simulink model "deltino"  (R2021b)
(part 8 of 10)

C = ft_4({phi_dot,psi_dot,t10,t100,t1000,t1001,t101,t1010,t1011,t1012,t1013,t1014,t1015,t1016,t1017,t1018,t1019,t102,t1020,t1021,t1022,t1023,t1024,t1025,t1026,t1027,t1028,t1029,t103,t1030,t1031,t1032,t1033,t1038,t1039,t104,t1040,t1041,t1042,t1043,t1044,t1045,t1046,t1047,t1048,t1049,t105,t1054,t1055,t1056,t1057,t1058,t1059,t1060,t1061,t1062,t1063,t1064,t1065,t1066,t1067,t1068,t1069,t1070,t1071,t1072,t1073,t1074,t1075,t1076,t1077,t1079,t1080,t1082,t1083,t1085,t1086,t1088,t1089,t1090,t1091,t1092,t1093,t1094,t1095,t1096,t1097,t1098,t1099,t11,t110,t1100,t1101,t1102,t1103,t1104,t1105,t1106,t1107,t1108,t1109,t111,t1110,t1111,t1112,t1113,t1114,t1115,t1116,t1117,t1118,t1119,t112,t1120,t1121,t1122,t1123,t1124,t1125,t1126,t1127,t1128,t1129,t113,t1130,t1131,t1132,t1133,t1134,t1135,t1136,t1137,t1138,t1139,t114,t1140,t1141,t1142,t1143,t1144,t1145,t1146,t1147,t1148,t1149,t115,t1150,t1151,t1152,t1153,t1154,t1155,t1156,t1157,t1158,t1159,t116,t1160,t1161,t1162,t1163,t1164,t1165,t1166,t1167,t1168,t1169,t117,t1170,t1171,t1172,t1173,t1175,t1176,t1177,t1178,t1179,t118,t1180,t1181,t1182,t1183,t1184,t1185,t1186,t1187,t1188,t119,t1190,t1191,t1193,t1194,t1195,t1196,t1197,t1198,t1199,t12,t120,t1200,t1201,t1202,t1203,t1204,t1205,t1206,t1207,t1208,t1209,t121,t1210,t1211,t1212,t1213,t1214,t122,t1223,t1224,t1225,t123,t1232,t1233,t1234,t1235,t1236,t1237,t1238,t1239,t124,t1240,t1241,t1242,t1243,t1244,t1245,t1246,t1247,t1248,t1249,t125,t1250,t1251,t1252,t1253,t1254,t1255,t1256,t1257,t1258,t1259,t126,t1260,t1261,t1262,t1263,t1264,t1265,t1266,t1267,t1268,t1269,t127,t1270,t1271,t1272,t1273,t1274,t1275,t1276,t1277,t1278,t1279,t128,t1280,t1281,t1282,t1283,t1284,t1285,t1286,t1287,t1288,t1289,t129,t1290,t1291,t1292,t1293,t1294,t1295,t1296,t1297,t1298,t1299,t13,t130,t1300,t1301,t1302,t1303,t1304,t1305,t1306,t1307,t1308,t1309,t131,t1310,t1311,t1312,t1313,t1314,t1315,t1316,t1317,t1318,t1319,t132,t1320,t1321,t1322,t1323,t1324,t1325,t1326,t1327,t1328,t1329,t133,t1330,t1331,t1332,t1335,t1337,t1338,t134,t1340,t1341,t1342,t1343,t1344,t1345,t1346,t1347,t1348,t1349,t135,t1350,t1351,t1352,t1353,t1354,t1355,t1356,t1357,t1358,t1359,t136,t1360,t1361,t1362,t1363,t1364,t1365,t1366,t1367,t1368,t1369,t1370,t1371,t138,t1384,t1385,t1386,t1387,t1388,t1389,t139,t1390,t1391,t1392,t1393,t1394,t1395,t1396,t1397,t1398,t1399,t14,t140,t1400,t1401,t1402,t1403,t1404,t1405,t1406,t1407,t1408,t1409,t141,t1410,t1411,t1412,t1413,t1414,t1415,t1416,t1417,t1418,t1419,t142,t1420,t1421,t1422,t1423,t1424,t1425,t1426,t1427,t1428,t1429,t143,t1430,t1431,t1432,t1433,t1434,t1435,t1436,t1437,t1438,t1439,t144,t1440,t1441,t1442,t1443,t1444,t1445,t1446,t1447,t145,t1458,t1459,t146,t1460,t1461,t1462,t1463,t1464,t1465,t1466,t1467,t1468,t1469,t147,t1470,t1471,t1472,t1473,t1474,t1475,t1476,t1477,t1478,t1479,t148,t1480,t1481,t1482,t1483,t1484,t1485,t1486,t1487,t1488,t1489,t149,t1490,t1491,t1492,t1493,t1494,t1495,t1496,t1497,t1498,t1499,t15,t150,t1501,t1502,t1504,t1505,t1507,t1508,t151,t1510,t1511,t1512,t1513,t1514,t1515,t152,t1524,t1525,t1526,t1527,t1528,t1529,t153,t1530,t1531,t1532,t1533,t1534,t1535,t1536,t1537,t1538,t1539,t154,t1541,t1542,t1543,t1544,t1545,t1546,t1547,t1548,t1549,t155,t1550,t1551,t1552,t1553,t1554,t1555,t1556,t1557,t1558,t1559,t156,t1560,t1561,t1562,t1563,t1564,t1565,t1566,t1567,t1568,t1569,t157,t1570,t1571,t1572,t1573,t1574,t1575,t1576,t1577,t1578,t1579,t158,t1580,t1581,t1582,t1583,t1584,t1585,t1586,t1587,t1588,t1589,t159,t1590,t1591,t1592,t1593,t1594,t1595,t1596,t1597,t1598,t1599,t16,t160,t1600,t1601,t1602,t1603,t1604,t1605,t1606,t1608,t1609,t161,t1610,t1611,t1612,t1613,t1614,t1615,t1616,t1617,t1618,t1619,t162,t1620,t1621,t1622,t1623,t1624,t1625,t1626,t1627,t1628,t1629,t163,t1630,t1631,t1632,t1633,t1634,t1635,t1636,t164,t1645,t165,t1651,t1652,t1653,t1654,t1655,t1656,t1657,t1658,t1659,t166,t1660,t1661,t1662,t1663,t1664,t1665,t1666,t1667,t1668,t1669,t167,t1670,t1671,t1672,t1673,t1674,t1675,t1676,t1677,t1678,t1679,t168,t1680,t1681,t1682,t1683,t1684,t1685,t1686,t1687,t1688,t1689,t169,t1690,t1691,t1692,t1693,t1694,t1695,t1696,t1697,t1698,t1699,t17,t170,t1700,t1701,t1702,t1703,t1704,t1705,t1706,t1707,t1708,t1709,t171,t1710,t1711,t1712,t1713,t1714,t1719,t172,t1720,t1721,t1722,t1723,t1724,t1725,t1726,t1727,t1728,t1729,t173,t1730,t1731,t1732,t1733,t1734,t1735,t1736,t1737,t1738,t1739,t174,t1740,t1741,t1742,t1743,t1744,t1745,t1746,t1747,t1748,t1749,t175,t1750,t1751,t1752,t1753,t1754,t1755,t1756,t1757,t1758,t176,t1760,t1762,t1764,t1766,t1767,t1768,t1769,t177,t1770,t1771,t1772,t1773,t1774,t1775,t1776,t1777,t1778,t1779,t178,t1780,t1781,t1782,t1783,t1784,t1785,t1786,t1787,t1788,t1789,t179,t1790,t1791,t1792,t1793,t1794,t1795,t1796,t1797,t1798,t1799,t18,t180,t1800,t1801,t1802,t1803,t1804,t1805,t1806,t1808,t1809,t181,t1810,t1811,t1812,t1813,t1814,t1815,t1816,t1817,t1818,t1819,t182,t1820,t1821,t1822,t1823,t1824,t1825,t1826,t1827,t1828,t1829,t183,t1830,t1831,t1833,t1835,t1837,t1839,t184,t1841,t1842,t1843,t1844,t1845,t1846,t1847,t1848,t1849,t185,t1850,t1851,t1852,t1853,t1854,t1855,t1856,t1865,t1866,t1867,t1868,t1869,t187,t1870,t1871,t1872,t1873,t1874,t1875,t1876,t1877,t1878,t1879,t188,t1880,t1881,t1882,t1883,t1884,t1885,t1886,t1887,t1888,t1889,t189,t1890,t1891,t1892,t1894,t1895,t1897,t19,t190,t1900,t1901,t1903,t1905,t1907,t191,t1917,t1918,t1919,t192,t1920,t1921,t1922,t1923,t1924,t1929,t193,t1930,t1931,t1932,t1933,t1934,t1935,t1936,t1937,t1938,t1939,t194,t1940,t1941,t1942,t1943,t1944,t1945,t1946,t1947,t1948,t195,t1950,t1951,t1952,t1953,t1954,t1955,t1956,t1957,t1958,t1959,t196,t1960,t1961,t1962,t1963,t1964,t1965,t1966,t1967,t1968,t1969,t197,t1978,t198,t1980,t1982,t1984,t1986,t1987,t1988,t1989,t199,t1990,t1991,t1992,t1993,t1994,t1995,t1996,t1997,t1998,t1999,t2,t20,t200,t2000,t2001,t2002,t2003,t2004,t2005,t2006,t2007,t2008,t2009,t201,t2010,t2011,t2012,t2013,t2014,t2015,t2016,t2017,t2018,t2019,t202,t2020,t2021,t2022,t2023,t2024,t2025,t2026,t2027,t2028,t2029,t203,t2030,t2031,t2032,t2033,t2034,t2035,t2036,t2037,t2038,t2039,t204,t2040,t2041,t2042,t2043,t2044,t2045,t2046,t2047,t2048,t2049,t205,t2050,t2051,t2052,t2053,t2054,t2055,t2056,t2057,t2058,t2059,t206,t2060,t2061,t2062,t2063,t2064,t2065,t207,t2075,t2076,t2077,t2078,t2079,t208,t2080,t2081,t2082,t2083,t2084,t2085,t2086,t2087,t2088,t2089,t209,t2090,t2091,t2092,t2093,t2094,t21,t210,t2100,t2101,t2102,t2103,t2104,t2105,t2106,t2107,t2108,t2109,t211,t2110,t2111,t2112,t2113,t2114,t2115,t212,t2124,t2125,t2126,t2127,t2128,t2129,t213,t2130,t2131,t214,t2140,t2141,t2142,t2143,t2144,t2145,t2146,t2147,t215,t2158,t2159,t216,t2160,t2161,t2162,t2163,t2164,t2165,t217,t218,t219,t22,t220,t221,t222,t223,t224,t225,t226,t227,t228,t229,t23,t230,t231,t232,t233,t234,t235,t24,t248,t249,t25,t250,t251,t252,t253,t254,t255,t256,t257,t258,t259,t26,t260,t261,t262,t263,t264,t266,t267,t268,t269,t27,t270,t271,t272,t273,t274,t275,t276,t277,t278,t279,t28,t280,t281,t282,t283,t284,t285,t286,t287,t288,t289,t29,t290,t291,t292,t293,t294,t295,t296,t297,t298,t299,t3,t30,t300,t301,t302,t303,t304,t305,t306,t307,t308,t309,t31,t310,t311,t312,t313,t314,t315,t316,t317,t318,t319,t320,t321,t322,t323,t324,t325,t326,t327,t328,t329,t330,t331,t332,t333,t334,t335,t336,t337,t338,t339,t340,t341,t342,t343,t344,t345,t346,t347,t348,t349,t350,t351,t352,t353,t354,t355,t356,t357,t358,t359,t360,t361,t362,t363,t364,t365,t366,t367,t368,t369,t370,t371,t372,t373,t374,t375,t376,t377,t378,t379,t380,t394,t395,t396,t397,t398,t399,t4,t400,t401,t402,t403,t404,t405,t406,t407,t408,t409,t410,t411,t412,t413,t414,t415,t416,t417,t418,t419,t420,t421,t422,t423,t424,t425,t426,t427,t428,t429,t430,t431,t432,t433,t434,t435,t436,t437,t438,t439,t440,t441,t442,t443,t444,t445,t446,t447,t448,t449,t450,t451,t452,t453,t454,t455,t456,t457,t458,t459,t46,t460,t461,t462,t463,t464,t465,t466,t467,t468,t469,t47,t470,t471,t472,t473,t474,t475,t476,t477,t478,t479,t48,t480,t481,t482,t483,t484,t485,t486,t487,t488,t489,t49,t490,t491,t492,t493,t494,t495,t496,t497,t498,t499,t5,t50,t500,t501,t503,t504,t506,t507,t509,t51,t510,t512,t513,t514,t515,t516,t517,t518,t519,t52,t520,t521,t522,t523,t524,t525,t526,t527,t528,t529,t53,t530,t531,t532,t533,t534,t535,t536,t537,t538,t539,t54,t540,t541,t542,t543,t544,t545,t546,t547,t548,t549,t55,t550,t551,t552,t553,t554,t555,t556,t557,t558,t559,t56,t560,t561,t562,t563,t564,t565,t566,t567,t568,t569,t57,t570,t571,t572,t573,t574,t575,t576,t577,t578,t579,t58,t580,t581,t582,t583,t584,t585,t586,t587,t588,t589,t59,t590,t591,t592,t593,t594,t595,t596,t597,t598,t599,t6,t60,t600,t601,t602,t603,t604,t605,t606,t607,t608,t609,t61,t610,t611,t612,t613,t614,t615,t616,t617,t618,t619,t62,t620,t621,t622,t623,t624,t625,t626,t627,t628,t629,t63,t630,t631,t632,t633,t634,t635,t636,t637,t638,t639,t64,t640,t641,t642,t643,t644,t645,t646,t647,t648,t649,t65,t650,t651,t652,t653,t654,t655,t656,t657,t658,t659,t66,t660,t661,t662,t663,t664,t665,t666,t667,t668,t669,t67,t670,t671,t672,t673,t674,t675,t676,t677,t678,t679,t68,t680,t681,t682,t683,t684,t685,t686,t687,t688,t689,t69,t690,t691,t692,t693,t694,t695,t696,t697,t698,t699,t7,t70,t700,t701,t702,t703,t704,t705,t706,t707,t708,t709,t71,t710,t711,t712,t713,t714,t715,t716,t717,t718,t719,t72,t720,t721,t722,t725,t726,t727,t728,t729,t73,t730,t731,t732,t733,t734,t735,t736,t737,t738,t739,t74,t740,t741,t742,t743,t744,t745,t746,t747,t748,t749,t75,t750,t751,t752,t753,t754,t755,t756,t757,t758,t759,t76,t760,t761,t762,t763,t764,t765,t766,t767,t768,t769,t77,t770,t771,t772,t773,t774,t775,t776,t777,t778,t779,t78,t780,t781,t782,t783,t784,t785,t786,t787,t788,t789,t79,t790,t791,t792,t793,t794,t795,t796,t797,t798,t799,t8,t80,t800,t801,t802,t803,t804,t805,t806,t807,t808,t809,t81,t810,t811,t812,t813,t814,t815,t816,t817,t818,t819,t82,t820,t821,t822,t823,t824,t825,t826,t827,t828,t83,t830,t831,t833,t834,t836,t837,t839,t84,t840,t841,t842,t843,t844,t845,t846,t847,t848,t849,t85,t850,t851,t852,t853,t856,t859,t86,t862,t865,t866,t867,t868,t869,t87,t872,t875,t877,t878,t879,t88,t880,t881,t882,t883,t884,t885,t886,t887,t888,t889,t89,t890,t891,t892,t893,t894,t895,t896,t897,t898,t899,t9,t90,t900,t901,t902,t903,t904,t905,t906,t907,t908,t909,t91,t910,t911,t912,t913,t914,t915,t916,t917,t918,t919,t92,t920,t921,t922,t923,t924,t925,t926,t927,t928,t929,t93,t930,t931,t932,t933,t934,t935,t936,t937,t938,t939,t94,t940,t941,t942,t943,t944,t945,t946,t947,t948,t949,t95,t950,t951,t952,t953,t954,t955,t956,t957,t958,t96,t960,t961,t962,t963,t964,t965,t966,t967,t968,t969,t97,t970,t971,t972,t973,t974,t975,t976,t977,t978,t979,t98,t980,t981,t982,t983,t984,t985,t986,t987,t989,t99,t994,t995,t996,t997,t998,t999,th11_dot,th12_dot,th13_dot,th21_dot,th22_dot,th23_dot,th31_dot,th32_dot,th33_dot,th41_dot,th42_dot,th43_dot,zeta_dot});
end
function C = ft_4(ct)
phi_dot = ct{1};
psi_dot = ct{2};
t10 = ct{3};
t100 = ct{4};
t1000 = ct{5};
t1001 = ct{6};
t101 = ct{7};
t1010 = ct{8};
t1011 = ct{9};
t1012 = ct{10};
t1013 = ct{11};
t1014 = ct{12};
t1015 = ct{13};
t1016 = ct{14};
t1017 = ct{15};
t1018 = ct{16};
t1019 = ct{17};
t102 = ct{18};
t1020 = ct{19};
t1021 = ct{20};
t1022 = ct{21};
t1023 = ct{22};
t1024 = ct{23};
t1025 = ct{24};
t1026 = ct{25};
t1027 = ct{26};
t1028 = ct{27};
t1029 = ct{28};
t103 = ct{29};
t1030 = ct{30};
t1031 = ct{31};
t1032 = ct{32};
t1033 = ct{33};
t1038 = ct{34};
t1039 = ct{35};
t104 = ct{36};
t1040 = ct{37};
t1041 = ct{38};
t1042 = ct{39};
t1043 = ct{40};
t1044 = ct{41};
t1045 = ct{42};
t1046 = ct{43};
t1047 = ct{44};
t1048 = ct{45};
t1049 = ct{46};
t105 = ct{47};
t1054 = ct{48};
t1055 = ct{49};
t1056 = ct{50};
t1057 = ct{51};
t1058 = ct{52};
t1059 = ct{53};
t1060 = ct{54};
t1061 = ct{55};
t1062 = ct{56};
t1063 = ct{57};
t1064 = ct{58};
t1065 = ct{59};
t1066 = ct{60};
t1067 = ct{61};
t1068 = ct{62};
t1069 = ct{63};
t1070 = ct{64};
t1071 = ct{65};
t1072 = ct{66};
t1073 = ct{67};
t1074 = ct{68};
t1075 = ct{69};
t1076 = ct{70};
t1077 = ct{71};
t1079 = ct{72};
t1080 = ct{73};
t1082 = ct{74};
t1083 = ct{75};
t1085 = ct{76};
t1086 = ct{77};
t1088 = ct{78};
t1089 = ct{79};
t1090 = ct{80};
t1091 = ct{81};
t1092 = ct{82};
t1093 = ct{83};
t1094 = ct{84};
t1095 = ct{85};
t1096 = ct{86};
t1097 = ct{87};
t1098 = ct{88};
t1099 = ct{89};
t11 = ct{90};
t110 = ct{91};
t1100 = ct{92};
t1101 = ct{93};
t1102 = ct{94};
t1103 = ct{95};
t1104 = ct{96};
t1105 = ct{97};
t1106 = ct{98};
t1107 = ct{99};
t1108 = ct{100};
t1109 = ct{101};
t111 = ct{102};
t1110 = ct{103};
t1111 = ct{104};
t1112 = ct{105};
t1113 = ct{106};
t1114 = ct{107};
t1115 = ct{108};
t1116 = ct{109};
t1117 = ct{110};
t1118 = ct{111};
t1119 = ct{112};
t112 = ct{113};
t1120 = ct{114};
t1121 = ct{115};
t1122 = ct{116};
t1123 = ct{117};
t1124 = ct{118};
t1125 = ct{119};
t1126 = ct{120};
t1127 = ct{121};
t1128 = ct{122};
t1129 = ct{123};
t113 = ct{124};
t1130 = ct{125};
t1131 = ct{126};
t1132 = ct{127};
t1133 = ct{128};
t1134 = ct{129};
t1135 = ct{130};
t1136 = ct{131};
t1137 = ct{132};
t1138 = ct{133};
t1139 = ct{134};
t114 = ct{135};
t1140 = ct{136};
t1141 = ct{137};
t1142 = ct{138};
t1143 = ct{139};
t1144 = ct{140};
t1145 = ct{141};
t1146 = ct{142};
t1147 = ct{143};
t1148 = ct{144};
t1149 = ct{145};
t115 = ct{146};
t1150 = ct{147};
t1151 = ct{148};
t1152 = ct{149};
t1153 = ct{150};
t1154 = ct{151};
t1155 = ct{152};
t1156 = ct{153};
t1157 = ct{154};
t1158 = ct{155};
t1159 = ct{156};
t116 = ct{157};
t1160 = ct{158};
t1161 = ct{159};
t1162 = ct{160};
t1163 = ct{161};
t1164 = ct{162};
t1165 = ct{163};
t1166 = ct{164};
t1167 = ct{165};
t1168 = ct{166};
t1169 = ct{167};
t117 = ct{168};
t1170 = ct{169};
t1171 = ct{170};
t1172 = ct{171};
t1173 = ct{172};
t1175 = ct{173};
t1176 = ct{174};
t1177 = ct{175};
t1178 = ct{176};
t1179 = ct{177};
t118 = ct{178};
t1180 = ct{179};
t1181 = ct{180};
t1182 = ct{181};
t1183 = ct{182};
t1184 = ct{183};
t1185 = ct{184};
t1186 = ct{185};
t1187 = ct{186};
t1188 = ct{187};
t119 = ct{188};
t1190 = ct{189};
t1191 = ct{190};
t1193 = ct{191};
t1194 = ct{192};
t1195 = ct{193};
t1196 = ct{194};
t1197 = ct{195};
t1198 = ct{196};
t1199 = ct{197};
t12 = ct{198};
t120 = ct{199};
t1200 = ct{200};
t1201 = ct{201};
t1202 = ct{202};
t1203 = ct{203};
t1204 = ct{204};
t1205 = ct{205};
t1206 = ct{206};
t1207 = ct{207};
t1208 = ct{208};
t1209 = ct{209};
t121 = ct{210};
t1210 = ct{211};
t1211 = ct{212};
t1212 = ct{213};
t1213 = ct{214};
t1214 = ct{215};
t122 = ct{216};
t1223 = ct{217};
t1224 = ct{218};
t1225 = ct{219};
t123 = ct{220};
t1232 = ct{221};
t1233 = ct{222};
t1234 = ct{223};
t1235 = ct{224};
t1236 = ct{225};
t1237 = ct{226};
t1238 = ct{227};
t1239 = ct{228};
t124 = ct{229};
t1240 = ct{230};
t1241 = ct{231};
t1242 = ct{232};
t1243 = ct{233};
t1244 = ct{234};
t1245 = ct{235};
t1246 = ct{236};
t1247 = ct{237};
t1248 = ct{238};
t1249 = ct{239};
t125 = ct{240};
t1250 = ct{241};
t1251 = ct{242};
t1252 = ct{243};
t1253 = ct{244};
t1254 = ct{245};
t1255 = ct{246};
t1256 = ct{247};
t1257 = ct{248};
t1258 = ct{249};
t1259 = ct{250};
t126 = ct{251};
t1260 = ct{252};
t1261 = ct{253};
t1262 = ct{254};
t1263 = ct{255};
t1264 = ct{256};
t1265 = ct{257};
t1266 = ct{258};
t1267 = ct{259};
t1268 = ct{260};
t1269 = ct{261};
t127 = ct{262};
t1270 = ct{263};
t1271 = ct{264};
t1272 = ct{265};
t1273 = ct{266};
t1274 = ct{267};
t1275 = ct{268};
t1276 = ct{269};
t1277 = ct{270};
t1278 = ct{271};
t1279 = ct{272};
t128 = ct{273};
t1280 = ct{274};
t1281 = ct{275};
t1282 = ct{276};
t1283 = ct{277};
t1284 = ct{278};
t1285 = ct{279};
t1286 = ct{280};
t1287 = ct{281};
t1288 = ct{282};
t1289 = ct{283};
t129 = ct{284};
t1290 = ct{285};
t1291 = ct{286};
t1292 = ct{287};
t1293 = ct{288};
t1294 = ct{289};
t1295 = ct{290};
t1296 = ct{291};
t1297 = ct{292};
t1298 = ct{293};
t1299 = ct{294};
t13 = ct{295};
t130 = ct{296};
t1300 = ct{297};
t1301 = ct{298};
t1302 = ct{299};
t1303 = ct{300};
t1304 = ct{301};
t1305 = ct{302};
t1306 = ct{303};
t1307 = ct{304};
t1308 = ct{305};
t1309 = ct{306};
t131 = ct{307};
t1310 = ct{308};
t1311 = ct{309};
t1312 = ct{310};
t1313 = ct{311};
t1314 = ct{312};
t1315 = ct{313};
t1316 = ct{314};
t1317 = ct{315};
t1318 = ct{316};
t1319 = ct{317};
t132 = ct{318};
t1320 = ct{319};
t1321 = ct{320};
t1322 = ct{321};
t1323 = ct{322};
t1324 = ct{323};
t1325 = ct{324};
t1326 = ct{325};
t1327 = ct{326};
t1328 = ct{327};
t1329 = ct{328};
t133 = ct{329};
t1330 = ct{330};
t1331 = ct{331};
t1332 = ct{332};
t1335 = ct{333};
t1337 = ct{334};
t1338 = ct{335};
t134 = ct{336};
t1340 = ct{337};
t1341 = ct{338};
t1342 = ct{339};
t1343 = ct{340};
t1344 = ct{341};
t1345 = ct{342};
t1346 = ct{343};
t1347 = ct{344};
t1348 = ct{345};
t1349 = ct{346};
t135 = ct{347};
t1350 = ct{348};
t1351 = ct{349};
t1352 = ct{350};
t1353 = ct{351};
t1354 = ct{352};
t1355 = ct{353};
t1356 = ct{354};
t1357 = ct{355};
t1358 = ct{356};
t1359 = ct{357};
t136 = ct{358};
t1360 = ct{359};
t1361 = ct{360};
t1362 = ct{361};
t1363 = ct{362};
t1364 = ct{363};
t1365 = ct{364};
t1366 = ct{365};
t1367 = ct{366};
t1368 = ct{367};
t1369 = ct{368};
t1370 = ct{369};
t1371 = ct{370};
t138 = ct{371};
t1384 = ct{372};
t1385 = ct{373};
t1386 = ct{374};
t1387 = ct{375};
t1388 = ct{376};
t1389 = ct{377};
t139 = ct{378};
t1390 = ct{379};
t1391 = ct{380};
t1392 = ct{381};
t1393 = ct{382};
t1394 = ct{383};
t1395 = ct{384};
t1396 = ct{385};
t1397 = ct{386};
t1398 = ct{387};
t1399 = ct{388};
t14 = ct{389};
t140 = ct{390};
t1400 = ct{391};
t1401 = ct{392};
t1402 = ct{393};
t1403 = ct{394};
t1404 = ct{395};
t1405 = ct{396};
t1406 = ct{397};
t1407 = ct{398};
t1408 = ct{399};
t1409 = ct{400};
t141 = ct{401};
t1410 = ct{402};
t1411 = ct{403};
t1412 = ct{404};
t1413 = ct{405};
t1414 = ct{406};
t1415 = ct{407};
t1416 = ct{408};
t1417 = ct{409};
t1418 = ct{410};
t1419 = ct{411};
t142 = ct{412};
t1420 = ct{413};
t1421 = ct{414};
t1422 = ct{415};
t1423 = ct{416};
t1424 = ct{417};
t1425 = ct{418};
t1426 = ct{419};
t1427 = ct{420};
t1428 = ct{421};
t1429 = ct{422};
t143 = ct{423};
t1430 = ct{424};
t1431 = ct{425};
t1432 = ct{426};
t1433 = ct{427};
t1434 = ct{428};
t1435 = ct{429};
t1436 = ct{430};
t1437 = ct{431};
t1438 = ct{432};
t1439 = ct{433};
t144 = ct{434};
t1440 = ct{435};
t1441 = ct{436};
t1442 = ct{437};
t1443 = ct{438};
t1444 = ct{439};
t1445 = ct{440};
t1446 = ct{441};
t1447 = ct{442};
t145 = ct{443};
t1458 = ct{444};
t1459 = ct{445};
t146 = ct{446};
t1460 = ct{447};
t1461 = ct{448};
t1462 = ct{449};
t1463 = ct{450};
t1464 = ct{451};
t1465 = ct{452};
t1466 = ct{453};
t1467 = ct{454};
t1468 = ct{455};
t1469 = ct{456};
t147 = ct{457};
t1470 = ct{458};
t1471 = ct{459};
t1472 = ct{460};
t1473 = ct{461};
t1474 = ct{462};
t1475 = ct{463};
t1476 = ct{464};
t1477 = ct{465};
t1478 = ct{466};
t1479 = ct{467};
t148 = ct{468};
t1480 = ct{469};
t1481 = ct{470};
t1482 = ct{471};
t1483 = ct{472};
t1484 = ct{473};
t1485 = ct{474};
t1486 = ct{475};
t1487 = ct{476};
t1488 = ct{477};
t1489 = ct{478};
t149 = ct{479};
t1490 = ct{480};
t1491 = ct{481};
t1492 = ct{482};
t1493 = ct{483};
t1494 = ct{484};
t1495 = ct{485};
t1496 = ct{486};
t1497 = ct{487};
t1498 = ct{488};
t1499 = ct{489};
t15 = ct{490};
t150 = ct{491};
t1501 = ct{492};
t1502 = ct{493};
t1504 = ct{494};
t1505 = ct{495};
t1507 = ct{496};
t1508 = ct{497};
t151 = ct{498};
t1510 = ct{499};
t1511 = ct{500};
t1512 = ct{501};
t1513 = ct{502};
t1514 = ct{503};
t1515 = ct{504};
t152 = ct{505};
t1524 = ct{506};
t1525 = ct{507};
t1526 = ct{508};
t1527 = ct{509};
t1528 = ct{510};
t1529 = ct{511};
t153 = ct{512};
t1530 = ct{513};
t1531 = ct{514};
t1532 = ct{515};
t1533 = ct{516};
t1534 = ct{517};
t1535 = ct{518};
t1536 = ct{519};
t1537 = ct{520};
t1538 = ct{521};
t1539 = ct{522};
t154 = ct{523};
t1541 = ct{524};
t1542 = ct{525};
t1543 = ct{526};
t1544 = ct{527};
t1545 = ct{528};
t1546 = ct{529};
t1547 = ct{530};
t1548 = ct{531};
t1549 = ct{532};
t155 = ct{533};
t1550 = ct{534};
t1551 = ct{535};
t1552 = ct{536};
t1553 = ct{537};
t1554 = ct{538};
t1555 = ct{539};
t1556 = ct{540};
t1557 = ct{541};
t1558 = ct{542};
t1559 = ct{543};
t156 = ct{544};
t1560 = ct{545};
t1561 = ct{546};
t1562 = ct{547};
t1563 = ct{548};
t1564 = ct{549};
t1565 = ct{550};
t1566 = ct{551};
t1567 = ct{552};
t1568 = ct{553};
t1569 = ct{554};
t157 = ct{555};
t1570 = ct{556};
t1571 = ct{557};
t1572 = ct{558};
t1573 = ct{559};
t1574 = ct{560};
t1575 = ct{561};
t1576 = ct{562};
t1577 = ct{563};
t1578 = ct{564};
t1579 = ct{565};
t158 = ct{566};
t1580 = ct{567};
t1581 = ct{568};
t1582 = ct{569};
t1583 = ct{570};
t1584 = ct{571};
t1585 = ct{572};
t1586 = ct{573};
t1587 = ct{574};
t1588 = ct{575};
t1589 = ct{576};
t159 = ct{577};
t1590 = ct{578};
t1591 = ct{579};
t1592 = ct{580};
t1593 = ct{581};
t1594 = ct{582};
t1595 = ct{583};
t1596 = ct{584};
t1597 = ct{585};
t1598 = ct{586};
t1599 = ct{587};
t16 = ct{588};
t160 = ct{589};
t1600 = ct{590};
t1601 = ct{591};
t1602 = ct{592};
t1603 = ct{593};
t1604 = ct{594};
t1605 = ct{595};
t1606 = ct{596};
t1608 = ct{597};
t1609 = ct{598};
t161 = ct{599};
t1610 = ct{600};
t1611 = ct{601};
t1612 = ct{602};
t1613 = ct{603};
t1614 = ct{604};
t1615 = ct{605};
t1616 = ct{606};
t1617 = ct{607};
t1618 = ct{608};
t1619 = ct{609};
t162 = ct{610};
t1620 = ct{611};
t1621 = ct{612};
t1622 = ct{613};
t1623 = ct{614};
t1624 = ct{615};
t1625 = ct{616};
t1626 = ct{617};
t1627 = ct{618};
t1628 = ct{619};
t1629 = ct{620};
t163 = ct{621};
t1630 = ct{622};
t1631 = ct{623};
t1632 = ct{624};
t1633 = ct{625};
t1634 = ct{626};
t1635 = ct{627};
t1636 = ct{628};
t164 = ct{629};
t1645 = ct{630};
t165 = ct{631};
t1651 = ct{632};
t1652 = ct{633};
t1653 = ct{634};
t1654 = ct{635};
t1655 = ct{636};
t1656 = ct{637};
t1657 = ct{638};
t1658 = ct{639};
t1659 = ct{640};
t166 = ct{641};
t1660 = ct{642};
t1661 = ct{643};
t1662 = ct{644};
t1663 = ct{645};
t1664 = ct{646};
t1665 = ct{647};
t1666 = ct{648};
t1667 = ct{649};
t1668 = ct{650};
t1669 = ct{651};
t167 = ct{652};
t1670 = ct{653};
t1671 = ct{654};
t1672 = ct{655};
t1673 = ct{656};
t1674 = ct{657};
t1675 = ct{658};
t1676 = ct{659};
t1677 = ct{660};
t1678 = ct{661};
t1679 = ct{662};
t168 = ct{663};
t1680 = ct{664};
t1681 = ct{665};
t1682 = ct{666};
t1683 = ct{667};
t1684 = ct{668};
t1685 = ct{669};
t1686 = ct{670};
t1687 = ct{671};
t1688 = ct{672};
t1689 = ct{673};
t169 = ct{674};
t1690 = ct{675};
t1691 = ct{676};
t1692 = ct{677};
t1693 = ct{678};
t1694 = ct{679};
t1695 = ct{680};
t1696 = ct{681};
t1697 = ct{682};
t1698 = ct{683};
t1699 = ct{684};
t17 = ct{685};
t170 = ct{686};
t1700 = ct{687};
t1701 = ct{688};
t1702 = ct{689};
t1703 = ct{690};
t1704 = ct{691};
t1705 = ct{692};
t1706 = ct{693};
t1707 = ct{694};
t1708 = ct{695};
t1709 = ct{696};
t171 = ct{697};
t1710 = ct{698};
t1711 = ct{699};
t1712 = ct{700};
t1713 = ct{701};
t1714 = ct{702};
t1719 = ct{703};
t172 = ct{704};
t1720 = ct{705};
t1721 = ct{706};
t1722 = ct{707};
t1723 = ct{708};
t1724 = ct{709};
t1725 = ct{710};
t1726 = ct{711};
t1727 = ct{712};
t1728 = ct{713};
t1729 = ct{714};
t173 = ct{715};
t1730 = ct{716};
t1731 = ct{717};
t1732 = ct{718};
t1733 = ct{719};
t1734 = ct{720};
t1735 = ct{721};
t1736 = ct{722};
t1737 = ct{723};
t1738 = ct{724};
t1739 = ct{725};
t174 = ct{726};
t1740 = ct{727};
t1741 = ct{728};
t1742 = ct{729};
t1743 = ct{730};
t1744 = ct{731};
t1745 = ct{732};
t1746 = ct{733};
t1747 = ct{734};
t1748 = ct{735};
t1749 = ct{736};
t175 = ct{737};
t1750 = ct{738};
t1751 = ct{739};
t1752 = ct{740};
t1753 = ct{741};
t1754 = ct{742};
t1755 = ct{743};
t1756 = ct{744};
t1757 = ct{745};
t1758 = ct{746};
t176 = ct{747};
t1760 = ct{748};
t1762 = ct{749};
t1764 = ct{750};
t1766 = ct{751};
t1767 = ct{752};
t1768 = ct{753};
t1769 = ct{754};
t177 = ct{755};
t1770 = ct{756};
t1771 = ct{757};
t1772 = ct{758};
t1773 = ct{759};
t1774 = ct{760};
t1775 = ct{761};
t1776 = ct{762};
t1777 = ct{763};
t1778 = ct{764};
t1779 = ct{765};
t178 = ct{766};
t1780 = ct{767};
t1781 = ct{768};
t1782 = ct{769};
t1783 = ct{770};
t1784 = ct{771};
t1785 = ct{772};
t1786 = ct{773};
t1787 = ct{774};
t1788 = ct{775};
t1789 = ct{776};
t179 = ct{777};
t1790 = ct{778};
t1791 = ct{779};
t1792 = ct{780};
t1793 = ct{781};
t1794 = ct{782};
t1795 = ct{783};
t1796 = ct{784};
t1797 = ct{785};
t1798 = ct{786};
t1799 = ct{787};
t18 = ct{788};
t180 = ct{789};
t1800 = ct{790};
t1801 = ct{791};
t1802 = ct{792};
t1803 = ct{793};
t1804 = ct{794};
t1805 = ct{795};
t1806 = ct{796};
t1808 = ct{797};
t1809 = ct{798};
t181 = ct{799};
t1810 = ct{800};
t1811 = ct{801};
t1812 = ct{802};
t1813 = ct{803};
t1814 = ct{804};
t1815 = ct{805};
t1816 = ct{806};
t1817 = ct{807};
t1818 = ct{808};
t1819 = ct{809};
t182 = ct{810};
t1820 = ct{811};
t1821 = ct{812};
t1822 = ct{813};
t1823 = ct{814};
t1824 = ct{815};
t1825 = ct{816};
t1826 = ct{817};
t1827 = ct{818};
t1828 = ct{819};
t1829 = ct{820};
t183 = ct{821};
t1830 = ct{822};
t1831 = ct{823};
t1833 = ct{824};
t1835 = ct{825};
t1837 = ct{826};
t1839 = ct{827};
t184 = ct{828};
t1841 = ct{829};
t1842 = ct{830};
t1843 = ct{831};
t1844 = ct{832};
t1845 = ct{833};
t1846 = ct{834};
t1847 = ct{835};
t1848 = ct{836};
t1849 = ct{837};
t185 = ct{838};
t1850 = ct{839};
t1851 = ct{840};
t1852 = ct{841};
t1853 = ct{842};
t1854 = ct{843};
t1855 = ct{844};
t1856 = ct{845};
t1865 = ct{846};
t1866 = ct{847};
t1867 = ct{848};
t1868 = ct{849};
t1869 = ct{850};
t187 = ct{851};
t1870 = ct{852};
t1871 = ct{853};
t1872 = ct{854};
t1873 = ct{855};
t1874 = ct{856};
t1875 = ct{857};
t1876 = ct{858};
t1877 = ct{859};
t1878 = ct{860};
t1879 = ct{861};
t188 = ct{862};
t1880 = ct{863};
t1881 = ct{864};
t1882 = ct{865};
t1883 = ct{866};
t1884 = ct{867};
t1885 = ct{868};
t1886 = ct{869};
t1887 = ct{870};
t1888 = ct{871};
t1889 = ct{872};
t189 = ct{873};
t1890 = ct{874};
t1891 = ct{875};
t1892 = ct{876};
t1894 = ct{877};
t1895 = ct{878};
t1897 = ct{879};
t19 = ct{880};
t190 = ct{881};
t1900 = ct{882};
t1901 = ct{883};
t1903 = ct{884};
t1905 = ct{885};
t1907 = ct{886};
t191 = ct{887};
t1917 = ct{888};
t1918 = ct{889};
t1919 = ct{890};
t192 = ct{891};
t1920 = ct{892};
t1921 = ct{893};
t1922 = ct{894};
t1923 = ct{895};
t1924 = ct{896};
t1929 = ct{897};
t193 = ct{898};
t1930 = ct{899};
t1931 = ct{900};
t1932 = ct{901};
t1933 = ct{902};
t1934 = ct{903};
t1935 = ct{904};
t1936 = ct{905};
t1937 = ct{906};
t1938 = ct{907};
t1939 = ct{908};
t194 = ct{909};
t1940 = ct{910};
t1941 = ct{911};
t1942 = ct{912};
t1943 = ct{913};
t1944 = ct{914};
t1945 = ct{915};
t1946 = ct{916};
t1947 = ct{917};
t1948 = ct{918};
t195 = ct{919};
t1950 = ct{920};
t1951 = ct{921};
t1952 = ct{922};
t1953 = ct{923};
t1954 = ct{924};
t1955 = ct{925};
t1956 = ct{926};
t1957 = ct{927};
t1958 = ct{928};
t1959 = ct{929};
t196 = ct{930};
t1960 = ct{931};
t1961 = ct{932};
t1962 = ct{933};
t1963 = ct{934};
t1964 = ct{935};
t1965 = ct{936};
t1966 = ct{937};
t1967 = ct{938};
t1968 = ct{939};
t1969 = ct{940};
t197 = ct{941};
t1978 = ct{942};
t198 = ct{943};
t1980 = ct{944};
t1982 = ct{945};
t1984 = ct{946};
t1986 = ct{947};
t1987 = ct{948};
t1988 = ct{949};
t1989 = ct{950};
t199 = ct{951};
t1990 = ct{952};
t1991 = ct{953};
t1992 = ct{954};
t1993 = ct{955};
t1994 = ct{956};
t1995 = ct{957};
t1996 = ct{958};
t1997 = ct{959};
t1998 = ct{960};
t1999 = ct{961};
t2 = ct{962};
t20 = ct{963};
t200 = ct{964};
t2000 = ct{965};
t2001 = ct{966};
t2002 = ct{967};
t2003 = ct{968};
t2004 = ct{969};
t2005 = ct{970};
t2006 = ct{971};
t2007 = ct{972};
t2008 = ct{973};
t2009 = ct{974};
t201 = ct{975};
t2010 = ct{976};
t2011 = ct{977};
t2012 = ct{978};
t2013 = ct{979};
t2014 = ct{980};
t2015 = ct{981};
t2016 = ct{982};
t2017 = ct{983};
t2018 = ct{984};
t2019 = ct{985};
t202 = ct{986};
t2020 = ct{987};
t2021 = ct{988};
t2022 = ct{989};
t2023 = ct{990};
t2024 = ct{991};
t2025 = ct{992};
t2026 = ct{993};
t2027 = ct{994};
t2028 = ct{995};
t2029 = ct{996};
t203 = ct{997};
t2030 = ct{998};
t2031 = ct{999};
t2032 = ct{1000};
t2033 = ct{1001};
t2034 = ct{1002};
t2035 = ct{1003};
t2036 = ct{1004};
t2037 = ct{1005};
t2038 = ct{1006};
t2039 = ct{1007};
t204 = ct{1008};
t2040 = ct{1009};
t2041 = ct{1010};
t2042 = ct{1011};
t2043 = ct{1012};
t2044 = ct{1013};
t2045 = ct{1014};
t2046 = ct{1015};
t2047 = ct{1016};
t2048 = ct{1017};
t2049 = ct{1018};
t205 = ct{1019};
t2050 = ct{1020};
t2051 = ct{1021};
t2052 = ct{1022};
t2053 = ct{1023};
t2054 = ct{1024};
t2055 = ct{1025};
t2056 = ct{1026};
t2057 = ct{1027};
t2058 = ct{1028};
t2059 = ct{1029};
t206 = ct{1030};
t2060 = ct{1031};
t2061 = ct{1032};
t2062 = ct{1033};
t2063 = ct{1034};
t2064 = ct{1035};
t2065 = ct{1036};
t207 = ct{1037};
t2075 = ct{1038};
t2076 = ct{1039};
t2077 = ct{1040};
t2078 = ct{1041};
t2079 = ct{1042};
t208 = ct{1043};
t2080 = ct{1044};
t2081 = ct{1045};
t2082 = ct{1046};
t2083 = ct{1047};
t2084 = ct{1048};
t2085 = ct{1049};
t2086 = ct{1050};
t2087 = ct{1051};
t2088 = ct{1052};
t2089 = ct{1053};
t209 = ct{1054};
t2090 = ct{1055};
t2091 = ct{1056};
t2092 = ct{1057};
t2093 = ct{1058};
t2094 = ct{1059};
t21 = ct{1060};
t210 = ct{1061};
t2100 = ct{1062};
t2101 = ct{1063};
t2102 = ct{1064};
t2103 = ct{1065};
t2104 = ct{1066};
t2105 = ct{1067};
t2106 = ct{1068};
t2107 = ct{1069};
t2108 = ct{1070};
t2109 = ct{1071};
t211 = ct{1072};
t2110 = ct{1073};
t2111 = ct{1074};
t2112 = ct{1075};
t2113 = ct{1076};
t2114 = ct{1077};
t2115 = ct{1078};
t212 = ct{1079};
t2124 = ct{1080};
t2125 = ct{1081};
t2126 = ct{1082};
t2127 = ct{1083};
t2128 = ct{1084};
t2129 = ct{1085};
t213 = ct{1086};
t2130 = ct{1087};
t2131 = ct{1088};
t214 = ct{1089};
t2140 = ct{1090};
t2141 = ct{1091};
t2142 = ct{1092};
t2143 = ct{1093};
t2144 = ct{1094};
t2145 = ct{1095};
t2146 = ct{1096};
t2147 = ct{1097};
t215 = ct{1098};
t2158 = ct{1099};
t2159 = ct{1100};
t216 = ct{1101};
t2160 = ct{1102};
t2161 = ct{1103};
t2162 = ct{1104};
t2163 = ct{1105};
t2164 = ct{1106};
t2165 = ct{1107};
t217 = ct{1108};
t218 = ct{1109};
t219 = ct{1110};
t22 = ct{1111};
t220 = ct{1112};
t221 = ct{1113};
t222 = ct{1114};
t223 = ct{1115};
t224 = ct{1116};
t225 = ct{1117};
t226 = ct{1118};
t227 = ct{1119};
t228 = ct{1120};
t229 = ct{1121};
t23 = ct{1122};
t230 = ct{1123};
t231 = ct{1124};
t232 = ct{1125};
t233 = ct{1126};
t234 = ct{1127};
t235 = ct{1128};
t24 = ct{1129};
t248 = ct{1130};
t249 = ct{1131};
t25 = ct{1132};
t250 = ct{1133};
t251 = ct{1134};
t252 = ct{1135};
t253 = ct{1136};
t254 = ct{1137};
t255 = ct{1138};
t256 = ct{1139};
t257 = ct{1140};
t258 = ct{1141};
t259 = ct{1142};
t26 = ct{1143};
t260 = ct{1144};
t261 = ct{1145};
t262 = ct{1146};
t263 = ct{1147};
t264 = ct{1148};
t266 = ct{1149};
t267 = ct{1150};
t268 = ct{1151};
t269 = ct{1152};
t27 = ct{1153};
t270 = ct{1154};
t271 = ct{1155};
t272 = ct{1156};
t273 = ct{1157};
t274 = ct{1158};
t275 = ct{1159};
t276 = ct{1160};
t277 = ct{1161};
t278 = ct{1162};
t279 = ct{1163};
t28 = ct{1164};
t280 = ct{1165};
t281 = ct{1166};
t282 = ct{1167};
t283 = ct{1168};
t284 = ct{1169};
t285 = ct{1170};
t286 = ct{1171};
t287 = ct{1172};
t288 = ct{1173};
t289 = ct{1174};
t29 = ct{1175};
t290 = ct{1176};
t291 = ct{1177};
t292 = ct{1178};
t293 = ct{1179};
t294 = ct{1180};
t295 = ct{1181};
t296 = ct{1182};
t297 = ct{1183};
t298 = ct{1184};
t299 = ct{1185};
t3 = ct{1186};
t30 = ct{1187};
t300 = ct{1188};
t301 = ct{1189};
t302 = ct{1190};
t303 = ct{1191};
t304 = ct{1192};
t305 = ct{1193};
t306 = ct{1194};
t307 = ct{1195};
t308 = ct{1196};
t309 = ct{1197};
t31 = ct{1198};
t310 = ct{1199};
t311 = ct{1200};
t312 = ct{1201};
t313 = ct{1202};
t314 = ct{1203};
t315 = ct{1204};
t316 = ct{1205};
t317 = ct{1206};
t318 = ct{1207};
t319 = ct{1208};
t320 = ct{1209};
t321 = ct{1210};
t322 = ct{1211};
t323 = ct{1212};
t324 = ct{1213};
t325 = ct{1214};
t326 = ct{1215};
t327 = ct{1216};
t328 = ct{1217};
t329 = ct{1218};
t330 = ct{1219};
t331 = ct{1220};
t332 = ct{1221};
t333 = ct{1222};
t334 = ct{1223};
t335 = ct{1224};
t336 = ct{1225};
t337 = ct{1226};
t338 = ct{1227};
t339 = ct{1228};
t340 = ct{1229};
t341 = ct{1230};
t342 = ct{1231};
t343 = ct{1232};
t344 = ct{1233};
t345 = ct{1234};
t346 = ct{1235};
t347 = ct{1236};
t348 = ct{1237};
t349 = ct{1238};
t350 = ct{1239};
t351 = ct{1240};
t352 = ct{1241};
t353 = ct{1242};
t354 = ct{1243};
t355 = ct{1244};
t356 = ct{1245};
t357 = ct{1246};
t358 = ct{1247};
t359 = ct{1248};
t360 = ct{1249};
t361 = ct{1250};
t362 = ct{1251};
t363 = ct{1252};
t364 = ct{1253};
t365 = ct{1254};
t366 = ct{1255};
t367 = ct{1256};
t368 = ct{1257};
t369 = ct{1258};
t370 = ct{1259};
t371 = ct{1260};
t372 = ct{1261};
t373 = ct{1262};
t374 = ct{1263};
t375 = ct{1264};
t376 = ct{1265};
t377 = ct{1266};
t378 = ct{1267};
t379 = ct{1268};
t380 = ct{1269};
t394 = ct{1270};
t395 = ct{1271};
t396 = ct{1272};
t397 = ct{1273};
t398 = ct{1274};
t399 = ct{1275};
t4 = ct{1276};
t400 = ct{1277};
t401 = ct{1278};
t402 = ct{1279};
t403 = ct{1280};
t404 = ct{1281};
t405 = ct{1282};
t406 = ct{1283};
t407 = ct{1284};
t408 = ct{1285};
t409 = ct{1286};
t410 = ct{1287};
t411 = ct{1288};
t412 = ct{1289};
t413 = ct{1290};
t414 = ct{1291};
t415 = ct{1292};
t416 = ct{1293};
t417 = ct{1294};
t418 = ct{1295};
t419 = ct{1296};
t420 = ct{1297};
t421 = ct{1298};
t422 = ct{1299};
t423 = ct{1300};
t424 = ct{1301};
t425 = ct{1302};
t426 = ct{1303};
t427 = ct{1304};
t428 = ct{1305};
t429 = ct{1306};
t430 = ct{1307};
t431 = ct{1308};
t432 = ct{1309};
t433 = ct{1310};
t434 = ct{1311};
t435 = ct{1312};
t436 = ct{1313};
t437 = ct{1314};
t438 = ct{1315};
t439 = ct{1316};
t440 = ct{1317};
t441 = ct{1318};
t442 = ct{1319};
t443 = ct{1320};
t444 = ct{1321};
t445 = ct{1322};
t446 = ct{1323};
t447 = ct{1324};
t448 = ct{1325};
t449 = ct{1326};
t450 = ct{1327};
t451 = ct{1328};
t452 = ct{1329};
t453 = ct{1330};
t454 = ct{1331};
t455 = ct{1332};
t456 = ct{1333};
t457 = ct{1334};
t458 = ct{1335};
t459 = ct{1336};
t46 = ct{1337};
t460 = ct{1338};
t461 = ct{1339};
t462 = ct{1340};
t463 = ct{1341};
t464 = ct{1342};
t465 = ct{1343};
t466 = ct{1344};
t467 = ct{1345};
t468 = ct{1346};
t469 = ct{1347};
t47 = ct{1348};
t470 = ct{1349};
t471 = ct{1350};
t472 = ct{1351};
t473 = ct{1352};
t474 = ct{1353};
t475 = ct{1354};
t476 = ct{1355};
t477 = ct{1356};
t478 = ct{1357};
t479 = ct{1358};
t48 = ct{1359};
t480 = ct{1360};
t481 = ct{1361};
t482 = ct{1362};
t483 = ct{1363};
t484 = ct{1364};
t485 = ct{1365};
t486 = ct{1366};
t487 = ct{1367};
t488 = ct{1368};
t489 = ct{1369};
t49 = ct{1370};
t490 = ct{1371};
t491 = ct{1372};
t492 = ct{1373};
t493 = ct{1374};
t494 = ct{1375};
t495 = ct{1376};
t496 = ct{1377};
t497 = ct{1378};
t498 = ct{1379};
t499 = ct{1380};
t5 = ct{1381};
t50 = ct{1382};
t500 = ct{1383};
t501 = ct{1384};
t503 = ct{1385};
t504 = ct{1386};
t506 = ct{1387};
t507 = ct{1388};
t509 = ct{1389};
t51 = ct{1390};
t510 = ct{1391};
t512 = ct{1392};
t513 = ct{1393};
t514 = ct{1394};
t515 = ct{1395};
t516 = ct{1396};
t517 = ct{1397};
t518 = ct{1398};
t519 = ct{1399};
t52 = ct{1400};
t520 = ct{1401};
t521 = ct{1402};
t522 = ct{1403};
t523 = ct{1404};
t524 = ct{1405};
t525 = ct{1406};
t526 = ct{1407};
t527 = ct{1408};
t528 = ct{1409};
t529 = ct{1410};
t53 = ct{1411};
t530 = ct{1412};
t531 = ct{1413};
t532 = ct{1414};
t533 = ct{1415};
t534 = ct{1416};
t535 = ct{1417};
t536 = ct{1418};
t537 = ct{1419};
t538 = ct{1420};
t539 = ct{1421};
t54 = ct{1422};
t540 = ct{1423};
t541 = ct{1424};
t542 = ct{1425};
t543 = ct{1426};
t544 = ct{1427};
t545 = ct{1428};
t546 = ct{1429};
t547 = ct{1430};
t548 = ct{1431};
t549 = ct{1432};
t55 = ct{1433};
t550 = ct{1434};
t551 = ct{1435};
t552 = ct{1436};
t553 = ct{1437};
t554 = ct{1438};
t555 = ct{1439};
t556 = ct{1440};
t557 = ct{1441};
t558 = ct{1442};
t559 = ct{1443};
t56 = ct{1444};
t560 = ct{1445};
t561 = ct{1446};
t562 = ct{1447};
t563 = ct{1448};
t564 = ct{1449};
t565 = ct{1450};
t566 = ct{1451};
t567 = ct{1452};
t568 = ct{1453};
t569 = ct{1454};
t57 = ct{1455};
t570 = ct{1456};
t571 = ct{1457};
t572 = ct{1458};
t573 = ct{1459};
t574 = ct{1460};
t575 = ct{1461};
t576 = ct{1462};
t577 = ct{1463};
t578 = ct{1464};
t579 = ct{1465};
t58 = ct{1466};
t580 = ct{1467};
t581 = ct{1468};
t582 = ct{1469};
t583 = ct{1470};
t584 = ct{1471};
t585 = ct{1472};
t586 = ct{1473};
t587 = ct{1474};
t588 = ct{1475};
t589 = ct{1476};
t59 = ct{1477};
t590 = ct{1478};
t591 = ct{1479};
t592 = ct{1480};
t593 = ct{1481};
t594 = ct{1482};
t595 = ct{1483};
t596 = ct{1484};
t597 = ct{1485};
t598 = ct{1486};
t599 = ct{1487};
t6 = ct{1488};
t60 = ct{1489};
t600 = ct{1490};
t601 = ct{1491};
t602 = ct{1492};
t603 = ct{1493};
t604 = ct{1494};
t605 = ct{1495};
t606 = ct{1496};
t607 = ct{1497};
t608 = ct{1498};
t609 = ct{1499};
t61 = ct{1500};
t610 = ct{1501};
t611 = ct{1502};
t612 = ct{1503};
t613 = ct{1504};
t614 = ct{1505};
t615 = ct{1506};
t616 = ct{1507};
t617 = ct{1508};
t618 = ct{1509};
t619 = ct{1510};
t62 = ct{1511};
t620 = ct{1512};
t621 = ct{1513};
t622 = ct{1514};
t623 = ct{1515};
t624 = ct{1516};
t625 = ct{1517};
t626 = ct{1518};
t627 = ct{1519};
t628 = ct{1520};
t629 = ct{1521};
t63 = ct{1522};
t630 = ct{1523};
t631 = ct{1524};
t632 = ct{1525};
t633 = ct{1526};
t634 = ct{1527};
t635 = ct{1528};
t636 = ct{1529};
t637 = ct{1530};
t638 = ct{1531};
t639 = ct{1532};
t64 = ct{1533};
t640 = ct{1534};
t641 = ct{1535};
t642 = ct{1536};
t643 = ct{1537};
t644 = ct{1538};
t645 = ct{1539};
t646 = ct{1540};
t647 = ct{1541};
t648 = ct{1542};
t649 = ct{1543};
t65 = ct{1544};
t650 = ct{1545};
t651 = ct{1546};
t652 = ct{1547};
t653 = ct{1548};
t654 = ct{1549};
t655 = ct{1550};
t656 = ct{1551};
t657 = ct{1552};
t658 = ct{1553};
t659 = ct{1554};
t66 = ct{1555};
t660 = ct{1556};
t661 = ct{1557};
t662 = ct{1558};
t663 = ct{1559};
t664 = ct{1560};
t665 = ct{1561};
t666 = ct{1562};
t667 = ct{1563};
t668 = ct{1564};
t669 = ct{1565};
t67 = ct{1566};
t670 = ct{1567};
t671 = ct{1568};
t672 = ct{1569};
t673 = ct{1570};
t674 = ct{1571};
t675 = ct{1572};
t676 = ct{1573};
t677 = ct{1574};
t678 = ct{1575};
t679 = ct{1576};
t68 = ct{1577};
t680 = ct{1578};
t681 = ct{1579};
t682 = ct{1580};
t683 = ct{1581};
t684 = ct{1582};
t685 = ct{1583};
t686 = ct{1584};
t687 = ct{1585};
t688 = ct{1586};
t689 = ct{1587};
t69 = ct{1588};
t690 = ct{1589};
t691 = ct{1590};
t692 = ct{1591};
t693 = ct{1592};
t694 = ct{1593};
t695 = ct{1594};
t696 = ct{1595};
t697 = ct{1596};
t698 = ct{1597};
t699 = ct{1598};
t7 = ct{1599};
t70 = ct{1600};
t700 = ct{1601};
t701 = ct{1602};
t702 = ct{1603};
t703 = ct{1604};
t704 = ct{1605};
t705 = ct{1606};
t706 = ct{1607};
t707 = ct{1608};
t708 = ct{1609};
t709 = ct{1610};
t71 = ct{1611};
t710 = ct{1612};
t711 = ct{1613};
t712 = ct{1614};
t713 = ct{1615};
t714 = ct{1616};
t715 = ct{1617};
t716 = ct{1618};
t717 = ct{1619};
t718 = ct{1620};
t719 = ct{1621};
t72 = ct{1622};
t720 = ct{1623};
t721 = ct{1624};
t722 = ct{1625};
t725 = ct{1626};
t726 = ct{1627};
t727 = ct{1628};
t728 = ct{1629};
t729 = ct{1630};
t73 = ct{1631};
t730 = ct{1632};
t731 = ct{1633};
t732 = ct{1634};
t733 = ct{1635};
t734 = ct{1636};
t735 = ct{1637};
t736 = ct{1638};
t737 = ct{1639};
t738 = ct{1640};
t739 = ct{1641};
t74 = ct{1642};
t740 = ct{1643};
t741 = ct{1644};
t742 = ct{1645};
t743 = ct{1646};
t744 = ct{1647};
t745 = ct{1648};
t746 = ct{1649};
t747 = ct{1650};
t748 = ct{1651};
t749 = ct{1652};
t75 = ct{1653};
t750 = ct{1654};
t751 = ct{1655};
t752 = ct{1656};
t753 = ct{1657};
t754 = ct{1658};
t755 = ct{1659};
t756 = ct{1660};
t757 = ct{1661};
t758 = ct{1662};
t759 = ct{1663};
t76 = ct{1664};
t760 = ct{1665};
t761 = ct{1666};
t762 = ct{1667};
t763 = ct{1668};
t764 = ct{1669};
t765 = ct{1670};
t766 = ct{1671};
t767 = ct{1672};
t768 = ct{1673};
t769 = ct{1674};
t77 = ct{1675};
t770 = ct{1676};
t771 = ct{1677};
t772 = ct{1678};
t773 = ct{1679};
t774 = ct{1680};
t775 = ct{1681};
t776 = ct{1682};
t777 = ct{1683};
t778 = ct{1684};
t779 = ct{1685};
t78 = ct{1686};
t780 = ct{1687};
t781 = ct{1688};
t782 = ct{1689};
t783 = ct{1690};
t784 = ct{1691};
t785 = ct{1692};
t786 = ct{1693};
t787 = ct{1694};
t788 = ct{1695};
t789 = ct{1696};
t79 = ct{1697};
t790 = ct{1698};
t791 = ct{1699};
t792 = ct{1700};
t793 = ct{1701};
t794 = ct{1702};
t795 = ct{1703};
t796 = ct{1704};
t797 = ct{1705};
t798 = ct{1706};
t799 = ct{1707};
t8 = ct{1708};
t80 = ct{1709};
t800 = ct{1710};
t801 = ct{1711};
t802 = ct{1712};
t803 = ct{1713};
t804 = ct{1714};
t805 = ct{1715};
t806 = ct{1716};
t807 = ct{1717};
t808 = ct{1718};
t809 = ct{1719};
t81 = ct{1720};
t810 = ct{1721};
t811 = ct{1722};
t812 = ct{1723};
t813 = ct{1724};
t814 = ct{1725};
t815 = ct{1726};
t816 = ct{1727};
t817 = ct{1728};
t818 = ct{1729};
t819 = ct{1730};
t82 = ct{1731};
t820 = ct{1732};
t821 = ct{1733};
t822 = ct{1734};
t823 = ct{1735};
t824 = ct{1736};
t825 = ct{1737};
t826 = ct{1738};
t827 = ct{1739};
t828 = ct{1740};
t83 = ct{1741};
t830 = ct{1742};
t831 = ct{1743};
t833 = ct{1744};
t834 = ct{1745};
t836 = ct{1746};
t837 = ct{1747};
t839 = ct{1748};
t84 = ct{1749};
t840 = ct{1750};
t841 = ct{1751};
t842 = ct{1752};
t843 = ct{1753};
t844 = ct{1754};
t845 = ct{1755};
t846 = ct{1756};
t847 = ct{1757};
t848 = ct{1758};
t849 = ct{1759};
t85 = ct{1760};
t850 = ct{1761};
t851 = ct{1762};
t852 = ct{1763};
t853 = ct{1764};
t856 = ct{1765};
t859 = ct{1766};
t86 = ct{1767};
t862 = ct{1768};
t865 = ct{1769};
t866 = ct{1770};
t867 = ct{1771};
t868 = ct{1772};
t869 = ct{1773};
t87 = ct{1774};
t872 = ct{1775};
t875 = ct{1776};
t877 = ct{1777};
t878 = ct{1778};
t879 = ct{1779};
t88 = ct{1780};
t880 = ct{1781};
t881 = ct{1782};
t882 = ct{1783};
t883 = ct{1784};
t884 = ct{1785};
t885 = ct{1786};
t886 = ct{1787};
t887 = ct{1788};
t888 = ct{1789};
t889 = ct{1790};
t89 = ct{1791};
t890 = ct{1792};
t891 = ct{1793};
t892 = ct{1794};
t893 = ct{1795};
t894 = ct{1796};
t895 = ct{1797};
t896 = ct{1798};
t897 = ct{1799};
t898 = ct{1800};
t899 = ct{1801};
t9 = ct{1802};
t90 = ct{1803};
t900 = ct{1804};
t901 = ct{1805};
t902 = ct{1806};
t903 = ct{1807};
t904 = ct{1808};
t905 = ct{1809};
t906 = ct{1810};
t907 = ct{1811};
t908 = ct{1812};
t909 = ct{1813};
t91 = ct{1814};
t910 = ct{1815};
t911 = ct{1816};
t912 = ct{1817};
t913 = ct{1818};
t914 = ct{1819};
t915 = ct{1820};
t916 = ct{1821};
t917 = ct{1822};
t918 = ct{1823};
t919 = ct{1824};
t92 = ct{1825};
t920 = ct{1826};
t921 = ct{1827};
t922 = ct{1828};
t923 = ct{1829};
t924 = ct{1830};
t925 = ct{1831};
t926 = ct{1832};
t927 = ct{1833};
t928 = ct{1834};
t929 = ct{1835};
t93 = ct{1836};
t930 = ct{1837};
t931 = ct{1838};
t932 = ct{1839};
t933 = ct{1840};
t934 = ct{1841};
t935 = ct{1842};
t936 = ct{1843};
t937 = ct{1844};
t938 = ct{1845};
t939 = ct{1846};
t94 = ct{1847};
t940 = ct{1848};
t941 = ct{1849};
t942 = ct{1850};
t943 = ct{1851};
t944 = ct{1852};
t945 = ct{1853};
t946 = ct{1854};
t947 = ct{1855};
t948 = ct{1856};
t949 = ct{1857};
t95 = ct{1858};
t950 = ct{1859};
t951 = ct{1860};
t952 = ct{1861};
t953 = ct{1862};
t954 = ct{1863};
t955 = ct{1864};
t956 = ct{1865};
t957 = ct{1866};
t958 = ct{1867};
t96 = ct{1868};
t960 = ct{1869};
t961 = ct{1870};
t962 = ct{1871};
t963 = ct{1872};
t964 = ct{1873};
t965 = ct{1874};
t966 = ct{1875};
t967 = ct{1876};
t968 = ct{1877};
t969 = ct{1878};
t97 = ct{1879};
t970 = ct{1880};
t971 = ct{1881};
t972 = ct{1882};
t973 = ct{1883};
t974 = ct{1884};
t975 = ct{1885};
t976 = ct{1886};
t977 = ct{1887};
t978 = ct{1888};
t979 = ct{1889};
t98 = ct{1890};
t980 = ct{1891};
t981 = ct{1892};
t982 = ct{1893};
t983 = ct{1894};
t984 = ct{1895};
t985 = ct{1896};
t986 = ct{1897};
t987 = ct{1898};
t989 = ct{1899};
t99 = ct{1900};
t994 = ct{1901};
t995 = ct{1902};
t996 = ct{1903};
t997 = ct{1904};
t998 = ct{1905};
t999 = ct{1906};
th11_dot = ct{1907};
th12_dot = ct{1908};
th13_dot = ct{1909};
th21_dot = ct{1910};
th22_dot = ct{1911};
th23_dot = ct{1912};
th31_dot = ct{1913};
th32_dot = ct{1914};
th33_dot = ct{1915};
th41_dot = ct{1916};
th42_dot = ct{1917};
th43_dot = ct{1918};
zeta_dot = ct{1919};
t870 = t65.*t264;
t871 = t67.*t264;
t873 = t68.*t264;
t874 = t70.*t264;
t876 = t71.*t264;
t959 = -t657;
t988 = -t666;
t990 = t93+t155;
t991 = t94+t156;
t992 = t95+t157;
t993 = t96+t158;
t1002 = -t754;
t1003 = -t755;
t1004 = -t757;
t1005 = -t758;
t1006 = -t760;
t1007 = -t761;
t1008 = -t763;
t1009 = -t764;
t1034 = t46.*t470;
t1035 = t46.*t471;
t1036 = t46.*t472;
t1037 = t46.*t473;
t1050 = t46.*t474;
t1051 = t46.*t475;
t1052 = t46.*t476;
t1053 = t46.*t477;
t1078 = t3.*t72.*t165;
t1081 = t3.*t72.*t166;
t1084 = t3.*t72.*t167;
t1087 = t3.*t72.*t168;
t1174 = -t989;
t1189 = t3.*t18.*t528;
t1192 = t3.*t18.*t529;
t1372 = t46.*t546;
t1373 = t46.*t547;
t1374 = t46.*t548;
t1375 = t46.*t549;
t1376 = t46.*t550;
t1377 = t46.*t551;
t1378 = t46.*t552;
t1379 = t46.*t553;
t1380 = t46.*t554;
t1381 = t46.*t555;
t1382 = t46.*t556;
t1383 = t46.*t557;
t1448 = t18.*t92.*t190;
t1449 = t18.*t92.*t192;
t1450 = t18.*t92.*t196;
t1451 = t18.*t92.*t198;
t1452 = -t1287;
t1453 = -t1288;
t1454 = -t1289;
t1455 = -t1296;
t1456 = -t1297;
t1457 = -t1298;
t1500 = t47.*t793;
t1503 = t47.*t796;
t1506 = t47.*t799;
t1509 = t47.*t802;
t1516 = -t1352;
t1517 = -t1353;
t1518 = -t1354;
t1519 = -t1355;
t1520 = -t1356;
t1521 = -t1357;
t1522 = -t1358;
t1523 = -t1359;
t1540 = -t1392;
t1607 = -t1459;
t1637 = t92.*t794;
t1638 = t92.*t795;
t1639 = t92.*t797;
t1640 = t92.*t798;
t1641 = t92.*t800;
t1642 = t92.*t801;
t1643 = t92.*t803;
t1644 = t92.*t804;
t1646 = -t1570;
t1647 = -t1572;
t1648 = -t1574;
t1649 = -t1576;
t1650 = t46.*t933;
t1715 = t3.*t16.*t92.*t190;
t1716 = t3.*t16.*t92.*t192;
t1717 = t3.*t16.*t92.*t196;
t1718 = t3.*t16.*t92.*t198;
t1807 = -t1620;
t1840 = t97+t585;
t1857 = t31.*t1570;
t1858 = t31.*t1571;
t1859 = t31.*t1572;
t1860 = t31.*t1573;
t1861 = t31.*t1574;
t1862 = t31.*t1575;
t1863 = t31.*t1576;
t1864 = t31.*t1577;
t1909 = t92.*t1236;
t1910 = t92.*t1237;
t1911 = t92.*t1239;
t1912 = t92.*t1240;
t1913 = t92.*t1242;
t1914 = t92.*t1243;
t1915 = t92.*t1245;
t1916 = t92.*t1246;
t1925 = -t1824;
t1926 = -t1826;
t1927 = -t1828;
t1928 = -t1830;
t1970 = t92.*t1039;
t1971 = t92.*t1040;
t1972 = t92.*t1042;
t1973 = t92.*t1043;
t1974 = t92.*t1045;
t1975 = t92.*t1046;
t1976 = t92.*t1048;
t1977 = t92.*t1049;
t2066 = -t1941;
t2067 = -t1943;
t2068 = -t1945;
t2069 = -t1947;
t2071 = -t1955;
t2072 = -t1956;
t2073 = -t1958;
t2074 = -t1961;
t2095 = -t2010;
t2096 = -t2012;
t2097 = -t2014;
t2098 = -t2016;
t2116 = t46.*t1651;
t2117 = t46.*t1652;
t2118 = t46.*t1653;
t2119 = t46.*t1654;
t2120 = t46.*t1655;
t2121 = t46.*t1656;
t2122 = t46.*t1657;
t2123 = t46.*t1658;
t2132 = t47.*t1663;
t2133 = t47.*t1664;
t2134 = t47.*t1667;
t2135 = t47.*t1668;
t2136 = t47.*t1671;
t2137 = t47.*t1672;
t2138 = t47.*t1673;
t2139 = t47.*t1674;
t2148 = t103+t657;
t2149 = t105+t666;
t2150 = t92.*t1579;
t2151 = t92.*t1580;
t2152 = t92.*t1582;
t2153 = t92.*t1583;
t2154 = t92.*t1585;
t2155 = t92.*t1586;
t2156 = t92.*t1588;
t2157 = t92.*t1589;
t2166 = t74.*t87.*t92.*t286;
t2167 = t74.*t87.*t92.*t287;
t2168 = t74.*t87.*t92.*t288;
t2169 = t74.*t87.*t92.*t289;
t2170 = t74.*t87.*t92.*t290;
t2171 = t74.*t87.*t92.*t291;
t2172 = t74.*t87.*t92.*t292;
t2173 = t74.*t87.*t92.*t293;
t723 = t89+t111;
t724 = t90+t110;
t829 = t3.*t325;
t832 = t3.*t326;
t835 = t3.*t327;
t838 = t3.*t328;
t1949 = (t92.*t359)./2.0;
t2175 = t103+t959;
t2176 = t105+t988;
t2070 = -t1949;
t2099 = (t92.*t724)./2.0;
t2177 = t104+t1949;
t2174 = -t2099;
t2178 = t104+t2070;
t2179 = t102+t2099;
t2180 = t102+t2174;
et1 = phi_dot.*t91.*(1.2e+1./2.5e+1)+phi_dot.*t101.*(1.2e+1./2.5e+1)-psi_dot.*t88.*(1.2e+1./2.5e+1)-psi_dot.*t100.*(1.2e+1./2.5e+1)+phi_dot.*t19.*t91.*(3.0./5.0e+1)+phi_dot.*t20.*t91.*(3.0./5.0e+1)+phi_dot.*t21.*t91.*(3.0./5.0e+1)+phi_dot.*t22.*t91.*(3.0./5.0e+1)+phi_dot.*t23.*t91.*(3.0./5.0e+1)+phi_dot.*t24.*t91.*(3.0./5.0e+1)+phi_dot.*t25.*t91.*(3.0./5.0e+1)+phi_dot.*t26.*t91.*(3.0./5.0e+1)+phi_dot.*t27.*t91.*(3.0./5.0e+1)+phi_dot.*t28.*t91.*(3.0./5.0e+1)+phi_dot.*t19.*t101.*(3.0./5.0e+1)+phi_dot.*t29.*t91.*(3.0./5.0e+1)+phi_dot.*t20.*t101.*(3.0./5.0e+1)+phi_dot.*t30.*t91.*(3.0./5.0e+1)+phi_dot.*t21.*t101.*(3.0./5.0e+1)+phi_dot.*t22.*t101.*(3.0./5.0e+1)+phi_dot.*t23.*t101.*(3.0./5.0e+1)+phi_dot.*t24.*t101.*(3.0./5.0e+1)+phi_dot.*t25.*t101.*(3.0./5.0e+1)+phi_dot.*t26.*t101.*(3.0./5.0e+1);
et2 = phi_dot.*t27.*t101.*(3.0./5.0e+1)+phi_dot.*t28.*t101.*(3.0./5.0e+1)+phi_dot.*t29.*t101.*(3.0./5.0e+1)+phi_dot.*t30.*t101.*(3.0./5.0e+1)-psi_dot.*t19.*t88.*(3.0./5.0e+1)-psi_dot.*t20.*t88.*(3.0./5.0e+1)-psi_dot.*t21.*t88.*(3.0./5.0e+1)-psi_dot.*t22.*t88.*(3.0./5.0e+1)-psi_dot.*t23.*t88.*(3.0./5.0e+1)-psi_dot.*t24.*t88.*(3.0./5.0e+1)-psi_dot.*t25.*t88.*(3.0./5.0e+1)-psi_dot.*t26.*t88.*(3.0./5.0e+1)-psi_dot.*t27.*t88.*(3.0./5.0e+1)-psi_dot.*t28.*t88.*(3.0./5.0e+1)-psi_dot.*t29.*t88.*(3.0./5.0e+1)-psi_dot.*t30.*t88.*(3.0./5.0e+1)-psi_dot.*t19.*t100.*(3.0./5.0e+1)-psi_dot.*t20.*t100.*(3.0./5.0e+1)-psi_dot.*t21.*t100.*(3.0./5.0e+1)-psi_dot.*t22.*t100.*(3.0./5.0e+1)-psi_dot.*t23.*t100.*(3.0./5.0e+1)-psi_dot.*t24.*t100.*(3.0./5.0e+1);
et3 = psi_dot.*t25.*t100.*(-3.0./5.0e+1)-psi_dot.*t26.*t100.*(3.0./5.0e+1)-psi_dot.*t27.*t100.*(3.0./5.0e+1)-psi_dot.*t28.*t100.*(3.0./5.0e+1)-psi_dot.*t29.*t100.*(3.0./5.0e+1)-psi_dot.*t30.*t100.*(3.0./5.0e+1)-t4.*t89.*th11_dot.*(3.0./5.0e+1)-t5.*t89.*th12_dot.*(3.0./5.0e+1)-t6.*t89.*th13_dot.*(3.0./5.0e+1)+t4.*t99.*th11_dot.*(3.0./5.0e+1)+t5.*t99.*th12_dot.*(3.0./5.0e+1)-t7.*t89.*th21_dot.*(3.0./5.0e+1)+t6.*t99.*th13_dot.*(3.0./5.0e+1)-t8.*t89.*th22_dot.*(3.0./5.0e+1)-t9.*t89.*th23_dot.*(3.0./5.0e+1)+t7.*t99.*th21_dot.*(3.0./5.0e+1)+t8.*t99.*th22_dot.*(3.0./5.0e+1)-t10.*t89.*th31_dot.*(3.0./5.0e+1)+t9.*t99.*th23_dot.*(3.0./5.0e+1)-t11.*t89.*th32_dot.*(3.0./5.0e+1)-t12.*t89.*th33_dot.*(3.0./5.0e+1)+t10.*t99.*th31_dot.*(3.0./5.0e+1)+t11.*t99.*th32_dot.*(3.0./5.0e+1);
et4 = t13.*t89.*th41_dot.*(-3.0./5.0e+1)+t12.*t99.*th33_dot.*(3.0./5.0e+1)-t14.*t89.*th42_dot.*(3.0./5.0e+1)-t15.*t89.*th43_dot.*(3.0./5.0e+1)+t13.*t99.*th41_dot.*(3.0./5.0e+1)+t14.*t99.*th42_dot.*(3.0./5.0e+1)+t15.*t99.*th43_dot.*(3.0./5.0e+1)+t16.*t90.*zeta_dot.*(1.2e+1./2.5e+1)-phi_dot.*t2.*t4.*t16.*(3.0./5.0e+1)+phi_dot.*t2.*t5.*t16.*(3.0./1.0e+2)+phi_dot.*t2.*t6.*t16.*(3.0./1.0e+2)-phi_dot.*t2.*t7.*t16.*(3.0./5.0e+1)+phi_dot.*t2.*t8.*t16.*(3.0./1.0e+2)+phi_dot.*t2.*t9.*t16.*(3.0./1.0e+2)-phi_dot.*t2.*t10.*t16.*(3.0./5.0e+1)+phi_dot.*t2.*t11.*t16.*(3.0./1.0e+2)+phi_dot.*t2.*t12.*t16.*(3.0./1.0e+2)-phi_dot.*t2.*t13.*t16.*(3.0./5.0e+1)+phi_dot.*t2.*t14.*t16.*(3.0./1.0e+2)+phi_dot.*t2.*t15.*t16.*(3.0./1.0e+2)+phi_dot.*t5.*t90.*t92.*(3.0./1.0e+2);
et5 = phi_dot.*t6.*t90.*t92.*(-3.0./1.0e+2)+phi_dot.*t8.*t90.*t92.*(3.0./1.0e+2)-phi_dot.*t9.*t90.*t92.*(3.0./1.0e+2)+phi_dot.*t11.*t90.*t92.*(3.0./1.0e+2)-phi_dot.*t12.*t90.*t92.*(3.0./1.0e+2)-phi_dot.*t5.*t92.*t98.*(3.0./1.0e+2)+phi_dot.*t6.*t92.*t98.*(3.0./1.0e+2)+phi_dot.*t14.*t90.*t92.*(3.0./1.0e+2)-phi_dot.*t15.*t90.*t92.*(3.0./1.0e+2)-phi_dot.*t8.*t92.*t98.*(3.0./1.0e+2)+phi_dot.*t9.*t92.*t98.*(3.0./1.0e+2)-phi_dot.*t11.*t92.*t98.*(3.0./1.0e+2)+phi_dot.*t12.*t92.*t98.*(3.0./1.0e+2)-phi_dot.*t14.*t92.*t98.*(3.0./1.0e+2)+phi_dot.*t15.*t92.*t98.*(3.0./1.0e+2)+psi_dot.*t5.*t89.*t92.*(3.0./1.0e+2)-psi_dot.*t6.*t89.*t92.*(3.0./1.0e+2)+psi_dot.*t8.*t89.*t92.*(3.0./1.0e+2)-psi_dot.*t9.*t89.*t92.*(3.0./1.0e+2);
et6 = psi_dot.*t11.*t89.*t92.*(3.0./1.0e+2)-psi_dot.*t12.*t89.*t92.*(3.0./1.0e+2)+psi_dot.*t14.*t89.*t92.*(3.0./1.0e+2)-psi_dot.*t5.*t92.*t99.*(3.0./1.0e+2)-psi_dot.*t15.*t89.*t92.*(3.0./1.0e+2)+psi_dot.*t6.*t92.*t99.*(3.0./1.0e+2)-psi_dot.*t8.*t92.*t99.*(3.0./1.0e+2)+psi_dot.*t9.*t92.*t99.*(3.0./1.0e+2)-psi_dot.*t11.*t92.*t99.*(3.0./1.0e+2)+psi_dot.*t12.*t92.*t99.*(3.0./1.0e+2)-psi_dot.*t14.*t92.*t99.*(3.0./1.0e+2)+psi_dot.*t15.*t92.*t99.*(3.0./1.0e+2)+t16.*t17.*t19.*th11_dot.*(3.0./5.0e+1)-t16.*t17.*t20.*th12_dot.*(3.0./1.0e+2)-t16.*t17.*t21.*th13_dot.*(3.0./1.0e+2)+t16.*t17.*t22.*th21_dot.*(3.0./5.0e+1)-t16.*t17.*t23.*th22_dot.*(3.0./1.0e+2)-t16.*t17.*t24.*th23_dot.*(3.0./1.0e+2)+t16.*t17.*t25.*th31_dot.*(3.0./5.0e+1);
et7 = t16.*t17.*t26.*th32_dot.*(-3.0./1.0e+2)-t16.*t17.*t27.*th33_dot.*(3.0./1.0e+2)+t16.*t17.*t28.*th41_dot.*(3.0./5.0e+1)-t16.*t17.*t29.*th42_dot.*(3.0./1.0e+2)-t16.*t17.*t30.*th43_dot.*(3.0./1.0e+2)+t20.*t88.*t92.*th12_dot.*(3.0./1.0e+2)-t21.*t88.*t92.*th13_dot.*(3.0./1.0e+2)+t20.*t92.*t100.*th12_dot.*(3.0./1.0e+2)+t23.*t88.*t92.*th22_dot.*(3.0./1.0e+2)-t21.*t92.*t100.*th13_dot.*(3.0./1.0e+2)-t24.*t88.*t92.*th23_dot.*(3.0./1.0e+2)+t23.*t92.*t100.*th22_dot.*(3.0./1.0e+2)+t26.*t88.*t92.*th32_dot.*(3.0./1.0e+2)-t24.*t92.*t100.*th23_dot.*(3.0./1.0e+2)-t27.*t88.*t92.*th33_dot.*(3.0./1.0e+2)+t26.*t92.*t100.*th32_dot.*(3.0./1.0e+2)+t29.*t88.*t92.*th42_dot.*(3.0./1.0e+2)-t27.*t92.*t100.*th33_dot.*(3.0./1.0e+2)-t30.*t88.*t92.*th43_dot.*(3.0./1.0e+2);
et8 = t29.*t92.*t100.*th42_dot.*(3.0./1.0e+2)-t30.*t92.*t100.*th43_dot.*(3.0./1.0e+2)+t4.*t17.*t31.*zeta_dot.*(3.0./5.0e+1)-t5.*t17.*t31.*zeta_dot.*(3.0./1.0e+2)-t6.*t17.*t31.*zeta_dot.*(3.0./1.0e+2)+t7.*t17.*t31.*zeta_dot.*(3.0./5.0e+1)-t8.*t17.*t31.*zeta_dot.*(3.0./1.0e+2)-t9.*t17.*t31.*zeta_dot.*(3.0./1.0e+2)+t10.*t17.*t31.*zeta_dot.*(3.0./5.0e+1)-t11.*t17.*t31.*zeta_dot.*(3.0./1.0e+2)-t12.*t17.*t31.*zeta_dot.*(3.0./1.0e+2)+t13.*t17.*t31.*zeta_dot.*(3.0./5.0e+1)-t14.*t17.*t31.*zeta_dot.*(3.0./1.0e+2)-t15.*t17.*t31.*zeta_dot.*(3.0./1.0e+2)+t16.*t19.*t90.*zeta_dot.*(3.0./5.0e+1)+t16.*t20.*t90.*zeta_dot.*(3.0./5.0e+1)+t16.*t21.*t90.*zeta_dot.*(3.0./5.0e+1)+t16.*t22.*t90.*zeta_dot.*(3.0./5.0e+1)+t16.*t23.*t90.*zeta_dot.*(3.0./5.0e+1)+t16.*t24.*t90.*zeta_dot.*(3.0./5.0e+1);
et9 = t16.*t25.*t90.*zeta_dot.*(3.0./5.0e+1)+t16.*t26.*t90.*zeta_dot.*(3.0./5.0e+1)+t16.*t27.*t90.*zeta_dot.*(3.0./5.0e+1)+t16.*t28.*t90.*zeta_dot.*(3.0./5.0e+1)+t16.*t29.*t90.*zeta_dot.*(3.0./5.0e+1)+t16.*t30.*t90.*zeta_dot.*(3.0./5.0e+1)-t5.*t16.*t91.*t92.*zeta_dot.*(3.0./1.0e+2)+t6.*t16.*t91.*t92.*zeta_dot.*(3.0./1.0e+2)-t8.*t16.*t91.*t92.*zeta_dot.*(3.0./1.0e+2)+t9.*t16.*t91.*t92.*zeta_dot.*(3.0./1.0e+2)-t11.*t16.*t91.*t92.*zeta_dot.*(3.0./1.0e+2)+t12.*t16.*t91.*t92.*zeta_dot.*(3.0./1.0e+2)-t14.*t16.*t91.*t92.*zeta_dot.*(3.0./1.0e+2)+t15.*t16.*t91.*t92.*zeta_dot.*(3.0./1.0e+2);
et10 = t101.*zeta_dot.*(1.2e+1./2.5e+1)+phi_dot.*t16.*t90.*(1.2e+1./2.5e+1)+psi_dot.*t16.*t89.*(1.2e+1./2.5e+1)+t19.*t101.*zeta_dot.*(3.0./5.0e+1)+t20.*t101.*zeta_dot.*(3.0./5.0e+1)+t21.*t101.*zeta_dot.*(3.0./5.0e+1)+t22.*t101.*zeta_dot.*(3.0./5.0e+1)+t23.*t101.*zeta_dot.*(3.0./5.0e+1)+t24.*t101.*zeta_dot.*(3.0./5.0e+1)+t25.*t101.*zeta_dot.*(3.0./5.0e+1)+t26.*t101.*zeta_dot.*(3.0./5.0e+1)+t27.*t101.*zeta_dot.*(3.0./5.0e+1)+t28.*t101.*zeta_dot.*(3.0./5.0e+1)+t29.*t101.*zeta_dot.*(3.0./5.0e+1)+t30.*t101.*zeta_dot.*(3.0./5.0e+1)+phi_dot.*t4.*t17.*t31.*(3.0./5.0e+1)-phi_dot.*t5.*t17.*t31.*(3.0./1.0e+2)-phi_dot.*t6.*t17.*t31.*(3.0./1.0e+2)+phi_dot.*t7.*t17.*t31.*(3.0./5.0e+1)-phi_dot.*t8.*t17.*t31.*(3.0./1.0e+2)-phi_dot.*t9.*t17.*t31.*(3.0./1.0e+2)+phi_dot.*t10.*t17.*t31.*(3.0./5.0e+1);
et11 = phi_dot.*t11.*t17.*t31.*(-3.0./1.0e+2)-phi_dot.*t12.*t17.*t31.*(3.0./1.0e+2)+phi_dot.*t13.*t17.*t31.*(3.0./5.0e+1)-phi_dot.*t14.*t17.*t31.*(3.0./1.0e+2)-phi_dot.*t15.*t17.*t31.*(3.0./1.0e+2)+phi_dot.*t16.*t19.*t90.*(3.0./5.0e+1)+phi_dot.*t16.*t20.*t90.*(3.0./5.0e+1)+phi_dot.*t16.*t21.*t90.*(3.0./5.0e+1)+phi_dot.*t16.*t22.*t90.*(3.0./5.0e+1)+phi_dot.*t16.*t23.*t90.*(3.0./5.0e+1)+phi_dot.*t16.*t24.*t90.*(3.0./5.0e+1)+phi_dot.*t16.*t25.*t90.*(3.0./5.0e+1)+phi_dot.*t16.*t26.*t90.*(3.0./5.0e+1)+phi_dot.*t16.*t27.*t90.*(3.0./5.0e+1)+phi_dot.*t16.*t28.*t90.*(3.0./5.0e+1)+phi_dot.*t16.*t29.*t90.*(3.0./5.0e+1)+phi_dot.*t16.*t30.*t90.*(3.0./5.0e+1)+psi_dot.*t16.*t19.*t89.*(3.0./5.0e+1)+psi_dot.*t16.*t20.*t89.*(3.0./5.0e+1)+psi_dot.*t16.*t21.*t89.*(3.0./5.0e+1)+psi_dot.*t16.*t22.*t89.*(3.0./5.0e+1);
et12 = psi_dot.*t16.*t23.*t89.*(3.0./5.0e+1)+psi_dot.*t16.*t24.*t89.*(3.0./5.0e+1)+psi_dot.*t16.*t25.*t89.*(3.0./5.0e+1)+psi_dot.*t16.*t26.*t89.*(3.0./5.0e+1)+psi_dot.*t16.*t27.*t89.*(3.0./5.0e+1)+psi_dot.*t16.*t28.*t89.*(3.0./5.0e+1)+psi_dot.*t16.*t29.*t89.*(3.0./5.0e+1)+psi_dot.*t16.*t30.*t89.*(3.0./5.0e+1)+t2.*t19.*t31.*th11_dot.*(3.0./5.0e+1)-t2.*t20.*t31.*th12_dot.*(3.0./1.0e+2)-t2.*t21.*t31.*th13_dot.*(3.0./1.0e+2)+t2.*t22.*t31.*th21_dot.*(3.0./5.0e+1)-t2.*t23.*t31.*th22_dot.*(3.0./1.0e+2)-t2.*t24.*t31.*th23_dot.*(3.0./1.0e+2)+t2.*t25.*t31.*th31_dot.*(3.0./5.0e+1)-t2.*t26.*t31.*th32_dot.*(3.0./1.0e+2)-t2.*t27.*t31.*th33_dot.*(3.0./1.0e+2)+t2.*t28.*t31.*th41_dot.*(3.0./5.0e+1)-t2.*t29.*t31.*th42_dot.*(3.0./1.0e+2)-t2.*t30.*t31.*th43_dot.*(3.0./1.0e+2);
et13 = t4.*t16.*t88.*th11_dot.*(-3.0./5.0e+1)-t5.*t16.*t88.*th12_dot.*(3.0./5.0e+1)-t6.*t16.*t88.*th13_dot.*(3.0./5.0e+1)-t7.*t16.*t88.*th21_dot.*(3.0./5.0e+1)-t8.*t16.*t88.*th22_dot.*(3.0./5.0e+1)-t9.*t16.*t88.*th23_dot.*(3.0./5.0e+1)-t10.*t16.*t88.*th31_dot.*(3.0./5.0e+1)-t11.*t16.*t88.*th32_dot.*(3.0./5.0e+1)-t12.*t16.*t88.*th33_dot.*(3.0./5.0e+1)-t13.*t16.*t88.*th41_dot.*(3.0./5.0e+1)-t14.*t16.*t88.*th42_dot.*(3.0./5.0e+1)-t15.*t16.*t88.*th43_dot.*(3.0./5.0e+1)-t2.*t4.*t16.*zeta_dot.*(3.0./5.0e+1)+t2.*t5.*t16.*zeta_dot.*(3.0./1.0e+2)+t2.*t6.*t16.*zeta_dot.*(3.0./1.0e+2)-t2.*t7.*t16.*zeta_dot.*(3.0./5.0e+1)+t2.*t8.*t16.*zeta_dot.*(3.0./1.0e+2)+t2.*t9.*t16.*zeta_dot.*(3.0./1.0e+2)-t2.*t10.*t16.*zeta_dot.*(3.0./5.0e+1)+t2.*t11.*t16.*zeta_dot.*(3.0./1.0e+2);
et14 = t2.*t12.*t16.*zeta_dot.*(3.0./1.0e+2)-t2.*t13.*t16.*zeta_dot.*(3.0./5.0e+1)+t2.*t14.*t16.*zeta_dot.*(3.0./1.0e+2)+t2.*t15.*t16.*zeta_dot.*(3.0./1.0e+2)-t5.*t92.*t98.*zeta_dot.*(3.0./1.0e+2)+t6.*t92.*t98.*zeta_dot.*(3.0./1.0e+2)-t8.*t92.*t98.*zeta_dot.*(3.0./1.0e+2)+t9.*t92.*t98.*zeta_dot.*(3.0./1.0e+2)-t11.*t92.*t98.*zeta_dot.*(3.0./1.0e+2)+t12.*t92.*t98.*zeta_dot.*(3.0./1.0e+2)-t14.*t92.*t98.*zeta_dot.*(3.0./1.0e+2)+t15.*t92.*t98.*zeta_dot.*(3.0./1.0e+2)-phi_dot.*t5.*t16.*t91.*t92.*(3.0./1.0e+2)+phi_dot.*t6.*t16.*t91.*t92.*(3.0./1.0e+2)-phi_dot.*t8.*t16.*t91.*t92.*(3.0./1.0e+2)+phi_dot.*t9.*t16.*t91.*t92.*(3.0./1.0e+2)-phi_dot.*t11.*t16.*t91.*t92.*(3.0./1.0e+2)+phi_dot.*t12.*t16.*t91.*t92.*(3.0./1.0e+2);
et15 = phi_dot.*t14.*t16.*t91.*t92.*(-3.0./1.0e+2)+phi_dot.*t15.*t16.*t91.*t92.*(3.0./1.0e+2)+psi_dot.*t5.*t16.*t88.*t92.*(3.0./1.0e+2)-psi_dot.*t6.*t16.*t88.*t92.*(3.0./1.0e+2)+psi_dot.*t8.*t16.*t88.*t92.*(3.0./1.0e+2)-psi_dot.*t9.*t16.*t88.*t92.*(3.0./1.0e+2)+psi_dot.*t11.*t16.*t88.*t92.*(3.0./1.0e+2)-psi_dot.*t12.*t16.*t88.*t92.*(3.0./1.0e+2)+psi_dot.*t14.*t16.*t88.*t92.*(3.0./1.0e+2)-psi_dot.*t15.*t16.*t88.*t92.*(3.0./1.0e+2)-t16.*t20.*t89.*t92.*th12_dot.*(3.0./1.0e+2)+t16.*t21.*t89.*t92.*th13_dot.*(3.0./1.0e+2)-t16.*t23.*t89.*t92.*th22_dot.*(3.0./1.0e+2)+t16.*t24.*t89.*t92.*th23_dot.*(3.0./1.0e+2)-t16.*t26.*t89.*t92.*th32_dot.*(3.0./1.0e+2)+t16.*t27.*t89.*t92.*th33_dot.*(3.0./1.0e+2)-t16.*t29.*t89.*t92.*th42_dot.*(3.0./1.0e+2);
et16 = t16.*t30.*t89.*t92.*th43_dot.*(3.0./1.0e+2);
et17 = phi_dot.*t88.*(-1.2e+1./2.5e+1)-phi_dot.*t100.*(1.2e+1./2.5e+1)+psi_dot.*t91.*(1.2e+1./2.5e+1)+psi_dot.*t101.*(1.2e+1./2.5e+1)-phi_dot.*t19.*t88.*(3.0./5.0e+1)-phi_dot.*t20.*t88.*(3.0./5.0e+1)-phi_dot.*t21.*t88.*(3.0./5.0e+1)-phi_dot.*t22.*t88.*(3.0./5.0e+1)-phi_dot.*t23.*t88.*(3.0./5.0e+1)-phi_dot.*t24.*t88.*(3.0./5.0e+1)-phi_dot.*t25.*t88.*(3.0./5.0e+1)-phi_dot.*t26.*t88.*(3.0./5.0e+1)-phi_dot.*t27.*t88.*(3.0./5.0e+1)-phi_dot.*t28.*t88.*(3.0./5.0e+1)-phi_dot.*t29.*t88.*(3.0./5.0e+1)-phi_dot.*t30.*t88.*(3.0./5.0e+1)-phi_dot.*t19.*t100.*(3.0./5.0e+1)-phi_dot.*t20.*t100.*(3.0./5.0e+1)-phi_dot.*t21.*t100.*(3.0./5.0e+1)-phi_dot.*t22.*t100.*(3.0./5.0e+1)-phi_dot.*t23.*t100.*(3.0./5.0e+1)-phi_dot.*t24.*t100.*(3.0./5.0e+1);
et18 = phi_dot.*t25.*t100.*(-3.0./5.0e+1)-phi_dot.*t26.*t100.*(3.0./5.0e+1)-phi_dot.*t27.*t100.*(3.0./5.0e+1)-phi_dot.*t28.*t100.*(3.0./5.0e+1)-phi_dot.*t29.*t100.*(3.0./5.0e+1)-phi_dot.*t30.*t100.*(3.0./5.0e+1)+psi_dot.*t19.*t91.*(3.0./5.0e+1)+psi_dot.*t20.*t91.*(3.0./5.0e+1)+psi_dot.*t21.*t91.*(3.0./5.0e+1)+psi_dot.*t22.*t91.*(3.0./5.0e+1)+psi_dot.*t23.*t91.*(3.0./5.0e+1)+psi_dot.*t24.*t91.*(3.0./5.0e+1)+psi_dot.*t25.*t91.*(3.0./5.0e+1)+psi_dot.*t26.*t91.*(3.0./5.0e+1)+psi_dot.*t27.*t91.*(3.0./5.0e+1)+psi_dot.*t28.*t91.*(3.0./5.0e+1)+psi_dot.*t19.*t101.*(3.0./5.0e+1)+psi_dot.*t29.*t91.*(3.0./5.0e+1)+psi_dot.*t20.*t101.*(3.0./5.0e+1)+psi_dot.*t30.*t91.*(3.0./5.0e+1)+psi_dot.*t21.*t101.*(3.0./5.0e+1)+psi_dot.*t22.*t101.*(3.0./5.0e+1)+psi_dot.*t23.*t101.*(3.0./5.0e+1)+psi_dot.*t24.*t101.*(3.0./5.0e+1);
et19 = psi_dot.*t25.*t101.*(3.0./5.0e+1)+psi_dot.*t26.*t101.*(3.0./5.0e+1)+psi_dot.*t27.*t101.*(3.0./5.0e+1)+psi_dot.*t28.*t101.*(3.0./5.0e+1)+psi_dot.*t29.*t101.*(3.0./5.0e+1)+psi_dot.*t30.*t101.*(3.0./5.0e+1)-t4.*t90.*th11_dot.*(3.0./5.0e+1)-t5.*t90.*th12_dot.*(3.0./5.0e+1)-t6.*t90.*th13_dot.*(3.0./5.0e+1)+t4.*t98.*th11_dot.*(3.0./5.0e+1)+t5.*t98.*th12_dot.*(3.0./5.0e+1)+t6.*t98.*th13_dot.*(3.0./5.0e+1)-t7.*t90.*th21_dot.*(3.0./5.0e+1)-t8.*t90.*th22_dot.*(3.0./5.0e+1)-t9.*t90.*th23_dot.*(3.0./5.0e+1)+t7.*t98.*th21_dot.*(3.0./5.0e+1)+t8.*t98.*th22_dot.*(3.0./5.0e+1)+t9.*t98.*th23_dot.*(3.0./5.0e+1)-t10.*t90.*th31_dot.*(3.0./5.0e+1)-t11.*t90.*th32_dot.*(3.0./5.0e+1)-t12.*t90.*th33_dot.*(3.0./5.0e+1)+t10.*t98.*th31_dot.*(3.0./5.0e+1)+t11.*t98.*th32_dot.*(3.0./5.0e+1);
et20 = t12.*t98.*th33_dot.*(3.0./5.0e+1)-t13.*t90.*th41_dot.*(3.0./5.0e+1)-t14.*t90.*th42_dot.*(3.0./5.0e+1)-t15.*t90.*th43_dot.*(3.0./5.0e+1)+t13.*t98.*th41_dot.*(3.0./5.0e+1)+t14.*t98.*th42_dot.*(3.0./5.0e+1)+t15.*t98.*th43_dot.*(3.0./5.0e+1)+t16.*t89.*zeta_dot.*(1.2e+1./2.5e+1)+phi_dot.*t5.*t89.*t92.*(3.0./1.0e+2)-phi_dot.*t6.*t89.*t92.*(3.0./1.0e+2)+phi_dot.*t8.*t89.*t92.*(3.0./1.0e+2)-phi_dot.*t9.*t89.*t92.*(3.0./1.0e+2)+phi_dot.*t11.*t89.*t92.*(3.0./1.0e+2)-phi_dot.*t12.*t89.*t92.*(3.0./1.0e+2)+phi_dot.*t14.*t89.*t92.*(3.0./1.0e+2)-phi_dot.*t5.*t92.*t99.*(3.0./1.0e+2)-phi_dot.*t15.*t89.*t92.*(3.0./1.0e+2)+phi_dot.*t6.*t92.*t99.*(3.0./1.0e+2)-phi_dot.*t8.*t92.*t99.*(3.0./1.0e+2)+phi_dot.*t9.*t92.*t99.*(3.0./1.0e+2);
et21 = phi_dot.*t11.*t92.*t99.*(-3.0./1.0e+2)+phi_dot.*t12.*t92.*t99.*(3.0./1.0e+2)-phi_dot.*t14.*t92.*t99.*(3.0./1.0e+2)+phi_dot.*t15.*t92.*t99.*(3.0./1.0e+2)+psi_dot.*t5.*t90.*t92.*(3.0./1.0e+2)-psi_dot.*t6.*t90.*t92.*(3.0./1.0e+2)+psi_dot.*t8.*t90.*t92.*(3.0./1.0e+2)-psi_dot.*t9.*t90.*t92.*(3.0./1.0e+2)+psi_dot.*t11.*t90.*t92.*(3.0./1.0e+2)-psi_dot.*t12.*t90.*t92.*(3.0./1.0e+2)-psi_dot.*t5.*t92.*t98.*(3.0./1.0e+2)+psi_dot.*t6.*t92.*t98.*(3.0./1.0e+2)+psi_dot.*t14.*t90.*t92.*(3.0./1.0e+2)-psi_dot.*t15.*t90.*t92.*(3.0./1.0e+2)-psi_dot.*t8.*t92.*t98.*(3.0./1.0e+2)+psi_dot.*t9.*t92.*t98.*(3.0./1.0e+2)-psi_dot.*t11.*t92.*t98.*(3.0./1.0e+2)+psi_dot.*t12.*t92.*t98.*(3.0./1.0e+2)-psi_dot.*t14.*t92.*t98.*(3.0./1.0e+2);
et22 = psi_dot.*t15.*t92.*t98.*(3.0./1.0e+2)-t20.*t91.*t92.*th12_dot.*(3.0./1.0e+2)+t21.*t91.*t92.*th13_dot.*(3.0./1.0e+2)-t20.*t92.*t101.*th12_dot.*(3.0./1.0e+2)+t21.*t92.*t101.*th13_dot.*(3.0./1.0e+2)-t23.*t91.*t92.*th22_dot.*(3.0./1.0e+2)+t24.*t91.*t92.*th23_dot.*(3.0./1.0e+2)-t23.*t92.*t101.*th22_dot.*(3.0./1.0e+2)+t24.*t92.*t101.*th23_dot.*(3.0./1.0e+2)-t26.*t91.*t92.*th32_dot.*(3.0./1.0e+2)+t27.*t91.*t92.*th33_dot.*(3.0./1.0e+2)-t26.*t92.*t101.*th32_dot.*(3.0./1.0e+2)+t27.*t92.*t101.*th33_dot.*(3.0./1.0e+2)-t29.*t91.*t92.*th42_dot.*(3.0./1.0e+2)+t30.*t91.*t92.*th43_dot.*(3.0./1.0e+2)-t29.*t92.*t101.*th42_dot.*(3.0./1.0e+2)+t30.*t92.*t101.*th43_dot.*(3.0./1.0e+2)+t16.*t19.*t89.*zeta_dot.*(3.0./5.0e+1)+t16.*t20.*t89.*zeta_dot.*(3.0./5.0e+1);
et23 = t16.*t21.*t89.*zeta_dot.*(3.0./5.0e+1)+t16.*t22.*t89.*zeta_dot.*(3.0./5.0e+1)+t16.*t23.*t89.*zeta_dot.*(3.0./5.0e+1)+t16.*t24.*t89.*zeta_dot.*(3.0./5.0e+1)+t16.*t25.*t89.*zeta_dot.*(3.0./5.0e+1)+t16.*t26.*t89.*zeta_dot.*(3.0./5.0e+1)+t16.*t27.*t89.*zeta_dot.*(3.0./5.0e+1)+t16.*t28.*t89.*zeta_dot.*(3.0./5.0e+1)+t16.*t29.*t89.*zeta_dot.*(3.0./5.0e+1)+t16.*t30.*t89.*zeta_dot.*(3.0./5.0e+1)+t5.*t16.*t88.*t92.*zeta_dot.*(3.0./1.0e+2)-t6.*t16.*t88.*t92.*zeta_dot.*(3.0./1.0e+2)+t8.*t16.*t88.*t92.*zeta_dot.*(3.0./1.0e+2)-t9.*t16.*t88.*t92.*zeta_dot.*(3.0./1.0e+2)+t11.*t16.*t88.*t92.*zeta_dot.*(3.0./1.0e+2)-t12.*t16.*t88.*t92.*zeta_dot.*(3.0./1.0e+2)+t14.*t16.*t88.*t92.*zeta_dot.*(3.0./1.0e+2)-t15.*t16.*t88.*t92.*zeta_dot.*(3.0./1.0e+2);
et24 = phi_dot.*t89.*(-1.2e+1./2.5e+1)+phi_dot.*t99.*(1.2e+1./2.5e+1)-psi_dot.*t90.*(1.2e+1./2.5e+1)+psi_dot.*t98.*(1.2e+1./2.5e+1)-phi_dot.*t19.*t89.*(3.0./5.0e+1)-phi_dot.*t20.*t89.*(3.0./5.0e+1)-phi_dot.*t21.*t89.*(3.0./5.0e+1)-phi_dot.*t22.*t89.*(3.0./5.0e+1)-phi_dot.*t23.*t89.*(3.0./5.0e+1)-phi_dot.*t24.*t89.*(3.0./5.0e+1)-phi_dot.*t25.*t89.*(3.0./5.0e+1)-phi_dot.*t26.*t89.*(3.0./5.0e+1)-phi_dot.*t27.*t89.*(3.0./5.0e+1)-phi_dot.*t28.*t89.*(3.0./5.0e+1)+phi_dot.*t19.*t99.*(3.0./5.0e+1)-phi_dot.*t29.*t89.*(3.0./5.0e+1)+phi_dot.*t20.*t99.*(3.0./5.0e+1)-phi_dot.*t30.*t89.*(3.0./5.0e+1)+phi_dot.*t21.*t99.*(3.0./5.0e+1)+phi_dot.*t22.*t99.*(3.0./5.0e+1)+phi_dot.*t23.*t99.*(3.0./5.0e+1)+phi_dot.*t24.*t99.*(3.0./5.0e+1)+phi_dot.*t25.*t99.*(3.0./5.0e+1);
et25 = phi_dot.*t26.*t99.*(3.0./5.0e+1)+phi_dot.*t27.*t99.*(3.0./5.0e+1)+phi_dot.*t28.*t99.*(3.0./5.0e+1)+phi_dot.*t29.*t99.*(3.0./5.0e+1)+phi_dot.*t30.*t99.*(3.0./5.0e+1)-psi_dot.*t19.*t90.*(3.0./5.0e+1)-psi_dot.*t20.*t90.*(3.0./5.0e+1)-psi_dot.*t21.*t90.*(3.0./5.0e+1)-psi_dot.*t22.*t90.*(3.0./5.0e+1)-psi_dot.*t23.*t90.*(3.0./5.0e+1)-psi_dot.*t24.*t90.*(3.0./5.0e+1)-psi_dot.*t25.*t90.*(3.0./5.0e+1)-psi_dot.*t26.*t90.*(3.0./5.0e+1)+psi_dot.*t19.*t98.*(3.0./5.0e+1)-psi_dot.*t27.*t90.*(3.0./5.0e+1)+psi_dot.*t20.*t98.*(3.0./5.0e+1)-psi_dot.*t28.*t90.*(3.0./5.0e+1)+psi_dot.*t21.*t98.*(3.0./5.0e+1)-psi_dot.*t29.*t90.*(3.0./5.0e+1)+psi_dot.*t22.*t98.*(3.0./5.0e+1)-psi_dot.*t30.*t90.*(3.0./5.0e+1)+psi_dot.*t23.*t98.*(3.0./5.0e+1)+psi_dot.*t24.*t98.*(3.0./5.0e+1);
et26 = psi_dot.*t25.*t98.*(3.0./5.0e+1)+psi_dot.*t26.*t98.*(3.0./5.0e+1)+psi_dot.*t27.*t98.*(3.0./5.0e+1)+psi_dot.*t28.*t98.*(3.0./5.0e+1)+psi_dot.*t29.*t98.*(3.0./5.0e+1)+psi_dot.*t30.*t98.*(3.0./5.0e+1)-t4.*t91.*th11_dot.*(3.0./5.0e+1)-t5.*t91.*th12_dot.*(3.0./5.0e+1)-t6.*t91.*th13_dot.*(3.0./5.0e+1)-t4.*t101.*th11_dot.*(3.0./5.0e+1)-t5.*t101.*th12_dot.*(3.0./5.0e+1)-t7.*t91.*th21_dot.*(3.0./5.0e+1)-t6.*t101.*th13_dot.*(3.0./5.0e+1)-t8.*t91.*th22_dot.*(3.0./5.0e+1)-t9.*t91.*th23_dot.*(3.0./5.0e+1)-t7.*t101.*th21_dot.*(3.0./5.0e+1)-t8.*t101.*th22_dot.*(3.0./5.0e+1)-t10.*t91.*th31_dot.*(3.0./5.0e+1)-t9.*t101.*th23_dot.*(3.0./5.0e+1)-t11.*t91.*th32_dot.*(3.0./5.0e+1)-t12.*t91.*th33_dot.*(3.0./5.0e+1)-t10.*t101.*th31_dot.*(3.0./5.0e+1);
et27 = t11.*t101.*th32_dot.*(-3.0./5.0e+1)-t13.*t91.*th41_dot.*(3.0./5.0e+1)-t12.*t101.*th33_dot.*(3.0./5.0e+1)-t14.*t91.*th42_dot.*(3.0./5.0e+1)-t15.*t91.*th43_dot.*(3.0./5.0e+1)-t13.*t101.*th41_dot.*(3.0./5.0e+1)-t14.*t101.*th42_dot.*(3.0./5.0e+1)-t15.*t101.*th43_dot.*(3.0./5.0e+1)-t16.*t88.*zeta_dot.*(1.2e+1./2.5e+1)-phi_dot.*t4.*t16.*t17.*(3.0./5.0e+1)+phi_dot.*t5.*t16.*t17.*(3.0./1.0e+2)+phi_dot.*t6.*t16.*t17.*(3.0./1.0e+2)-phi_dot.*t7.*t16.*t17.*(3.0./5.0e+1)+phi_dot.*t8.*t16.*t17.*(3.0./1.0e+2)+phi_dot.*t9.*t16.*t17.*(3.0./1.0e+2)-phi_dot.*t10.*t16.*t17.*(3.0./5.0e+1)+phi_dot.*t11.*t16.*t17.*(3.0./1.0e+2)+phi_dot.*t12.*t16.*t17.*(3.0./1.0e+2)-phi_dot.*t13.*t16.*t17.*(3.0./5.0e+1)+phi_dot.*t14.*t16.*t17.*(3.0./1.0e+2);
et28 = phi_dot.*t15.*t16.*t17.*(3.0./1.0e+2)-phi_dot.*t5.*t88.*t92.*(3.0./1.0e+2)+phi_dot.*t6.*t88.*t92.*(3.0./1.0e+2)-phi_dot.*t8.*t88.*t92.*(3.0./1.0e+2)+phi_dot.*t9.*t88.*t92.*(3.0./1.0e+2)-phi_dot.*t11.*t88.*t92.*(3.0./1.0e+2)+phi_dot.*t12.*t88.*t92.*(3.0./1.0e+2)-phi_dot.*t14.*t88.*t92.*(3.0./1.0e+2)+phi_dot.*t15.*t88.*t92.*(3.0./1.0e+2)-phi_dot.*t5.*t92.*t100.*(3.0./1.0e+2)+phi_dot.*t6.*t92.*t100.*(3.0./1.0e+2)-phi_dot.*t8.*t92.*t100.*(3.0./1.0e+2)+phi_dot.*t9.*t92.*t100.*(3.0./1.0e+2)-phi_dot.*t11.*t92.*t100.*(3.0./1.0e+2)+phi_dot.*t12.*t92.*t100.*(3.0./1.0e+2)-phi_dot.*t14.*t92.*t100.*(3.0./1.0e+2)+phi_dot.*t15.*t92.*t100.*(3.0./1.0e+2)+psi_dot.*t5.*t91.*t92.*(3.0./1.0e+2)-psi_dot.*t6.*t91.*t92.*(3.0./1.0e+2);
et29 = psi_dot.*t8.*t91.*t92.*(3.0./1.0e+2)-psi_dot.*t9.*t91.*t92.*(3.0./1.0e+2)+psi_dot.*t11.*t91.*t92.*(3.0./1.0e+2)-psi_dot.*t12.*t91.*t92.*(3.0./1.0e+2)+psi_dot.*t14.*t91.*t92.*(3.0./1.0e+2)+psi_dot.*t5.*t92.*t101.*(3.0./1.0e+2)-psi_dot.*t15.*t91.*t92.*(3.0./1.0e+2)-psi_dot.*t6.*t92.*t101.*(3.0./1.0e+2)+psi_dot.*t8.*t92.*t101.*(3.0./1.0e+2)-psi_dot.*t9.*t92.*t101.*(3.0./1.0e+2)+psi_dot.*t11.*t92.*t101.*(3.0./1.0e+2)-psi_dot.*t12.*t92.*t101.*(3.0./1.0e+2)+psi_dot.*t14.*t92.*t101.*(3.0./1.0e+2)-psi_dot.*t15.*t92.*t101.*(3.0./1.0e+2)-t2.*t16.*t19.*th11_dot.*(3.0./5.0e+1)+t2.*t16.*t20.*th12_dot.*(3.0./1.0e+2)+t2.*t16.*t21.*th13_dot.*(3.0./1.0e+2)-t2.*t16.*t22.*th21_dot.*(3.0./5.0e+1)+t2.*t16.*t23.*th22_dot.*(3.0./1.0e+2);
et30 = t2.*t16.*t24.*th23_dot.*(3.0./1.0e+2)-t2.*t16.*t25.*th31_dot.*(3.0./5.0e+1)+t2.*t16.*t26.*th32_dot.*(3.0./1.0e+2)+t2.*t16.*t27.*th33_dot.*(3.0./1.0e+2)-t2.*t16.*t28.*th41_dot.*(3.0./5.0e+1)+t2.*t16.*t29.*th42_dot.*(3.0./1.0e+2)+t2.*t16.*t30.*th43_dot.*(3.0./1.0e+2)+t20.*t90.*t92.*th12_dot.*(3.0./1.0e+2)-t21.*t90.*t92.*th13_dot.*(3.0./1.0e+2)-t20.*t92.*t98.*th12_dot.*(3.0./1.0e+2)+t21.*t92.*t98.*th13_dot.*(3.0./1.0e+2)+t23.*t90.*t92.*th22_dot.*(3.0./1.0e+2)-t24.*t90.*t92.*th23_dot.*(3.0./1.0e+2)-t23.*t92.*t98.*th22_dot.*(3.0./1.0e+2)+t24.*t92.*t98.*th23_dot.*(3.0./1.0e+2)+t26.*t90.*t92.*th32_dot.*(3.0./1.0e+2)-t27.*t90.*t92.*th33_dot.*(3.0./1.0e+2)-t26.*t92.*t98.*th32_dot.*(3.0./1.0e+2)+t27.*t92.*t98.*th33_dot.*(3.0./1.0e+2);
et31 = t29.*t90.*t92.*th42_dot.*(3.0./1.0e+2)-t30.*t90.*t92.*th43_dot.*(3.0./1.0e+2)-t29.*t92.*t98.*th42_dot.*(3.0./1.0e+2)+t30.*t92.*t98.*th43_dot.*(3.0./1.0e+2)-t2.*t4.*t31.*zeta_dot.*(3.0./5.0e+1)+t2.*t5.*t31.*zeta_dot.*(3.0./1.0e+2)+t2.*t6.*t31.*zeta_dot.*(3.0./1.0e+2)-t2.*t7.*t31.*zeta_dot.*(3.0./5.0e+1)+t2.*t8.*t31.*zeta_dot.*(3.0./1.0e+2)+t2.*t9.*t31.*zeta_dot.*(3.0./1.0e+2)-t2.*t10.*t31.*zeta_dot.*(3.0./5.0e+1)+t2.*t11.*t31.*zeta_dot.*(3.0./1.0e+2)+t2.*t12.*t31.*zeta_dot.*(3.0./1.0e+2)-t2.*t13.*t31.*zeta_dot.*(3.0./5.0e+1)+t2.*t14.*t31.*zeta_dot.*(3.0./1.0e+2)+t2.*t15.*t31.*zeta_dot.*(3.0./1.0e+2)-t16.*t19.*t88.*zeta_dot.*(3.0./5.0e+1)-t16.*t20.*t88.*zeta_dot.*(3.0./5.0e+1)-t16.*t21.*t88.*zeta_dot.*(3.0./5.0e+1);
et32 = t16.*t22.*t88.*zeta_dot.*(-3.0./5.0e+1)-t16.*t23.*t88.*zeta_dot.*(3.0./5.0e+1)-t16.*t24.*t88.*zeta_dot.*(3.0./5.0e+1)-t16.*t25.*t88.*zeta_dot.*(3.0./5.0e+1)-t16.*t26.*t88.*zeta_dot.*(3.0./5.0e+1)-t16.*t27.*t88.*zeta_dot.*(3.0./5.0e+1)-t16.*t28.*t88.*zeta_dot.*(3.0./5.0e+1)-t16.*t29.*t88.*zeta_dot.*(3.0./5.0e+1)-t16.*t30.*t88.*zeta_dot.*(3.0./5.0e+1)+t5.*t16.*t89.*t92.*zeta_dot.*(3.0./1.0e+2)-t6.*t16.*t89.*t92.*zeta_dot.*(3.0./1.0e+2)+t8.*t16.*t89.*t92.*zeta_dot.*(3.0./1.0e+2)-t9.*t16.*t89.*t92.*zeta_dot.*(3.0./1.0e+2)+t11.*t16.*t89.*t92.*zeta_dot.*(3.0./1.0e+2)-t12.*t16.*t89.*t92.*zeta_dot.*(3.0./1.0e+2)+t14.*t16.*t89.*t92.*zeta_dot.*(3.0./1.0e+2)-t15.*t16.*t89.*t92.*zeta_dot.*(3.0./1.0e+2);
et33 = t99.*zeta_dot.*(1.2e+1./2.5e+1)-phi_dot.*t16.*t88.*(1.2e+1./2.5e+1)+psi_dot.*t16.*t91.*(1.2e+1./2.5e+1)+t19.*t99.*zeta_dot.*(3.0./5.0e+1)+t20.*t99.*zeta_dot.*(3.0./5.0e+1)+t21.*t99.*zeta_dot.*(3.0./5.0e+1)+t22.*t99.*zeta_dot.*(3.0./5.0e+1)+t23.*t99.*zeta_dot.*(3.0./5.0e+1)+t24.*t99.*zeta_dot.*(3.0./5.0e+1)+t25.*t99.*zeta_dot.*(3.0./5.0e+1)+t26.*t99.*zeta_dot.*(3.0./5.0e+1)+t27.*t99.*zeta_dot.*(3.0./5.0e+1)+t28.*t99.*zeta_dot.*(3.0./5.0e+1)+t29.*t99.*zeta_dot.*(3.0./5.0e+1)+t30.*t99.*zeta_dot.*(3.0./5.0e+1)-phi_dot.*t2.*t4.*t31.*(3.0./5.0e+1)+phi_dot.*t2.*t5.*t31.*(3.0./1.0e+2)+phi_dot.*t2.*t6.*t31.*(3.0./1.0e+2)-phi_dot.*t2.*t7.*t31.*(3.0./5.0e+1)+phi_dot.*t2.*t8.*t31.*(3.0./1.0e+2)+phi_dot.*t2.*t9.*t31.*(3.0./1.0e+2)-phi_dot.*t2.*t10.*t31.*(3.0./5.0e+1);
et34 = phi_dot.*t2.*t11.*t31.*(3.0./1.0e+2)+phi_dot.*t2.*t12.*t31.*(3.0./1.0e+2)-phi_dot.*t2.*t13.*t31.*(3.0./5.0e+1)+phi_dot.*t2.*t14.*t31.*(3.0./1.0e+2)+phi_dot.*t2.*t15.*t31.*(3.0./1.0e+2)-phi_dot.*t16.*t19.*t88.*(3.0./5.0e+1)-phi_dot.*t16.*t20.*t88.*(3.0./5.0e+1)-phi_dot.*t16.*t21.*t88.*(3.0./5.0e+1)-phi_dot.*t16.*t22.*t88.*(3.0./5.0e+1)-phi_dot.*t16.*t23.*t88.*(3.0./5.0e+1)-phi_dot.*t16.*t24.*t88.*(3.0./5.0e+1)-phi_dot.*t16.*t25.*t88.*(3.0./5.0e+1)-phi_dot.*t16.*t26.*t88.*(3.0./5.0e+1)-phi_dot.*t16.*t27.*t88.*(3.0./5.0e+1)-phi_dot.*t16.*t28.*t88.*(3.0./5.0e+1)-phi_dot.*t16.*t29.*t88.*(3.0./5.0e+1)-phi_dot.*t16.*t30.*t88.*(3.0./5.0e+1)+psi_dot.*t16.*t19.*t91.*(3.0./5.0e+1)+psi_dot.*t16.*t20.*t91.*(3.0./5.0e+1)+psi_dot.*t16.*t21.*t91.*(3.0./5.0e+1);
et35 = psi_dot.*t16.*t22.*t91.*(3.0./5.0e+1)+psi_dot.*t16.*t23.*t91.*(3.0./5.0e+1)+psi_dot.*t16.*t24.*t91.*(3.0./5.0e+1)+psi_dot.*t16.*t25.*t91.*(3.0./5.0e+1)+psi_dot.*t16.*t26.*t91.*(3.0./5.0e+1)+psi_dot.*t16.*t27.*t91.*(3.0./5.0e+1)+psi_dot.*t16.*t28.*t91.*(3.0./5.0e+1)+psi_dot.*t16.*t29.*t91.*(3.0./5.0e+1)+psi_dot.*t16.*t30.*t91.*(3.0./5.0e+1)+t17.*t19.*t31.*th11_dot.*(3.0./5.0e+1)-t17.*t20.*t31.*th12_dot.*(3.0./1.0e+2)-t17.*t21.*t31.*th13_dot.*(3.0./1.0e+2)+t17.*t22.*t31.*th21_dot.*(3.0./5.0e+1)-t17.*t23.*t31.*th22_dot.*(3.0./1.0e+2)-t17.*t24.*t31.*th23_dot.*(3.0./1.0e+2)+t17.*t25.*t31.*th31_dot.*(3.0./5.0e+1)-t17.*t26.*t31.*th32_dot.*(3.0./1.0e+2)-t17.*t27.*t31.*th33_dot.*(3.0./1.0e+2)+t17.*t28.*t31.*th41_dot.*(3.0./5.0e+1)-t17.*t29.*t31.*th42_dot.*(3.0./1.0e+2);
et36 = t4.*t16.*t90.*th11_dot.*(-3.0./5.0e+1)-t17.*t30.*t31.*th43_dot.*(3.0./1.0e+2)-t5.*t16.*t90.*th12_dot.*(3.0./5.0e+1)-t6.*t16.*t90.*th13_dot.*(3.0./5.0e+1)-t7.*t16.*t90.*th21_dot.*(3.0./5.0e+1)-t8.*t16.*t90.*th22_dot.*(3.0./5.0e+1)-t9.*t16.*t90.*th23_dot.*(3.0./5.0e+1)-t10.*t16.*t90.*th31_dot.*(3.0./5.0e+1)-t11.*t16.*t90.*th32_dot.*(3.0./5.0e+1)-t12.*t16.*t90.*th33_dot.*(3.0./5.0e+1)-t13.*t16.*t90.*th41_dot.*(3.0./5.0e+1)-t14.*t16.*t90.*th42_dot.*(3.0./5.0e+1)-t15.*t16.*t90.*th43_dot.*(3.0./5.0e+1)-t4.*t16.*t17.*zeta_dot.*(3.0./5.0e+1)+t5.*t16.*t17.*zeta_dot.*(3.0./1.0e+2)+t6.*t16.*t17.*zeta_dot.*(3.0./1.0e+2)-t7.*t16.*t17.*zeta_dot.*(3.0./5.0e+1)+t8.*t16.*t17.*zeta_dot.*(3.0./1.0e+2)+t9.*t16.*t17.*zeta_dot.*(3.0./1.0e+2);
et37 = t10.*t16.*t17.*zeta_dot.*(-3.0./5.0e+1)+t11.*t16.*t17.*zeta_dot.*(3.0./1.0e+2)+t12.*t16.*t17.*zeta_dot.*(3.0./1.0e+2)-t13.*t16.*t17.*zeta_dot.*(3.0./5.0e+1)+t14.*t16.*t17.*zeta_dot.*(3.0./1.0e+2)+t15.*t16.*t17.*zeta_dot.*(3.0./1.0e+2)-t5.*t92.*t100.*zeta_dot.*(3.0./1.0e+2)+t6.*t92.*t100.*zeta_dot.*(3.0./1.0e+2)-t8.*t92.*t100.*zeta_dot.*(3.0./1.0e+2)+t9.*t92.*t100.*zeta_dot.*(3.0./1.0e+2)-t11.*t92.*t100.*zeta_dot.*(3.0./1.0e+2)+t12.*t92.*t100.*zeta_dot.*(3.0./1.0e+2)-t14.*t92.*t100.*zeta_dot.*(3.0./1.0e+2)+t15.*t92.*t100.*zeta_dot.*(3.0./1.0e+2)+phi_dot.*t5.*t16.*t89.*t92.*(3.0./1.0e+2)-phi_dot.*t6.*t16.*t89.*t92.*(3.0./1.0e+2)+phi_dot.*t8.*t16.*t89.*t92.*(3.0./1.0e+2)-phi_dot.*t9.*t16.*t89.*t92.*(3.0./1.0e+2);
et38 = phi_dot.*t11.*t16.*t89.*t92.*(3.0./1.0e+2)-phi_dot.*t12.*t16.*t89.*t92.*(3.0./1.0e+2)+phi_dot.*t14.*t16.*t89.*t92.*(3.0./1.0e+2)-phi_dot.*t15.*t16.*t89.*t92.*(3.0./1.0e+2)+psi_dot.*t5.*t16.*t90.*t92.*(3.0./1.0e+2)-psi_dot.*t6.*t16.*t90.*t92.*(3.0./1.0e+2)+psi_dot.*t8.*t16.*t90.*t92.*(3.0./1.0e+2)-psi_dot.*t9.*t16.*t90.*t92.*(3.0./1.0e+2)+psi_dot.*t11.*t16.*t90.*t92.*(3.0./1.0e+2)-psi_dot.*t12.*t16.*t90.*t92.*(3.0./1.0e+2)+psi_dot.*t14.*t16.*t90.*t92.*(3.0./1.0e+2)-psi_dot.*t15.*t16.*t90.*t92.*(3.0./1.0e+2)-t16.*t20.*t91.*t92.*th12_dot.*(3.0./1.0e+2)+t16.*t21.*t91.*t92.*th13_dot.*(3.0./1.0e+2)-t16.*t23.*t91.*t92.*th22_dot.*(3.0./1.0e+2)+t16.*t24.*t91.*t92.*th23_dot.*(3.0./1.0e+2)-t16.*t26.*t91.*t92.*th32_dot.*(3.0./1.0e+2);
et39 = t16.*t27.*t91.*t92.*th33_dot.*(3.0./1.0e+2)-t16.*t29.*t91.*t92.*th42_dot.*(3.0./1.0e+2)+t16.*t30.*t91.*t92.*th43_dot.*(3.0./1.0e+2);
et40 = phi_dot.*t90.*(-1.2e+1./2.5e+1)+phi_dot.*t98.*(1.2e+1./2.5e+1)-psi_dot.*t89.*(1.2e+1./2.5e+1)+psi_dot.*t99.*(1.2e+1./2.5e+1)-phi_dot.*t19.*t90.*(3.0./5.0e+1)-phi_dot.*t20.*t90.*(3.0./5.0e+1)-phi_dot.*t21.*t90.*(3.0./5.0e+1)-phi_dot.*t22.*t90.*(3.0./5.0e+1)-phi_dot.*t23.*t90.*(3.0./5.0e+1)-phi_dot.*t24.*t90.*(3.0./5.0e+1)-phi_dot.*t25.*t90.*(3.0./5.0e+1)-phi_dot.*t26.*t90.*(3.0./5.0e+1)+phi_dot.*t19.*t98.*(3.0./5.0e+1)-phi_dot.*t27.*t90.*(3.0./5.0e+1)+phi_dot.*t20.*t98.*(3.0./5.0e+1)-phi_dot.*t28.*t90.*(3.0./5.0e+1)+phi_dot.*t21.*t98.*(3.0./5.0e+1)-phi_dot.*t29.*t90.*(3.0./5.0e+1)+phi_dot.*t22.*t98.*(3.0./5.0e+1)-phi_dot.*t30.*t90.*(3.0./5.0e+1)+phi_dot.*t23.*t98.*(3.0./5.0e+1)+phi_dot.*t24.*t98.*(3.0./5.0e+1)+phi_dot.*t25.*t98.*(3.0./5.0e+1);
et41 = phi_dot.*t26.*t98.*(3.0./5.0e+1)+phi_dot.*t27.*t98.*(3.0./5.0e+1)+phi_dot.*t28.*t98.*(3.0./5.0e+1)+phi_dot.*t29.*t98.*(3.0./5.0e+1)+phi_dot.*t30.*t98.*(3.0./5.0e+1)-psi_dot.*t19.*t89.*(3.0./5.0e+1)-psi_dot.*t20.*t89.*(3.0./5.0e+1)-psi_dot.*t21.*t89.*(3.0./5.0e+1)-psi_dot.*t22.*t89.*(3.0./5.0e+1)-psi_dot.*t23.*t89.*(3.0./5.0e+1)-psi_dot.*t24.*t89.*(3.0./5.0e+1)-psi_dot.*t25.*t89.*(3.0./5.0e+1)-psi_dot.*t26.*t89.*(3.0./5.0e+1)-psi_dot.*t27.*t89.*(3.0./5.0e+1)-psi_dot.*t28.*t89.*(3.0./5.0e+1)+psi_dot.*t19.*t99.*(3.0./5.0e+1)-psi_dot.*t29.*t89.*(3.0./5.0e+1)+psi_dot.*t20.*t99.*(3.0./5.0e+1)-psi_dot.*t30.*t89.*(3.0./5.0e+1)+psi_dot.*t21.*t99.*(3.0./5.0e+1)+psi_dot.*t22.*t99.*(3.0./5.0e+1)+psi_dot.*t23.*t99.*(3.0./5.0e+1)+psi_dot.*t24.*t99.*(3.0./5.0e+1);
et42 = psi_dot.*t25.*t99.*(3.0./5.0e+1)+psi_dot.*t26.*t99.*(3.0./5.0e+1)+psi_dot.*t27.*t99.*(3.0./5.0e+1)+psi_dot.*t28.*t99.*(3.0./5.0e+1)+psi_dot.*t29.*t99.*(3.0./5.0e+1)+psi_dot.*t30.*t99.*(3.0./5.0e+1)+t4.*t88.*th11_dot.*(3.0./5.0e+1)+t5.*t88.*th12_dot.*(3.0./5.0e+1)+t6.*t88.*th13_dot.*(3.0./5.0e+1)+t4.*t100.*th11_dot.*(3.0./5.0e+1)+t7.*t88.*th21_dot.*(3.0./5.0e+1)+t5.*t100.*th12_dot.*(3.0./5.0e+1)+t8.*t88.*th22_dot.*(3.0./5.0e+1)+t6.*t100.*th13_dot.*(3.0./5.0e+1)+t9.*t88.*th23_dot.*(3.0./5.0e+1)+t7.*t100.*th21_dot.*(3.0./5.0e+1)+t10.*t88.*th31_dot.*(3.0./5.0e+1)+t8.*t100.*th22_dot.*(3.0./5.0e+1)+t11.*t88.*th32_dot.*(3.0./5.0e+1)+t9.*t100.*th23_dot.*(3.0./5.0e+1)+t12.*t88.*th33_dot.*(3.0./5.0e+1)+t10.*t100.*th31_dot.*(3.0./5.0e+1)+t13.*t88.*th41_dot.*(3.0./5.0e+1)+t11.*t100.*th32_dot.*(3.0./5.0e+1)+t14.*t88.*th42_dot.*(3.0./5.0e+1);
et43 = t12.*t100.*th33_dot.*(3.0./5.0e+1)+t15.*t88.*th43_dot.*(3.0./5.0e+1)+t13.*t100.*th41_dot.*(3.0./5.0e+1)+t14.*t100.*th42_dot.*(3.0./5.0e+1)+t15.*t100.*th43_dot.*(3.0./5.0e+1)+t16.*t91.*zeta_dot.*(1.2e+1./2.5e+1)+phi_dot.*t5.*t91.*t92.*(3.0./1.0e+2)-phi_dot.*t6.*t91.*t92.*(3.0./1.0e+2)+phi_dot.*t8.*t91.*t92.*(3.0./1.0e+2)-phi_dot.*t9.*t91.*t92.*(3.0./1.0e+2)+phi_dot.*t11.*t91.*t92.*(3.0./1.0e+2)-phi_dot.*t12.*t91.*t92.*(3.0./1.0e+2)+phi_dot.*t14.*t91.*t92.*(3.0./1.0e+2)+phi_dot.*t5.*t92.*t101.*(3.0./1.0e+2)-phi_dot.*t15.*t91.*t92.*(3.0./1.0e+2)-phi_dot.*t6.*t92.*t101.*(3.0./1.0e+2)+phi_dot.*t8.*t92.*t101.*(3.0./1.0e+2)-phi_dot.*t9.*t92.*t101.*(3.0./1.0e+2)+phi_dot.*t11.*t92.*t101.*(3.0./1.0e+2)-phi_dot.*t12.*t92.*t101.*(3.0./1.0e+2);
et44 = phi_dot.*t14.*t92.*t101.*(3.0./1.0e+2)-phi_dot.*t15.*t92.*t101.*(3.0./1.0e+2)-psi_dot.*t5.*t88.*t92.*(3.0./1.0e+2)+psi_dot.*t6.*t88.*t92.*(3.0./1.0e+2)-psi_dot.*t8.*t88.*t92.*(3.0./1.0e+2)+psi_dot.*t9.*t88.*t92.*(3.0./1.0e+2)-psi_dot.*t11.*t88.*t92.*(3.0./1.0e+2)+psi_dot.*t12.*t88.*t92.*(3.0./1.0e+2)-psi_dot.*t14.*t88.*t92.*(3.0./1.0e+2)+psi_dot.*t15.*t88.*t92.*(3.0./1.0e+2)-psi_dot.*t5.*t92.*t100.*(3.0./1.0e+2)+psi_dot.*t6.*t92.*t100.*(3.0./1.0e+2)-psi_dot.*t8.*t92.*t100.*(3.0./1.0e+2)+psi_dot.*t9.*t92.*t100.*(3.0./1.0e+2)-psi_dot.*t11.*t92.*t100.*(3.0./1.0e+2)+psi_dot.*t12.*t92.*t100.*(3.0./1.0e+2)-psi_dot.*t14.*t92.*t100.*(3.0./1.0e+2)+psi_dot.*t15.*t92.*t100.*(3.0./1.0e+2)+t20.*t89.*t92.*th12_dot.*(3.0./1.0e+2);
et45 = t21.*t89.*t92.*th13_dot.*(-3.0./1.0e+2)-t20.*t92.*t99.*th12_dot.*(3.0./1.0e+2)+t21.*t92.*t99.*th13_dot.*(3.0./1.0e+2)+t23.*t89.*t92.*th22_dot.*(3.0./1.0e+2)-t24.*t89.*t92.*th23_dot.*(3.0./1.0e+2)-t23.*t92.*t99.*th22_dot.*(3.0./1.0e+2)+t24.*t92.*t99.*th23_dot.*(3.0./1.0e+2)+t26.*t89.*t92.*th32_dot.*(3.0./1.0e+2)-t27.*t89.*t92.*th33_dot.*(3.0./1.0e+2)-t26.*t92.*t99.*th32_dot.*(3.0./1.0e+2)+t27.*t92.*t99.*th33_dot.*(3.0./1.0e+2)+t29.*t89.*t92.*th42_dot.*(3.0./1.0e+2)-t30.*t89.*t92.*th43_dot.*(3.0./1.0e+2)-t29.*t92.*t99.*th42_dot.*(3.0./1.0e+2)+t30.*t92.*t99.*th43_dot.*(3.0./1.0e+2)+t16.*t19.*t91.*zeta_dot.*(3.0./5.0e+1)+t16.*t20.*t91.*zeta_dot.*(3.0./5.0e+1)+t16.*t21.*t91.*zeta_dot.*(3.0./5.0e+1)+t16.*t22.*t91.*zeta_dot.*(3.0./5.0e+1);
et46 = t16.*t23.*t91.*zeta_dot.*(3.0./5.0e+1)+t16.*t24.*t91.*zeta_dot.*(3.0./5.0e+1)+t16.*t25.*t91.*zeta_dot.*(3.0./5.0e+1)+t16.*t26.*t91.*zeta_dot.*(3.0./5.0e+1)+t16.*t27.*t91.*zeta_dot.*(3.0./5.0e+1)+t16.*t28.*t91.*zeta_dot.*(3.0./5.0e+1)+t16.*t29.*t91.*zeta_dot.*(3.0./5.0e+1)+t16.*t30.*t91.*zeta_dot.*(3.0./5.0e+1)+t5.*t16.*t90.*t92.*zeta_dot.*(3.0./1.0e+2)-t6.*t16.*t90.*t92.*zeta_dot.*(3.0./1.0e+2)+t8.*t16.*t90.*t92.*zeta_dot.*(3.0./1.0e+2)-t9.*t16.*t90.*t92.*zeta_dot.*(3.0./1.0e+2)+t11.*t16.*t90.*t92.*zeta_dot.*(3.0./1.0e+2)-t12.*t16.*t90.*t92.*zeta_dot.*(3.0./1.0e+2)+t14.*t16.*t90.*t92.*zeta_dot.*(3.0./1.0e+2)-t15.*t16.*t90.*t92.*zeta_dot.*(3.0./1.0e+2);
et47 = psi_dot.*t18.*t31.*(-1.2e+1./2.5e+1)+t16.*t19.*th11_dot.*(3.0./5.0e+1)-t16.*t20.*th12_dot.*(3.0./1.0e+2)-t16.*t21.*th13_dot.*(3.0./1.0e+2)+t16.*t22.*th21_dot.*(3.0./5.0e+1)-t16.*t23.*th22_dot.*(3.0./1.0e+2)-t16.*t24.*th23_dot.*(3.0./1.0e+2)+t16.*t25.*th31_dot.*(3.0./5.0e+1)-t16.*t26.*th32_dot.*(3.0./1.0e+2)-t16.*t27.*th33_dot.*(3.0./1.0e+2)+t16.*t28.*th41_dot.*(3.0./5.0e+1)-t16.*t29.*th42_dot.*(3.0./1.0e+2)-t16.*t30.*th43_dot.*(3.0./1.0e+2)+t3.*t16.*zeta_dot.*(1.2e+1./2.5e+1)+t4.*t31.*zeta_dot.*(3.0./5.0e+1)-t5.*t31.*zeta_dot.*(3.0./1.0e+2)-t6.*t31.*zeta_dot.*(3.0./1.0e+2)+t7.*t31.*zeta_dot.*(3.0./5.0e+1)-t8.*t31.*zeta_dot.*(3.0./1.0e+2)-t9.*t31.*zeta_dot.*(3.0./1.0e+2)+t10.*t31.*zeta_dot.*(3.0./5.0e+1);
et48 = t11.*t31.*zeta_dot.*(-3.0./1.0e+2)-t12.*t31.*zeta_dot.*(3.0./1.0e+2)+t13.*t31.*zeta_dot.*(3.0./5.0e+1)-t14.*t31.*zeta_dot.*(3.0./1.0e+2)-t15.*t31.*zeta_dot.*(3.0./1.0e+2)-psi_dot.*t18.*t19.*t31.*(3.0./5.0e+1)-psi_dot.*t18.*t20.*t31.*(3.0./5.0e+1)-psi_dot.*t18.*t21.*t31.*(3.0./5.0e+1)-psi_dot.*t18.*t22.*t31.*(3.0./5.0e+1)-psi_dot.*t18.*t23.*t31.*(3.0./5.0e+1)-psi_dot.*t18.*t24.*t31.*(3.0./5.0e+1)-psi_dot.*t18.*t25.*t31.*(3.0./5.0e+1)-psi_dot.*t18.*t26.*t31.*(3.0./5.0e+1)-psi_dot.*t18.*t27.*t31.*(3.0./5.0e+1)-psi_dot.*t18.*t28.*t31.*(3.0./5.0e+1)-psi_dot.*t18.*t29.*t31.*(3.0./5.0e+1)-psi_dot.*t18.*t30.*t31.*(3.0./5.0e+1)+t3.*t4.*t31.*th11_dot.*(3.0./5.0e+1)+t3.*t5.*t31.*th12_dot.*(3.0./5.0e+1)+t3.*t6.*t31.*th13_dot.*(3.0./5.0e+1);
et49 = t3.*t7.*t31.*th21_dot.*(3.0./5.0e+1)+t3.*t8.*t31.*th22_dot.*(3.0./5.0e+1)+t3.*t9.*t31.*th23_dot.*(3.0./5.0e+1)+t3.*t10.*t31.*th31_dot.*(3.0./5.0e+1)+t3.*t11.*t31.*th32_dot.*(3.0./5.0e+1)+t3.*t12.*t31.*th33_dot.*(3.0./5.0e+1)+t3.*t13.*t31.*th41_dot.*(3.0./5.0e+1)+t3.*t14.*t31.*th42_dot.*(3.0./5.0e+1)+t3.*t15.*t31.*th43_dot.*(3.0./5.0e+1)+t3.*t16.*t19.*zeta_dot.*(3.0./5.0e+1)+t3.*t16.*t20.*zeta_dot.*(3.0./5.0e+1)+t3.*t16.*t21.*zeta_dot.*(3.0./5.0e+1)+t3.*t16.*t22.*zeta_dot.*(3.0./5.0e+1)+t3.*t16.*t23.*zeta_dot.*(3.0./5.0e+1)+t3.*t16.*t24.*zeta_dot.*(3.0./5.0e+1)+t3.*t16.*t25.*zeta_dot.*(3.0./5.0e+1)+t3.*t16.*t26.*zeta_dot.*(3.0./5.0e+1)+t3.*t16.*t27.*zeta_dot.*(3.0./5.0e+1)+t3.*t16.*t28.*zeta_dot.*(3.0./5.0e+1)+t3.*t16.*t29.*zeta_dot.*(3.0./5.0e+1)+t3.*t16.*t30.*zeta_dot.*(3.0./5.0e+1);
et50 = psi_dot.*t3.*t5.*t31.*t92.*(-3.0./1.0e+2)+psi_dot.*t3.*t6.*t31.*t92.*(3.0./1.0e+2)-psi_dot.*t3.*t8.*t31.*t92.*(3.0./1.0e+2)+psi_dot.*t3.*t9.*t31.*t92.*(3.0./1.0e+2)-psi_dot.*t3.*t11.*t31.*t92.*(3.0./1.0e+2)+psi_dot.*t3.*t12.*t31.*t92.*(3.0./1.0e+2)-psi_dot.*t3.*t14.*t31.*t92.*(3.0./1.0e+2)+psi_dot.*t3.*t15.*t31.*t92.*(3.0./1.0e+2)+t18.*t20.*t31.*t92.*th12_dot.*(3.0./1.0e+2)-t18.*t21.*t31.*t92.*th13_dot.*(3.0./1.0e+2)+t18.*t23.*t31.*t92.*th22_dot.*(3.0./1.0e+2)-t18.*t24.*t31.*t92.*th23_dot.*(3.0./1.0e+2)+t18.*t26.*t31.*t92.*th32_dot.*(3.0./1.0e+2)-t18.*t27.*t31.*t92.*th33_dot.*(3.0./1.0e+2)+t18.*t29.*t31.*t92.*th42_dot.*(3.0./1.0e+2)-t18.*t30.*t31.*t92.*th43_dot.*(3.0./1.0e+2)-t5.*t16.*t18.*t92.*zeta_dot.*(3.0./1.0e+2);
et51 = t6.*t16.*t18.*t92.*zeta_dot.*(3.0./1.0e+2)-t8.*t16.*t18.*t92.*zeta_dot.*(3.0./1.0e+2)+t9.*t16.*t18.*t92.*zeta_dot.*(3.0./1.0e+2)-t11.*t16.*t18.*t92.*zeta_dot.*(3.0./1.0e+2)+t12.*t16.*t18.*t92.*zeta_dot.*(3.0./1.0e+2)-t14.*t16.*t18.*t92.*zeta_dot.*(3.0./1.0e+2)+t15.*t16.*t18.*t92.*zeta_dot.*(3.0./1.0e+2);
et52 = psi_dot.*t3.*t16.*(1.2e+1./2.5e+1)-t18.*t31.*zeta_dot.*(1.2e+1./2.5e+1)+psi_dot.*t3.*t16.*t19.*(3.0./5.0e+1)+psi_dot.*t3.*t16.*t20.*(3.0./5.0e+1)+psi_dot.*t3.*t16.*t21.*(3.0./5.0e+1)+psi_dot.*t3.*t16.*t22.*(3.0./5.0e+1)+psi_dot.*t3.*t16.*t23.*(3.0./5.0e+1)+psi_dot.*t3.*t16.*t24.*(3.0./5.0e+1)+psi_dot.*t3.*t16.*t25.*(3.0./5.0e+1)+psi_dot.*t3.*t16.*t26.*(3.0./5.0e+1)+psi_dot.*t3.*t16.*t27.*(3.0./5.0e+1)+psi_dot.*t3.*t16.*t28.*(3.0./5.0e+1)+psi_dot.*t3.*t16.*t29.*(3.0./5.0e+1)+psi_dot.*t3.*t16.*t30.*(3.0./5.0e+1)+t4.*t16.*t18.*th11_dot.*(3.0./5.0e+1)+t5.*t16.*t18.*th12_dot.*(3.0./5.0e+1)+t6.*t16.*t18.*th13_dot.*(3.0./5.0e+1)+t7.*t16.*t18.*th21_dot.*(3.0./5.0e+1)+t8.*t16.*t18.*th22_dot.*(3.0./5.0e+1)+t9.*t16.*t18.*th23_dot.*(3.0./5.0e+1)+t10.*t16.*t18.*th31_dot.*(3.0./5.0e+1)+t11.*t16.*t18.*th32_dot.*(3.0./5.0e+1);
et53 = t12.*t16.*t18.*th33_dot.*(3.0./5.0e+1)+t13.*t16.*t18.*th41_dot.*(3.0./5.0e+1)+t14.*t16.*t18.*th42_dot.*(3.0./5.0e+1)+t15.*t16.*t18.*th43_dot.*(3.0./5.0e+1)-t18.*t19.*t31.*zeta_dot.*(3.0./5.0e+1)-t18.*t20.*t31.*zeta_dot.*(3.0./5.0e+1)-t18.*t21.*t31.*zeta_dot.*(3.0./5.0e+1)-t18.*t22.*t31.*zeta_dot.*(3.0./5.0e+1)-t18.*t23.*t31.*zeta_dot.*(3.0./5.0e+1)-t18.*t24.*t31.*zeta_dot.*(3.0./5.0e+1)-t18.*t25.*t31.*zeta_dot.*(3.0./5.0e+1)-t18.*t26.*t31.*zeta_dot.*(3.0./5.0e+1)-t18.*t27.*t31.*zeta_dot.*(3.0./5.0e+1)-t18.*t28.*t31.*zeta_dot.*(3.0./5.0e+1)-t18.*t29.*t31.*zeta_dot.*(3.0./5.0e+1)-t18.*t30.*t31.*zeta_dot.*(3.0./5.0e+1)-psi_dot.*t5.*t16.*t18.*t92.*(3.0./1.0e+2)+psi_dot.*t6.*t16.*t18.*t92.*(3.0./1.0e+2)-psi_dot.*t8.*t16.*t18.*t92.*(3.0./1.0e+2);
et54 = psi_dot.*t9.*t16.*t18.*t92.*(3.0./1.0e+2)-psi_dot.*t11.*t16.*t18.*t92.*(3.0./1.0e+2)+psi_dot.*t12.*t16.*t18.*t92.*(3.0./1.0e+2)-psi_dot.*t14.*t16.*t18.*t92.*(3.0./1.0e+2)+psi_dot.*t15.*t16.*t18.*t92.*(3.0./1.0e+2)-t3.*t16.*t20.*t92.*th12_dot.*(3.0./1.0e+2)+t3.*t16.*t21.*t92.*th13_dot.*(3.0./1.0e+2)-t3.*t16.*t23.*t92.*th22_dot.*(3.0./1.0e+2)+t3.*t16.*t24.*t92.*th23_dot.*(3.0./1.0e+2)-t3.*t16.*t26.*t92.*th32_dot.*(3.0./1.0e+2)+t3.*t16.*t27.*t92.*th33_dot.*(3.0./1.0e+2)-t3.*t16.*t29.*t92.*th42_dot.*(3.0./1.0e+2)+t3.*t16.*t30.*t92.*th43_dot.*(3.0./1.0e+2)-t3.*t5.*t31.*t92.*zeta_dot.*(3.0./1.0e+2)+t3.*t6.*t31.*t92.*zeta_dot.*(3.0./1.0e+2)-t3.*t8.*t31.*t92.*zeta_dot.*(3.0./1.0e+2)+t3.*t9.*t31.*t92.*zeta_dot.*(3.0./1.0e+2);
et55 = t3.*t11.*t31.*t92.*zeta_dot.*(-3.0./1.0e+2)+t3.*t12.*t31.*t92.*zeta_dot.*(3.0./1.0e+2)-t3.*t14.*t31.*t92.*zeta_dot.*(3.0./1.0e+2)+t3.*t15.*t31.*t92.*zeta_dot.*(3.0./1.0e+2);
et56 = psi_dot.*t74.*(-1.5428125e-1)+t4.*th11_dot.*4.5e-3+t5.*th12_dot.*4.5e-3+t6.*th13_dot.*4.5e-3+t7.*th21_dot.*4.5e-3+t8.*th22_dot.*4.5e-3-t19.*th11_dot.*(3.0./2.0e+2)+t9.*th23_dot.*4.5e-3-t20.*th12_dot.*9.375e-4-t21.*th13_dot.*9.375e-4+t10.*th31_dot.*4.5e-3+t11.*th32_dot.*4.5e-3-t22.*th21_dot.*(3.0./2.0e+2)+t12.*th33_dot.*4.5e-3-t23.*th22_dot.*9.375e-4-t24.*th23_dot.*9.375e-4+t13.*th41_dot.*4.5e-3+t14.*th42_dot.*4.5e-3+t25.*th31_dot.*(3.0./5.0e+2)+t15.*th43_dot.*4.5e-3;
et57 = t26.*th32_dot.*(-1.14375e-2)-t27.*th33_dot.*1.14375e-2+t28.*th41_dot.*(3.0./5.0e+2)-t29.*th42_dot.*1.14375e-2-t30.*th43_dot.*1.14375e-2+(t75.*th11_dot)./7.5e+2+(t76.*th12_dot)./3.0e+3+(t77.*th13_dot)./3.0e+3+(t78.*th21_dot)./7.5e+2+(t79.*th22_dot)./3.0e+3+(t80.*th23_dot)./3.0e+3+(t81.*th31_dot)./7.5e+2+(t82.*th32_dot)./3.0e+3+(t83.*th33_dot)./3.0e+3+(t84.*th41_dot)./7.5e+2+(t85.*th42_dot)./3.0e+3+(t86.*th43_dot)./3.0e+3-t87.*zeta_dot.*1.5428125e-1+psi_dot.*t19.*t46.*1.05e-2;
et58 = psi_dot.*t20.*t46.*1.05e-2+psi_dot.*t21.*t46.*1.05e-2-psi_dot.*t22.*t46.*1.05e-2-psi_dot.*t23.*t46.*1.05e-2-psi_dot.*t24.*t46.*1.05e-2-psi_dot.*t25.*t46.*1.05e-2-psi_dot.*t26.*t46.*1.05e-2-psi_dot.*t27.*t46.*1.05e-2+psi_dot.*t28.*t46.*1.05e-2+psi_dot.*t29.*t46.*1.05e-2+psi_dot.*t30.*t46.*1.05e-2-psi_dot.*t5.*t74.*3.375e-3-psi_dot.*t6.*t74.*3.375e-3-psi_dot.*t8.*t74.*3.375e-3-psi_dot.*t9.*t74.*3.375e-3-psi_dot.*t11.*t74.*3.375e-3-psi_dot.*t12.*t74.*3.375e-3;
et59 = psi_dot.*t14.*t74.*(-3.375e-3)-psi_dot.*t15.*t74.*3.375e-3+psi_dot.*t19.*t74.*(3.0./1.0e+3)+psi_dot.*t20.*t74.*(3.0./1.0e+3)+psi_dot.*t21.*t74.*(3.0./1.0e+3)+psi_dot.*t22.*t74.*(3.0./1.0e+3)+psi_dot.*t23.*t74.*(3.0./1.0e+3)+psi_dot.*t24.*t74.*(3.0./1.0e+3)+psi_dot.*t25.*t74.*(3.0./1.0e+3)+psi_dot.*t26.*t74.*(3.0./1.0e+3)+psi_dot.*t27.*t74.*(3.0./1.0e+3)+psi_dot.*t28.*t74.*(3.0./1.0e+3)+psi_dot.*t29.*t74.*(3.0./1.0e+3)+psi_dot.*t30.*t74.*(3.0./1.0e+3)-(psi_dot.*t48.*t74)./7.5e+2-psi_dot.*t49.*t74.*2.333333333333333e-3-psi_dot.*t50.*t74.*2.333333333333333e-3-(psi_dot.*t51.*t74)./7.5e+2-psi_dot.*t52.*t74.*2.333333333333333e-3;
et60 = psi_dot.*t53.*t74.*(-2.333333333333333e-3)-(psi_dot.*t54.*t74)./7.5e+2-psi_dot.*t55.*t74.*2.333333333333333e-3-psi_dot.*t56.*t74.*2.333333333333333e-3-(psi_dot.*t57.*t74)./7.5e+2-psi_dot.*t58.*t74.*2.333333333333333e-3-psi_dot.*t59.*t74.*2.333333333333333e-3-psi_dot.*t72.*t74.*1.5428125e-1+t3.*t72.*t153+t3.*t72.*t154+t46.*t92.*t294+t46.*t92.*t296+t46.*t92.*t298+t46.*t92.*t300-t4.*t46.*th11_dot.*1.5e-3-t5.*t46.*th12_dot.*1.5e-3-t6.*t46.*th13_dot.*1.5e-3-t7.*t46.*th21_dot.*1.5e-3-t8.*t46.*th22_dot.*1.5e-3-t9.*t46.*th23_dot.*1.5e-3-t20.*t46.*th12_dot.*1.6875e-3;
et61 = t21.*t46.*th13_dot.*(-1.6875e-3)-t4.*t72.*th11_dot.*1.5e-3-t10.*t46.*th31_dot.*1.5e-3+t4.*t74.*th11_dot.*5.25e-3-t5.*t72.*th12_dot.*1.5e-3-t11.*t46.*th32_dot.*1.5e-3+t5.*t74.*th12_dot.*5.25e-3-t6.*t72.*th13_dot.*1.5e-3-t12.*t46.*th33_dot.*1.5e-3-t23.*t46.*th22_dot.*1.6875e-3+t6.*t74.*th13_dot.*5.25e-3-t24.*t46.*th23_dot.*1.6875e-3-t7.*t72.*th21_dot.*1.5e-3-t13.*t46.*th41_dot.*1.5e-3-t7.*t74.*th21_dot.*5.25e-3-t8.*t72.*th22_dot.*1.5e-3-t14.*t46.*th42_dot.*1.5e-3;
et62 = t19.*t72.*th11_dot.*(-3.0./2.0e+2)-t8.*t74.*th22_dot.*5.25e-3-t9.*t72.*th23_dot.*1.5e-3-t15.*t46.*th43_dot.*1.5e-3+t20.*t72.*th12_dot.*5.8125e-3-t26.*t46.*th32_dot.*1.6875e-3-t9.*t74.*th23_dot.*5.25e-3+t21.*t72.*th13_dot.*5.8125e-3-t27.*t46.*th33_dot.*1.6875e-3-t10.*t72.*th31_dot.*1.5e-3-t10.*t74.*th31_dot.*5.25e-3-t11.*t72.*th32_dot.*1.5e-3-t22.*t72.*th21_dot.*(3.0./2.0e+2)-t11.*t74.*th32_dot.*5.25e-3-t12.*t72.*th33_dot.*1.5e-3+t23.*t72.*th22_dot.*5.8125e-3;
et63 = t29.*t46.*th42_dot.*(-1.6875e-3)-t12.*t74.*th33_dot.*5.25e-3+t24.*t72.*th23_dot.*5.8125e-3-t30.*t46.*th43_dot.*1.6875e-3-t20.*t92.*th12_dot.*7.875e-3-t13.*t72.*th41_dot.*1.5e-3+t21.*t92.*th13_dot.*7.875e-3+t13.*t74.*th41_dot.*5.25e-3-t14.*t72.*th42_dot.*1.5e-3+t25.*t72.*th31_dot.*(3.0./5.0e+2)+t14.*t74.*th42_dot.*5.25e-3-t15.*t72.*th43_dot.*1.5e-3-t26.*t72.*th32_dot.*(3.0./6.4e+2)+t15.*t74.*th43_dot.*5.25e-3-t27.*t72.*th33_dot.*(3.0./6.4e+2)-(t46.*t75.*th11_dot)./7.5e+2-t46.*t76.*th12_dot.*2.333333333333333e-3;
et64 = t46.*t77.*th13_dot.*(-2.333333333333333e-3)+t23.*t92.*th22_dot.*7.875e-3-t24.*t92.*th23_dot.*7.875e-3+t28.*t72.*th41_dot.*(3.0./5.0e+2)-t29.*t72.*th42_dot.*(3.0./6.4e+2)-t30.*t72.*th43_dot.*(3.0./6.4e+2)-(t46.*t78.*th21_dot)./7.5e+2-t46.*t79.*th22_dot.*2.333333333333333e-3-t46.*t80.*th23_dot.*2.333333333333333e-3+t26.*t92.*th32_dot.*7.875e-3-t27.*t92.*th33_dot.*7.875e-3-(t46.*t81.*th31_dot)./7.5e+2-(t72.*t75.*th11_dot)./2.5e+2-t46.*t82.*th32_dot.*2.333333333333333e-3-(t72.*t76.*th12_dot)./1.0e+3-t46.*t83.*th33_dot.*2.333333333333333e-3-(t72.*t77.*th13_dot)./1.0e+3-t29.*t92.*th42_dot.*7.875e-3;
et65 = t30.*t92.*th43_dot.*7.875e-3-(t46.*t84.*th41_dot)./7.5e+2-(t72.*t78.*th21_dot)./2.5e+2-t46.*t85.*th42_dot.*2.333333333333333e-3-(t72.*t79.*th22_dot)./1.0e+3-t46.*t86.*th43_dot.*2.333333333333333e-3-(t72.*t80.*th23_dot)./1.0e+3-(t72.*t81.*th31_dot)./2.5e+2-(t72.*t82.*th32_dot)./1.0e+3-(t72.*t83.*th33_dot)./1.0e+3-(t72.*t84.*th41_dot)./2.5e+2-(t72.*t85.*th42_dot)./1.0e+3-(t72.*t86.*th43_dot)./1.0e+3-t4.*t87.*zeta_dot.*(3.0./1.0e+2)+t5.*t87.*zeta_dot.*1.1625e-2+t6.*t87.*zeta_dot.*1.1625e-2-t7.*t87.*zeta_dot.*(3.0./1.0e+2)+t8.*t87.*zeta_dot.*1.1625e-2;
et66 = t9.*t87.*zeta_dot.*1.1625e-2+t10.*t87.*zeta_dot.*(3.0./2.5e+2)-t11.*t87.*zeta_dot.*(3.0./3.2e+2)-t12.*t87.*zeta_dot.*(3.0./3.2e+2)+t13.*t87.*zeta_dot.*(3.0./2.5e+2)-t14.*t87.*zeta_dot.*(3.0./3.2e+2)-t15.*t87.*zeta_dot.*(3.0./3.2e+2)+t19.*t87.*zeta_dot.*(3.0./1.0e+3)+t20.*t87.*zeta_dot.*(3.0./1.0e+3)+t21.*t87.*zeta_dot.*(3.0./1.0e+3)+t22.*t87.*zeta_dot.*(3.0./1.0e+3)+t23.*t87.*zeta_dot.*(3.0./1.0e+3)+t24.*t87.*zeta_dot.*(3.0./1.0e+3)+t25.*t87.*zeta_dot.*(3.0./1.0e+3)+t26.*t87.*zeta_dot.*(3.0./1.0e+3)+t27.*t87.*zeta_dot.*(3.0./1.0e+3)+t28.*t87.*zeta_dot.*(3.0./1.0e+3)+t29.*t87.*zeta_dot.*(3.0./1.0e+3)+t30.*t87.*zeta_dot.*(3.0./1.0e+3);
et67 = t46.*t87.*zeta_dot.*(-1.5428125e-1)-(t48.*t87.*zeta_dot)./2.5e+2-(t49.*t87.*zeta_dot)./1.0e+3-(t50.*t87.*zeta_dot)./1.0e+3-(t51.*t87.*zeta_dot)./2.5e+2-(t52.*t87.*zeta_dot)./1.0e+3-(t53.*t87.*zeta_dot)./1.0e+3-(t54.*t87.*zeta_dot)./2.5e+2-(t55.*t87.*zeta_dot)./1.0e+3-(t56.*t87.*zeta_dot)./1.0e+3-(t57.*t87.*zeta_dot)./2.5e+2-(t58.*t87.*zeta_dot)./1.0e+3-(t59.*t87.*zeta_dot)./1.0e+3+psi_dot.*t3.*t4.*t87.*1.05e-2-psi_dot.*t3.*t5.*t87.*5.25e-3-psi_dot.*t3.*t6.*t87.*5.25e-3-psi_dot.*t3.*t7.*t87.*1.05e-2;
et68 = psi_dot.*t3.*t8.*t87.*5.25e-3+psi_dot.*t3.*t9.*t87.*5.25e-3-psi_dot.*t3.*t10.*t87.*1.05e-2+psi_dot.*t3.*t11.*t87.*5.25e-3+psi_dot.*t3.*t12.*t87.*5.25e-3+psi_dot.*t3.*t13.*t87.*1.05e-2-psi_dot.*t3.*t14.*t87.*5.25e-3-psi_dot.*t3.*t15.*t87.*5.25e-3+psi_dot.*t4.*t18.*t87.*(3.0./1.0e+3)-psi_dot.*t5.*t18.*t87.*1.5e-3-psi_dot.*t6.*t18.*t87.*1.5e-3+psi_dot.*t7.*t18.*t87.*(3.0./1.0e+3)-psi_dot.*t8.*t18.*t87.*1.5e-3-psi_dot.*t9.*t18.*t87.*1.5e-3+psi_dot.*t10.*t18.*t87.*(3.0./1.0e+3)-psi_dot.*t11.*t18.*t87.*1.5e-3;
et69 = psi_dot.*t12.*t18.*t87.*(-1.5e-3)+psi_dot.*t13.*t18.*t87.*(3.0./1.0e+3)-psi_dot.*t14.*t18.*t87.*1.5e-3-psi_dot.*t15.*t18.*t87.*1.5e-3+psi_dot.*t18.*t19.*t87.*(3.0./2.0e+2)+psi_dot.*t18.*t20.*t87.*8.25e-3+psi_dot.*t18.*t21.*t87.*8.25e-3+psi_dot.*t18.*t22.*t87.*(3.0./2.0e+2)+psi_dot.*t18.*t23.*t87.*8.25e-3+psi_dot.*t18.*t24.*t87.*8.25e-3-psi_dot.*t18.*t25.*t87.*(3.0./5.0e+2)-psi_dot.*t18.*t26.*t87.*1.275e-2-psi_dot.*t18.*t27.*t87.*1.275e-2-psi_dot.*t18.*t28.*t87.*(3.0./5.0e+2)-psi_dot.*t18.*t29.*t87.*1.275e-2-psi_dot.*t18.*t30.*t87.*1.275e-2;
et70 = psi_dot.*t19.*t46.*t72.*1.05e-2+psi_dot.*t20.*t46.*t72.*1.05e-2+psi_dot.*t21.*t46.*t72.*1.05e-2-psi_dot.*t22.*t46.*t72.*1.05e-2-psi_dot.*t23.*t46.*t72.*1.05e-2-psi_dot.*t24.*t46.*t72.*1.05e-2+psi_dot.*t5.*t46.*t92.*1.5e-3-psi_dot.*t25.*t46.*t72.*1.05e-2-psi_dot.*t6.*t46.*t92.*1.5e-3-psi_dot.*t26.*t46.*t72.*1.05e-2-psi_dot.*t27.*t46.*t72.*1.05e-2+psi_dot.*t8.*t46.*t92.*1.5e-3+psi_dot.*t28.*t46.*t72.*1.05e-2-psi_dot.*t9.*t46.*t92.*1.5e-3+psi_dot.*t29.*t46.*t72.*1.05e-2+psi_dot.*t30.*t46.*t72.*1.05e-2;
et71 = psi_dot.*t11.*t46.*t92.*1.5e-3-psi_dot.*t12.*t46.*t92.*1.5e-3-psi_dot.*t5.*t72.*t74.*3.375e-3-psi_dot.*t6.*t72.*t74.*3.375e-3+psi_dot.*t14.*t46.*t92.*1.5e-3-psi_dot.*t15.*t46.*t92.*1.5e-3-psi_dot.*t8.*t72.*t74.*3.375e-3-psi_dot.*t9.*t72.*t74.*3.375e-3-psi_dot.*t11.*t72.*t74.*3.375e-3-psi_dot.*t12.*t72.*t74.*3.375e-3+psi_dot.*t20.*t46.*t92.*2.25e-3-psi_dot.*t21.*t46.*t92.*2.25e-3-psi_dot.*t14.*t72.*t74.*3.375e-3-psi_dot.*t15.*t72.*t74.*3.375e-3+psi_dot.*t23.*t46.*t92.*2.25e-3-psi_dot.*t24.*t46.*t92.*2.25e-3;
et72 = psi_dot.*t26.*t46.*t92.*2.25e-3+psi_dot.*t19.*t72.*t74.*(3.0./1.0e+3)-psi_dot.*t27.*t46.*t92.*2.25e-3+psi_dot.*t20.*t72.*t74.*(3.0./1.0e+3)+psi_dot.*t21.*t72.*t74.*(3.0./1.0e+3)+psi_dot.*t29.*t46.*t92.*2.25e-3+psi_dot.*t22.*t72.*t74.*(3.0./1.0e+3)-psi_dot.*t30.*t46.*t92.*2.25e-3+psi_dot.*t23.*t72.*t74.*(3.0./1.0e+3)+psi_dot.*t24.*t72.*t74.*(3.0./1.0e+3)-psi_dot.*t5.*t74.*t92.*5.25e-3+psi_dot.*t25.*t72.*t74.*(3.0./1.0e+3)+psi_dot.*t6.*t74.*t92.*5.25e-3+psi_dot.*t26.*t72.*t74.*(3.0./1.0e+3)+psi_dot.*t27.*t72.*t74.*(3.0./1.0e+3)+psi_dot.*t8.*t74.*t92.*5.25e-3+psi_dot.*t28.*t72.*t74.*(3.0./1.0e+3);
et73 = psi_dot.*t9.*t74.*t92.*(-5.25e-3)+psi_dot.*t29.*t72.*t74.*(3.0./1.0e+3)+psi_dot.*t30.*t72.*t74.*(3.0./1.0e+3)+psi_dot.*t11.*t74.*t92.*5.25e-3-psi_dot.*t12.*t74.*t92.*5.25e-3-psi_dot.*t14.*t74.*t92.*5.25e-3+(psi_dot.*t18.*t75.*t87)./3.75e+2+psi_dot.*t15.*t74.*t92.*5.25e-3-(psi_dot.*t18.*t76.*t87)./7.5e+2-(psi_dot.*t18.*t77.*t87)./7.5e+2+(psi_dot.*t18.*t78.*t87)./3.75e+2-(psi_dot.*t18.*t79.*t87)./7.5e+2-(psi_dot.*t18.*t80.*t87)./7.5e+2+(psi_dot.*t18.*t81.*t87)./3.75e+2-(psi_dot.*t18.*t82.*t87)./7.5e+2-(psi_dot.*t18.*t83.*t87)./7.5e+2+(psi_dot.*t18.*t84.*t87)./3.75e+2;
et74 = psi_dot.*t18.*t85.*t87.*(-1.0./7.5e+2)-(psi_dot.*t18.*t86.*t87)./7.5e+2-(psi_dot.*t48.*t72.*t74)./7.5e+2-psi_dot.*t49.*t72.*t74.*2.333333333333333e-3-psi_dot.*t50.*t72.*t74.*2.333333333333333e-3-(psi_dot.*t51.*t72.*t74)./7.5e+2-psi_dot.*t52.*t72.*t74.*2.333333333333333e-3-psi_dot.*t53.*t72.*t74.*2.333333333333333e-3-(psi_dot.*t54.*t72.*t74)./7.5e+2-psi_dot.*t55.*t72.*t74.*2.333333333333333e-3-psi_dot.*t56.*t72.*t74.*2.333333333333333e-3-(psi_dot.*t57.*t72.*t74)./7.5e+2-psi_dot.*t58.*t72.*t74.*2.333333333333333e-3-psi_dot.*t59.*t72.*t74.*2.333333333333333e-3-(psi_dot.*t46.*t77.*t92)./7.5e+2-(psi_dot.*t46.*t80.*t92)./7.5e+2;
et75 = psi_dot.*t46.*t83.*t92.*(-1.0./7.5e+2)-(psi_dot.*t46.*t86.*t92)./7.5e+2+t46.*t72.*t92.*t294+t46.*t72.*t92.*t296+t46.*t72.*t92.*t298+t46.*t72.*t92.*t300-t3.*t4.*t87.*th11_dot.*(3.0./2.0e+2)-t3.*t5.*t87.*th12_dot.*8.25e-3-t3.*t6.*t87.*th13_dot.*8.25e-3-t3.*t7.*t87.*th21_dot.*(3.0./2.0e+2)-t3.*t8.*t87.*th22_dot.*8.25e-3+t3.*t19.*t87.*th11_dot.*(3.0./1.0e+3)-t3.*t9.*t87.*th23_dot.*8.25e-3-t3.*t20.*t87.*th12_dot.*1.5e-3-t3.*t21.*t87.*th13_dot.*1.5e-3+t3.*t10.*t87.*th31_dot.*(3.0./5.0e+2)+t3.*t11.*t87.*th32_dot.*1.275e-2+t3.*t22.*t87.*th21_dot.*(3.0./1.0e+3)-t4.*t46.*t72.*th11_dot.*1.5e-3;
et76 = t3.*t12.*t87.*th33_dot.*1.275e-2-t3.*t23.*t87.*th22_dot.*1.5e-3-t5.*t46.*t72.*th12_dot.*1.5e-3-t18.*t19.*t87.*th11_dot.*1.05e-2-t3.*t24.*t87.*th23_dot.*1.5e-3-t6.*t46.*t72.*th13_dot.*1.5e-3+t18.*t20.*t87.*th12_dot.*5.25e-3+t18.*t21.*t87.*th13_dot.*5.25e-3+t3.*t13.*t87.*th41_dot.*(3.0./5.0e+2)+t3.*t14.*t87.*th42_dot.*1.275e-2+t3.*t25.*t87.*th31_dot.*(3.0./1.0e+3)-t7.*t46.*t72.*th21_dot.*1.5e-3+t3.*t15.*t87.*th43_dot.*1.275e-2-t3.*t26.*t87.*th32_dot.*1.5e-3-t8.*t46.*t72.*th22_dot.*1.5e-3+t18.*t22.*t87.*th21_dot.*1.05e-2;
et77 = t3.*t48.*t87.*th11_dot.*(-2.0./3.75e+2)-t3.*t27.*t87.*th33_dot.*1.5e-3-t9.*t46.*t72.*th23_dot.*1.5e-3-t18.*t23.*t87.*th22_dot.*5.25e-3-t20.*t46.*t72.*th12_dot.*1.6875e-3+(t3.*t49.*t87.*th12_dot)./3.75e+2-t18.*t24.*t87.*th23_dot.*5.25e-3-t21.*t46.*t72.*th13_dot.*1.6875e-3+(t3.*t50.*t87.*th13_dot)./3.75e+2+t3.*t28.*t87.*th41_dot.*(3.0./1.0e+3)-t10.*t46.*t72.*th31_dot.*1.5e-3-t3.*t29.*t87.*th42_dot.*1.5e-3+t4.*t72.*t74.*th11_dot.*5.25e-3-t11.*t46.*t72.*th32_dot.*1.5e-3+t18.*t25.*t87.*th31_dot.*1.05e-2-t3.*t51.*t87.*th21_dot.*(2.0./3.75e+2);
et78 = t3.*t30.*t87.*th43_dot.*(-1.5e-3)+t5.*t72.*t74.*th12_dot.*5.25e-3-t12.*t46.*t72.*th33_dot.*1.5e-3-t18.*t26.*t87.*th32_dot.*5.25e-3-t23.*t46.*t72.*th22_dot.*1.6875e-3+(t3.*t52.*t87.*th22_dot)./3.75e+2+t6.*t72.*t74.*th13_dot.*5.25e-3-t18.*t27.*t87.*th33_dot.*5.25e-3-t24.*t46.*t72.*th23_dot.*1.6875e-3+(t3.*t53.*t87.*th23_dot)./3.75e+2-t20.*t46.*t92.*th12_dot.*2.625e-3-t13.*t46.*t72.*th41_dot.*1.5e-3+t21.*t46.*t92.*th13_dot.*2.625e-3-t7.*t72.*t74.*th21_dot.*5.25e-3-t14.*t46.*t72.*th42_dot.*1.5e-3-t18.*t28.*t87.*th41_dot.*1.05e-2;
et79 = t3.*t54.*t87.*th31_dot.*(-2.0./3.75e+2)-t8.*t72.*t74.*th22_dot.*5.25e-3-t15.*t46.*t72.*th43_dot.*1.5e-3+t18.*t29.*t87.*th42_dot.*5.25e-3-t26.*t46.*t72.*th32_dot.*1.6875e-3+(t3.*t55.*t87.*th32_dot)./3.75e+2-t9.*t72.*t74.*th23_dot.*5.25e-3+t18.*t30.*t87.*th43_dot.*5.25e-3-t27.*t46.*t72.*th33_dot.*1.6875e-3+(t3.*t56.*t87.*th33_dot)./3.75e+2+t5.*t74.*t92.*th12_dot.*1.125e-3+t23.*t46.*t92.*th22_dot.*2.625e-3-t6.*t74.*t92.*th13_dot.*1.125e-3-t24.*t46.*t92.*th23_dot.*2.625e-3-t10.*t72.*t74.*th31_dot.*5.25e-3-t3.*t57.*t87.*th41_dot.*(2.0./3.75e+2);
et80 = t11.*t72.*t74.*th32_dot.*(-5.25e-3)-t29.*t46.*t72.*th42_dot.*1.6875e-3+(t3.*t58.*t87.*th42_dot)./3.75e+2-t12.*t72.*t74.*th33_dot.*5.25e-3-t30.*t46.*t72.*th43_dot.*1.6875e-3+(t3.*t59.*t87.*th43_dot)./3.75e+2+t8.*t74.*t92.*th22_dot.*1.125e-3+t20.*t72.*t92.*th12_dot.*2.625e-3+t26.*t46.*t92.*th32_dot.*2.625e-3-t9.*t74.*t92.*th23_dot.*1.125e-3-t20.*t74.*t92.*th12_dot.*7.5e-4-t21.*t72.*t92.*th13_dot.*2.625e-3-t27.*t46.*t92.*th33_dot.*2.625e-3+t13.*t72.*t74.*th41_dot.*5.25e-3+t21.*t74.*t92.*th13_dot.*7.5e-4+t14.*t72.*t74.*th42_dot.*5.25e-3;
et81 = t15.*t72.*t74.*th43_dot.*5.25e-3-(t46.*t72.*t75.*th11_dot)./7.5e+2-t46.*t72.*t76.*th12_dot.*2.333333333333333e-3-t46.*t72.*t77.*th13_dot.*2.333333333333333e-3+t11.*t74.*t92.*th32_dot.*1.125e-3-t23.*t72.*t92.*th22_dot.*2.625e-3-t29.*t46.*t92.*th42_dot.*2.625e-3-t12.*t74.*t92.*th33_dot.*1.125e-3-t23.*t74.*t92.*th22_dot.*7.5e-4+t24.*t72.*t92.*th23_dot.*2.625e-3+t30.*t46.*t92.*th43_dot.*2.625e-3+t24.*t74.*t92.*th23_dot.*7.5e-4-(t46.*t72.*t78.*th21_dot)./7.5e+2-t46.*t72.*t79.*th22_dot.*2.333333333333333e-3-t46.*t72.*t80.*th23_dot.*2.333333333333333e-3+t14.*t74.*t92.*th42_dot.*1.125e-3;
et82 = t26.*t72.*t92.*th32_dot.*(-2.625e-3)-t15.*t74.*t92.*th43_dot.*1.125e-3-t26.*t74.*t92.*th32_dot.*7.5e-4+t27.*t72.*t92.*th33_dot.*2.625e-3+t27.*t74.*t92.*th33_dot.*7.5e-4+(t49.*t74.*t92.*th12_dot)./7.5e+2-(t50.*t74.*t92.*th13_dot)./7.5e+2-(t46.*t72.*t81.*th31_dot)./7.5e+2-t46.*t72.*t82.*th32_dot.*2.333333333333333e-3-t46.*t72.*t83.*th33_dot.*2.333333333333333e-3+t29.*t72.*t92.*th42_dot.*2.625e-3-t29.*t74.*t92.*th42_dot.*7.5e-4-t30.*t72.*t92.*th43_dot.*2.625e-3+t30.*t74.*t92.*th43_dot.*7.5e-4+(t52.*t74.*t92.*th22_dot)./7.5e+2-(t53.*t74.*t92.*th23_dot)./7.5e+2;
et83 = t46.*t72.*t84.*th41_dot.*(-1.0./7.5e+2)-t46.*t72.*t85.*th42_dot.*2.333333333333333e-3-t46.*t72.*t86.*th43_dot.*2.333333333333333e-3+(t55.*t74.*t92.*th32_dot)./7.5e+2-(t56.*t74.*t92.*th33_dot)./7.5e+2+(t58.*t74.*t92.*th42_dot)./7.5e+2-(t59.*t74.*t92.*th43_dot)./7.5e+2-t3.*t4.*t72.*zeta_dot.*(3.0./5.0e+2)+t3.*t5.*t72.*zeta_dot.*(3.0./1.0e+3)+t3.*t6.*t72.*zeta_dot.*(3.0./1.0e+3)-t3.*t7.*t72.*zeta_dot.*(3.0./5.0e+2)+t3.*t8.*t72.*zeta_dot.*(3.0./1.0e+3)+t3.*t9.*t72.*zeta_dot.*(3.0./1.0e+3)-t3.*t10.*t72.*zeta_dot.*(3.0./5.0e+2)+t3.*t11.*t72.*zeta_dot.*(3.0./1.0e+3)+t3.*t12.*t72.*zeta_dot.*(3.0./1.0e+3)-t3.*t13.*t72.*zeta_dot.*(3.0./5.0e+2);
et84 = t3.*t14.*t72.*zeta_dot.*(3.0./1.0e+3)+t3.*t15.*t72.*zeta_dot.*(3.0./1.0e+3)-t3.*t19.*t72.*zeta_dot.*(3.0./1.0e+2)+t4.*t18.*t72.*zeta_dot.*(2.1e+1./1.0e+3)-t3.*t20.*t72.*zeta_dot.*1.65e-2-t5.*t18.*t72.*zeta_dot.*1.05e-2-t3.*t21.*t72.*zeta_dot.*1.65e-2-t6.*t18.*t72.*zeta_dot.*1.05e-2-t3.*t22.*t72.*zeta_dot.*(3.0./1.0e+2)-t7.*t18.*t72.*zeta_dot.*(2.1e+1./1.0e+3)-t3.*t23.*t72.*zeta_dot.*1.65e-2+t8.*t18.*t72.*zeta_dot.*1.05e-2-t3.*t24.*t72.*zeta_dot.*1.65e-2+t9.*t18.*t72.*zeta_dot.*1.05e-2-t10.*t18.*t72.*zeta_dot.*(2.1e+1./1.0e+3)+t3.*t26.*t72.*zeta_dot.*2.55e-2;
et85 = t11.*t18.*t72.*zeta_dot.*1.05e-2+t3.*t27.*t72.*zeta_dot.*2.55e-2+t12.*t18.*t72.*zeta_dot.*1.05e-2+t13.*t18.*t72.*zeta_dot.*(2.1e+1./1.0e+3)+t3.*t29.*t72.*zeta_dot.*2.55e-2-t14.*t18.*t72.*zeta_dot.*1.05e-2+t3.*t30.*t72.*zeta_dot.*2.55e-2-t15.*t18.*t72.*zeta_dot.*1.05e-2-t5.*t46.*t87.*zeta_dot.*3.375e-3-t6.*t46.*t87.*zeta_dot.*3.375e-3-t8.*t46.*t87.*zeta_dot.*3.375e-3-t9.*t46.*t87.*zeta_dot.*3.375e-3-t11.*t46.*t87.*zeta_dot.*3.375e-3-t12.*t46.*t87.*zeta_dot.*3.375e-3-t14.*t46.*t87.*zeta_dot.*3.375e-3;
et86 = t15.*t46.*t87.*zeta_dot.*(-3.375e-3)-t3.*t72.*t75.*zeta_dot.*(2.0./3.75e+2)+(t3.*t72.*t76.*zeta_dot)./3.75e+2+(t3.*t72.*t77.*zeta_dot)./3.75e+2+t19.*t46.*t87.*zeta_dot.*(3.0./1.0e+3)-t3.*t72.*t78.*zeta_dot.*(2.0./3.75e+2)+t20.*t46.*t87.*zeta_dot.*(3.0./1.0e+3)+(t3.*t72.*t79.*zeta_dot)./3.75e+2+t21.*t46.*t87.*zeta_dot.*(3.0./1.0e+3)+(t3.*t72.*t80.*zeta_dot)./3.75e+2+t22.*t46.*t87.*zeta_dot.*(3.0./1.0e+3)-t3.*t72.*t81.*zeta_dot.*(2.0./3.75e+2)+t23.*t46.*t87.*zeta_dot.*(3.0./1.0e+3)+(t3.*t72.*t82.*zeta_dot)./3.75e+2+t24.*t46.*t87.*zeta_dot.*(3.0./1.0e+3)+(t3.*t72.*t83.*zeta_dot)./3.75e+2+t25.*t46.*t87.*zeta_dot.*(3.0./1.0e+3)-t3.*t72.*t84.*zeta_dot.*(2.0./3.75e+2);
et87 = t26.*t46.*t87.*zeta_dot.*(3.0./1.0e+3)+(t3.*t72.*t85.*zeta_dot)./3.75e+2+t27.*t46.*t87.*zeta_dot.*(3.0./1.0e+3)+(t3.*t72.*t86.*zeta_dot)./3.75e+2+t28.*t46.*t87.*zeta_dot.*(3.0./1.0e+3)+t29.*t46.*t87.*zeta_dot.*(3.0./1.0e+3)+t30.*t46.*t87.*zeta_dot.*(3.0./1.0e+3)-t19.*t74.*t87.*zeta_dot.*1.05e-2-t20.*t74.*t87.*zeta_dot.*1.05e-2-(t46.*t48.*t87.*zeta_dot)./7.5e+2-t21.*t74.*t87.*zeta_dot.*1.05e-2-t46.*t49.*t87.*zeta_dot.*2.333333333333333e-3+t22.*t74.*t87.*zeta_dot.*1.05e-2-t46.*t50.*t87.*zeta_dot.*2.333333333333333e-3+t5.*t87.*t92.*zeta_dot.*5.25e-3+t23.*t74.*t87.*zeta_dot.*1.05e-2-(t46.*t51.*t87.*zeta_dot)./7.5e+2;
et88 = t6.*t87.*t92.*zeta_dot.*(-5.25e-3)+t24.*t74.*t87.*zeta_dot.*1.05e-2-t46.*t52.*t87.*zeta_dot.*2.333333333333333e-3+t25.*t74.*t87.*zeta_dot.*1.05e-2-t46.*t53.*t87.*zeta_dot.*2.333333333333333e-3-t8.*t87.*t92.*zeta_dot.*5.25e-3+t26.*t74.*t87.*zeta_dot.*1.05e-2-(t46.*t54.*t87.*zeta_dot)./7.5e+2+t9.*t87.*t92.*zeta_dot.*5.25e-3+t27.*t74.*t87.*zeta_dot.*1.05e-2-t46.*t55.*t87.*zeta_dot.*2.333333333333333e-3-t28.*t74.*t87.*zeta_dot.*1.05e-2-t46.*t56.*t87.*zeta_dot.*2.333333333333333e-3-t11.*t87.*t92.*zeta_dot.*5.25e-3-t29.*t74.*t87.*zeta_dot.*1.05e-2-(t46.*t57.*t87.*zeta_dot)./7.5e+2;
et89 = t12.*t87.*t92.*zeta_dot.*5.25e-3-t30.*t74.*t87.*zeta_dot.*1.05e-2-t46.*t58.*t87.*zeta_dot.*2.333333333333333e-3-t46.*t59.*t87.*zeta_dot.*2.333333333333333e-3+t14.*t87.*t92.*zeta_dot.*5.25e-3-t15.*t87.*t92.*zeta_dot.*5.25e-3+psi_dot.*t3.*t5.*t87.*t92.*(3.0./1.0e+3)-psi_dot.*t3.*t6.*t87.*t92.*(3.0./1.0e+3)+psi_dot.*t3.*t8.*t87.*t92.*(3.0./1.0e+3)-psi_dot.*t3.*t9.*t87.*t92.*(3.0./1.0e+3)-psi_dot.*t3.*t11.*t87.*t92.*(3.0./4.0e+2)+psi_dot.*t3.*t12.*t87.*t92.*(3.0./4.0e+2)-psi_dot.*t3.*t14.*t87.*t92.*(3.0./4.0e+2)+psi_dot.*t3.*t15.*t87.*t92.*(3.0./4.0e+2)+psi_dot.*t5.*t46.*t72.*t92.*1.5e-3-psi_dot.*t6.*t46.*t72.*t92.*1.5e-3;
et90 = psi_dot.*t8.*t46.*t72.*t92.*1.5e-3-psi_dot.*t9.*t46.*t72.*t92.*1.5e-3+psi_dot.*t11.*t46.*t72.*t92.*1.5e-3-psi_dot.*t12.*t46.*t72.*t92.*1.5e-3+psi_dot.*t14.*t46.*t72.*t92.*1.5e-3-psi_dot.*t15.*t46.*t72.*t92.*1.5e-3+psi_dot.*t20.*t46.*t72.*t92.*2.25e-3-(psi_dot.*t3.*t49.*t87.*t92)./1.5e+3-psi_dot.*t21.*t46.*t72.*t92.*2.25e-3+(psi_dot.*t3.*t50.*t87.*t92)./1.5e+3+psi_dot.*t23.*t46.*t72.*t92.*2.25e-3-(psi_dot.*t3.*t52.*t87.*t92)./1.5e+3-psi_dot.*t24.*t46.*t72.*t92.*2.25e-3+(psi_dot.*t3.*t53.*t87.*t92)./1.5e+3+psi_dot.*t26.*t46.*t72.*t92.*2.25e-3;
et91 = psi_dot.*t3.*t55.*t87.*t92.*(-6.666666666666667e-4)-psi_dot.*t27.*t46.*t72.*t92.*2.25e-3+(psi_dot.*t3.*t56.*t87.*t92)./1.5e+3+psi_dot.*t29.*t46.*t72.*t92.*2.25e-3-(psi_dot.*t3.*t58.*t87.*t92)./1.5e+3-psi_dot.*t30.*t46.*t72.*t92.*2.25e-3+(psi_dot.*t3.*t59.*t87.*t92)./1.5e+3-psi_dot.*t5.*t72.*t74.*t92.*5.25e-3+psi_dot.*t6.*t72.*t74.*t92.*5.25e-3+psi_dot.*t8.*t72.*t74.*t92.*5.25e-3-psi_dot.*t9.*t72.*t74.*t92.*5.25e-3+psi_dot.*t11.*t72.*t74.*t92.*5.25e-3-psi_dot.*t12.*t72.*t74.*t92.*5.25e-3-psi_dot.*t14.*t72.*t74.*t92.*5.25e-3+psi_dot.*t15.*t72.*t74.*t92.*5.25e-3;
et92 = psi_dot.*t46.*t72.*t77.*t92.*(-1.0./7.5e+2)-(psi_dot.*t46.*t72.*t80.*t92)./7.5e+2-(psi_dot.*t46.*t72.*t83.*t92)./7.5e+2-(psi_dot.*t46.*t72.*t86.*t92)./7.5e+2-t18.*t20.*t87.*t92.*th12_dot.*(3.0./1.0e+3)+t18.*t21.*t87.*t92.*th13_dot.*(3.0./1.0e+3)-t18.*t23.*t87.*t92.*th22_dot.*(3.0./1.0e+3)-t20.*t46.*t72.*t92.*th12_dot.*2.625e-3+t18.*t24.*t87.*t92.*th23_dot.*(3.0./1.0e+3)+t21.*t46.*t72.*t92.*th13_dot.*2.625e-3+t5.*t72.*t74.*t92.*th12_dot.*1.125e-3+t18.*t26.*t87.*t92.*th32_dot.*(3.0./4.0e+2)+t23.*t46.*t72.*t92.*th22_dot.*2.625e-3-t6.*t72.*t74.*t92.*th13_dot.*1.125e-3-t18.*t27.*t87.*t92.*th33_dot.*(3.0./4.0e+2);
et93 = t24.*t46.*t72.*t92.*th23_dot.*(-2.625e-3)+t8.*t72.*t74.*t92.*th22_dot.*1.125e-3+t18.*t29.*t87.*t92.*th42_dot.*(3.0./4.0e+2)+t26.*t46.*t72.*t92.*th32_dot.*2.625e-3-t9.*t72.*t74.*t92.*th23_dot.*1.125e-3-t18.*t30.*t87.*t92.*th43_dot.*(3.0./4.0e+2)-t20.*t72.*t74.*t92.*th12_dot.*7.5e-4-t27.*t46.*t72.*t92.*th33_dot.*2.625e-3+t21.*t72.*t74.*t92.*th13_dot.*7.5e-4+t11.*t72.*t74.*t92.*th32_dot.*1.125e-3-t29.*t46.*t72.*t92.*th42_dot.*2.625e-3-t12.*t72.*t74.*t92.*th33_dot.*1.125e-3-t23.*t72.*t74.*t92.*th22_dot.*7.5e-4+t30.*t46.*t72.*t92.*th43_dot.*2.625e-3+(t18.*t76.*t87.*t92.*th12_dot)./7.5e+2;
et94 = t24.*t72.*t74.*t92.*th23_dot.*7.5e-4-(t18.*t77.*t87.*t92.*th13_dot)./7.5e+2+t14.*t72.*t74.*t92.*th42_dot.*1.125e-3-t15.*t72.*t74.*t92.*th43_dot.*1.125e-3-t26.*t72.*t74.*t92.*th32_dot.*7.5e-4+(t18.*t79.*t87.*t92.*th22_dot)./7.5e+2+t27.*t72.*t74.*t92.*th33_dot.*7.5e-4+(t49.*t72.*t74.*t92.*th12_dot)./7.5e+2-(t18.*t80.*t87.*t92.*th23_dot)./7.5e+2-(t50.*t72.*t74.*t92.*th13_dot)./7.5e+2-t29.*t72.*t74.*t92.*th42_dot.*7.5e-4+(t18.*t82.*t87.*t92.*th32_dot)./7.5e+2+t30.*t72.*t74.*t92.*th43_dot.*7.5e-4+(t52.*t72.*t74.*t92.*th22_dot)./7.5e+2-(t18.*t83.*t87.*t92.*th33_dot)./7.5e+2;
et95 = t53.*t72.*t74.*t92.*th23_dot.*(-1.0./7.5e+2)+(t18.*t85.*t87.*t92.*th42_dot)./7.5e+2+(t55.*t72.*t74.*t92.*th32_dot)./7.5e+2-(t18.*t86.*t87.*t92.*th43_dot)./7.5e+2-(t56.*t72.*t74.*t92.*th33_dot)./7.5e+2+(t58.*t72.*t74.*t92.*th42_dot)./7.5e+2-(t59.*t72.*t74.*t92.*th43_dot)./7.5e+2+t5.*t18.*t72.*t92.*zeta_dot.*(3.0./5.0e+2)-t6.*t18.*t72.*t92.*zeta_dot.*(3.0./5.0e+2)+t8.*t18.*t72.*t92.*zeta_dot.*(3.0./5.0e+2)-t9.*t18.*t72.*t92.*zeta_dot.*(3.0./5.0e+2)-t11.*t18.*t72.*t92.*zeta_dot.*(3.0./2.0e+2)+t12.*t18.*t72.*t92.*zeta_dot.*(3.0./2.0e+2)-t14.*t18.*t72.*t92.*zeta_dot.*(3.0./2.0e+2)+t15.*t18.*t72.*t92.*zeta_dot.*(3.0./2.0e+2)-t5.*t46.*t87.*t92.*zeta_dot.*5.25e-3;
et96 = t6.*t46.*t87.*t92.*zeta_dot.*5.25e-3-(t18.*t49.*t72.*t92.*zeta_dot)./7.5e+2+(t18.*t50.*t72.*t92.*zeta_dot)./7.5e+2+t8.*t46.*t87.*t92.*zeta_dot.*5.25e-3-t9.*t46.*t87.*t92.*zeta_dot.*5.25e-3-(t18.*t52.*t72.*t92.*zeta_dot)./7.5e+2+(t18.*t53.*t72.*t92.*zeta_dot)./7.5e+2+t11.*t46.*t87.*t92.*zeta_dot.*5.25e-3-t12.*t46.*t87.*t92.*zeta_dot.*5.25e-3-(t18.*t55.*t72.*t92.*zeta_dot)./7.5e+2+(t18.*t56.*t72.*t92.*zeta_dot)./7.5e+2-t14.*t46.*t87.*t92.*zeta_dot.*5.25e-3+t15.*t46.*t87.*t92.*zeta_dot.*5.25e-3-(t18.*t58.*t72.*t92.*zeta_dot)./7.5e+2+(t18.*t59.*t72.*t92.*zeta_dot)./7.5e+2;
et97 = t5.*t74.*t87.*t92.*zeta_dot.*(-1.5e-3)+t6.*t74.*t87.*t92.*zeta_dot.*1.5e-3-t8.*t74.*t87.*t92.*zeta_dot.*1.5e-3+t9.*t74.*t87.*t92.*zeta_dot.*1.5e-3-t11.*t74.*t87.*t92.*zeta_dot.*1.5e-3+t12.*t74.*t87.*t92.*zeta_dot.*1.5e-3-t14.*t74.*t87.*t92.*zeta_dot.*1.5e-3+t15.*t74.*t87.*t92.*zeta_dot.*1.5e-3-t20.*t74.*t87.*t92.*zeta_dot.*2.25e-3+t21.*t74.*t87.*t92.*zeta_dot.*2.25e-3-t23.*t74.*t87.*t92.*zeta_dot.*2.25e-3+t24.*t74.*t87.*t92.*zeta_dot.*2.25e-3-t26.*t74.*t87.*t92.*zeta_dot.*2.25e-3+t27.*t74.*t87.*t92.*zeta_dot.*2.25e-3-t29.*t74.*t87.*t92.*zeta_dot.*2.25e-3;
et98 = t30.*t74.*t87.*t92.*zeta_dot.*2.25e-3-(t74.*t76.*t87.*t92.*zeta_dot)./7.5e+2+(t74.*t77.*t87.*t92.*zeta_dot)./7.5e+2-(t74.*t79.*t87.*t92.*zeta_dot)./7.5e+2+(t74.*t80.*t87.*t92.*zeta_dot)./7.5e+2-(t74.*t82.*t87.*t92.*zeta_dot)./7.5e+2+(t74.*t83.*t87.*t92.*zeta_dot)./7.5e+2-(t74.*t85.*t87.*t92.*zeta_dot)./7.5e+2+(t74.*t86.*t87.*t92.*zeta_dot)./7.5e+2;
et99 = -t213-t215-t217-t219-t221-t223-t225-t227-t229-t231-t233-t235+t253+t254+t256+t257+t259+t260+t262+t263-t414-t415-t416-t417-t418-t419-t420-t421+t422+t423+t424-t425-t426-t427-t428-t429-t430+t431+t432+t433+t474+t475+t476+t477-t514-t515+t516+t517-t518-t519-t520-t521+t546+t547+t548+t549+t550+t551+t552+t553+t554+t555+t556+t557+t558-t559+t560-t561+t562-t563+t564-t565-t599+t608+t609+t610+t611+t612+t613+t614+t615-t649-t650;
et100 = -t651-t652-t765-t766+t767+t768+t781+t782+t783+t784+t785+t786+t787+t788+t789+t790+t791+t792+t853+t856+t859+t862-t933-t943-t944-t945-t946-t947-t948-t949-t950+t994+t995+t996+t997+t998+t999+t1000+t1001+t1010+t1011+t1012+t1013+t1014+t1015+t1016+t1017+t1018+t1019+t1020+t1021+t1022+t1023+t1024+t1025+t1026+t1027+t1028+t1029+t1030+t1031+t1032+t1033+t1079+t1080+t1082+t1083+t1085+t1086+t1088+t1089+t1102+t1103+t1104+t1105+t1223+t1224+t1225+t1232+t1233+t1234+t1255-t1256-t1257+t1258-t1259-t1260+t1261+t1262-t1263-t1264+t1265+t1266-t1267-t1268-t1269-t1270+t1271+t1272+t1273+t1274+t1290+t1291+t1292+t1293+t1294+t1295+t1299+t1300+t1301+t1302+t1303+t1304+t1305+t1306+t1308-t1309+t1310-t1311+t1312-t1313+t1314;
et101 = -t1315+t1348+t1349+t1350+t1351+t1372+t1373+t1374+t1375+t1376+t1377+t1378+t1379+t1380+t1381+t1382+t1383+t1384+t1385+t1386+t1387+t1388+t1389+t1390+t1391+t1414+t1415+t1416+t1417+t1418+t1419+t1420+t1421+t1422+t1423+t1424+t1425+t1426+t1427+t1452+t1453+t1454+t1455+t1456+t1457-t1476+t1477+t1478-t1479+t1480-t1481-t1482+t1483+t1484-t1485+t1486-t1487+t1488-t1489+t1490-t1491+t1516+t1517+t1518+t1519+t1520+t1521+t1522+t1523-t1524-t1525-t1526-t1527-t1528-t1529-t1530-t1531-t1557-t1558-t1559+t1560+t1561+t1562+t1563+t1564+t1565-t1566-t1567-t1568+t1607-t1621+t1622-t1623+t1624+t1625+t1627+t1651-t1652-t1653+t1654-t1655+t1656+t1657-t1658-t1699-t1700;
et102 = -t1701-t1702-t1703-t1704-t1705-t1706-t1707-t1708-t1709-t1710+t1825+t1827+t1829+t1831+t1833+t1835+t1837+t1839+t1857+t1859+t1861+t1863+t1894+t1895+t1897+t1900+t1901+t1903+t1905+t1907+t1925+t1926+t1927+t1928+t1929+t1930+t1931+t1932+t1942+t1944+t1946+t1948+t1950+t1951+t1952+t1953+t1954+t1957+t1959+t1960+t1978+t1980+t1982+t1984+t2011+t2013+t2015+t2017+t2058+t2059+t2060+t2061+t2062+t2063+t2064+t2065+t2066+t2067+t2068+t2069+t2071+t2072+t2073+t2074+t2075+t2076+t2077+t2078-t2079+t2080-t2081+t2082-t2083+t2084-t2085+t2086-t2087+t2088-t2089+t2090-t2091+t2092-t2093+t2094+t2095+t2096+t2097+t2098+t2117+t2118+t2120+t2123-t2140+t2141-t2142+t2143-t2144+t2145-t2146+t2147+t2167+t2169+t2171+t2173+t31.*t653+t31.*t654+t31.*t655+t31.*t656+t31.*t892+t31.*t893;
et103 = t31.*t894+t31.*t895+t31.*t896+t31.*t897+t31.*t901+t31.*t902+t31.*t903+t31.*t904+t31.*t905+t31.*t906+t31.*t907+t31.*t908+t31.*t934+t31.*t951+t31.*t952+t31.*t953+t31.*t954+t31.*t955+t31.*t956+t31.*t957+t31.*t958+t31.*t1550+t31.*t1552+t31.*t1554+t31.*t1556+t31.*t1676+t31.*t1678+t31.*t1679+t31.*t1682+t31.*t1684+t31.*t1686+t31.*t1688+t31.*t1689+t31.*t1752+t31.*t1754+t31.*t1756+t31.*t1758-phi_dot.*t46.*t87.*1.5428125e-1+t16.*t18.*t151+t16.*t18.*t152+t16.*t75.*t150+t16.*t78.*t150+t16.*t81.*t150+t16.*t84.*t150-t18.*t31.*th11_dot.*(2.0./3.75e+2)-t18.*t31.*th21_dot.*(2.0./3.75e+2)-t18.*t31.*th31_dot.*(2.0./3.75e+2)-t18.*t31.*th41_dot.*(2.0./3.75e+2);
et104 = phi_dot.*t3.*t4.*t72.*(-3.0./5.0e+2)-phi_dot.*t3.*t7.*t72.*(3.0./5.0e+2)-phi_dot.*t3.*t10.*t72.*(3.0./5.0e+2)-phi_dot.*t3.*t13.*t72.*(3.0./5.0e+2)-phi_dot.*t3.*t72.*t75.*(2.0./3.75e+2)-phi_dot.*t3.*t72.*t78.*(2.0./3.75e+2)-phi_dot.*t3.*t72.*t81.*(2.0./3.75e+2)-phi_dot.*t3.*t72.*t84.*(2.0./3.75e+2)-t3.*t19.*t31.*th11_dot.*(2.1e+1./1.0e+3)+t3.*t20.*t31.*th12_dot.*1.05e-2+t3.*t21.*t31.*th13_dot.*1.05e-2+t3.*t22.*t31.*th21_dot.*(2.1e+1./1.0e+3)-t3.*t23.*t31.*th22_dot.*1.05e-2-t18.*t19.*t31.*th11_dot.*(3.0./5.0e+2)-t3.*t24.*t31.*th23_dot.*1.05e-2+t18.*t20.*t31.*th12_dot.*(3.0./1.0e+3)+t18.*t21.*t31.*th13_dot.*(3.0./1.0e+3);
et105 = t3.*t25.*t31.*th31_dot.*(2.1e+1./1.0e+3)-t3.*t26.*t31.*th32_dot.*1.05e-2-t18.*t22.*t31.*th21_dot.*(3.0./5.0e+2)-t3.*t27.*t31.*th33_dot.*1.05e-2+t18.*t23.*t31.*th22_dot.*(3.0./1.0e+3)+t18.*t24.*t31.*th23_dot.*(3.0./1.0e+3)-t3.*t28.*t31.*th41_dot.*(2.1e+1./1.0e+3)+t3.*t29.*t31.*th42_dot.*1.05e-2-t18.*t25.*t31.*th31_dot.*(3.0./5.0e+2)+t3.*t30.*t31.*th43_dot.*1.05e-2+t18.*t26.*t31.*th32_dot.*(3.0./1.0e+3)+t18.*t27.*t31.*th33_dot.*(3.0./1.0e+3)-t18.*t28.*t31.*th41_dot.*(3.0./5.0e+2)+t18.*t29.*t31.*th42_dot.*(3.0./1.0e+3)+t18.*t30.*t31.*th43_dot.*(3.0./1.0e+3)+t3.*t4.*t16.*zeta_dot.*(2.1e+1./1.0e+3)-t3.*t5.*t16.*zeta_dot.*1.05e-2;
et106 = t3.*t6.*t16.*zeta_dot.*(-1.05e-2)-t3.*t7.*t16.*zeta_dot.*(2.1e+1./1.0e+3)+t3.*t8.*t16.*zeta_dot.*1.05e-2+t3.*t9.*t16.*zeta_dot.*1.05e-2-t3.*t10.*t16.*zeta_dot.*(2.1e+1./1.0e+3)+t3.*t11.*t16.*zeta_dot.*1.05e-2+t3.*t12.*t16.*zeta_dot.*1.05e-2+t3.*t13.*t16.*zeta_dot.*(2.1e+1./1.0e+3)-t3.*t14.*t16.*zeta_dot.*1.05e-2-t3.*t15.*t16.*zeta_dot.*1.05e-2+t4.*t16.*t18.*zeta_dot.*(3.0./5.0e+2)-t5.*t16.*t18.*zeta_dot.*(3.0./1.0e+3)-t6.*t16.*t18.*zeta_dot.*(3.0./1.0e+3)+t7.*t16.*t18.*zeta_dot.*(3.0./5.0e+2)-t8.*t16.*t18.*zeta_dot.*(3.0./1.0e+3)-t9.*t16.*t18.*zeta_dot.*(3.0./1.0e+3);
et107 = t10.*t16.*t18.*zeta_dot.*(3.0./5.0e+2)-t11.*t16.*t18.*zeta_dot.*(3.0./1.0e+3)-t12.*t16.*t18.*zeta_dot.*(3.0./1.0e+3)+t13.*t16.*t18.*zeta_dot.*(3.0./5.0e+2)-t14.*t16.*t18.*zeta_dot.*(3.0./1.0e+3)-t15.*t16.*t18.*zeta_dot.*(3.0./1.0e+3)+t16.*t18.*t20.*zeta_dot.*1.65e-2+t16.*t18.*t21.*zeta_dot.*1.65e-2+t16.*t18.*t23.*zeta_dot.*1.65e-2+t16.*t18.*t24.*zeta_dot.*1.65e-2-t16.*t18.*t25.*zeta_dot.*(3.0./2.5e+2)-t16.*t18.*t26.*zeta_dot.*2.55e-2-t16.*t18.*t27.*zeta_dot.*2.55e-2-t16.*t18.*t28.*zeta_dot.*(3.0./2.5e+2)-t16.*t18.*t29.*zeta_dot.*2.55e-2-t16.*t18.*t30.*zeta_dot.*2.55e-2;
et108 = t19.*t31.*t46.*zeta_dot.*(-2.1e+1./1.0e+3)-t20.*t31.*t46.*zeta_dot.*(2.1e+1./1.0e+3)-t21.*t31.*t46.*zeta_dot.*(2.1e+1./1.0e+3)-t28.*t31.*t46.*zeta_dot.*(2.1e+1./1.0e+3)-t29.*t31.*t46.*zeta_dot.*(2.1e+1./1.0e+3)-t30.*t31.*t46.*zeta_dot.*(2.1e+1./1.0e+3)-(t16.*t18.*t76.*zeta_dot)./3.75e+2-(t16.*t18.*t77.*zeta_dot)./3.75e+2-(t16.*t18.*t79.*zeta_dot)./3.75e+2-(t16.*t18.*t80.*zeta_dot)./3.75e+2-(t16.*t18.*t82.*zeta_dot)./3.75e+2-(t16.*t18.*t83.*zeta_dot)./3.75e+2-(t16.*t18.*t85.*zeta_dot)./3.75e+2-(t16.*t18.*t86.*zeta_dot)./3.75e+2-t19.*t31.*t74.*zeta_dot.*(3.0./5.0e+2)-t20.*t31.*t74.*zeta_dot.*(3.0./5.0e+2)-t21.*t31.*t74.*zeta_dot.*(3.0./5.0e+2);
et109 = t22.*t31.*t74.*zeta_dot.*(-3.0./5.0e+2)-t23.*t31.*t74.*zeta_dot.*(3.0./5.0e+2)-t24.*t31.*t74.*zeta_dot.*(3.0./5.0e+2)-t25.*t31.*t74.*zeta_dot.*(3.0./5.0e+2)-t26.*t31.*t74.*zeta_dot.*(3.0./5.0e+2)-t27.*t31.*t74.*zeta_dot.*(3.0./5.0e+2)-t28.*t31.*t74.*zeta_dot.*(3.0./5.0e+2)-t29.*t31.*t74.*zeta_dot.*(3.0./5.0e+2)-t30.*t31.*t74.*zeta_dot.*(3.0./5.0e+2)-phi_dot.*t6.*t18.*t72.*t92.*(3.0./5.0e+2)-phi_dot.*t9.*t18.*t72.*t92.*(3.0./5.0e+2)-phi_dot.*t5.*t46.*t87.*t92.*5.25e-3-phi_dot.*t9.*t46.*t87.*t92.*5.25e-3-phi_dot.*t12.*t46.*t87.*t92.*5.25e-3-phi_dot.*t14.*t46.*t87.*t92.*5.25e-3-(phi_dot.*t74.*t76.*t87.*t92)./7.5e+2;
et110 = phi_dot.*t74.*t79.*t87.*t92.*(-1.0./7.5e+2)-(phi_dot.*t74.*t82.*t87.*t92)./7.5e+2-(phi_dot.*t74.*t85.*t87.*t92)./7.5e+2+t3.*t20.*t31.*t92.*th12_dot.*2.25e-3-t3.*t21.*t31.*t92.*th13_dot.*2.25e-3+t3.*t23.*t31.*t92.*th22_dot.*2.25e-3-t3.*t24.*t31.*t92.*th23_dot.*2.25e-3+t3.*t26.*t31.*t92.*th32_dot.*2.25e-3-t3.*t27.*t31.*t92.*th33_dot.*2.25e-3+t3.*t29.*t31.*t92.*th42_dot.*2.25e-3-t3.*t30.*t31.*t92.*th43_dot.*2.25e-3+t3.*t5.*t16.*t92.*zeta_dot.*(3.0./5.0e+2)-t3.*t6.*t16.*t92.*zeta_dot.*(3.0./5.0e+2)+t3.*t8.*t16.*t92.*zeta_dot.*(3.0./5.0e+2)-t3.*t9.*t16.*t92.*zeta_dot.*(3.0./5.0e+2);
et111 = t3.*t11.*t16.*t92.*zeta_dot.*(-3.0./2.0e+2)+t3.*t12.*t16.*t92.*zeta_dot.*(3.0./2.0e+2)-t3.*t14.*t16.*t92.*zeta_dot.*(3.0./2.0e+2)+t3.*t15.*t16.*t92.*zeta_dot.*(3.0./2.0e+2)-(t3.*t16.*t49.*t92.*zeta_dot)./7.5e+2+(t3.*t16.*t50.*t92.*zeta_dot)./7.5e+2-(t3.*t16.*t52.*t92.*zeta_dot)./7.5e+2+(t3.*t16.*t53.*t92.*zeta_dot)./7.5e+2-(t3.*t16.*t55.*t92.*zeta_dot)./7.5e+2+(t3.*t16.*t56.*t92.*zeta_dot)./7.5e+2-(t3.*t16.*t58.*t92.*zeta_dot)./7.5e+2+(t3.*t16.*t59.*t92.*zeta_dot)./7.5e+2-t5.*t31.*t46.*t92.*zeta_dot.*(3.0./1.0e+3)-t8.*t31.*t46.*t92.*zeta_dot.*(3.0./1.0e+3)-t11.*t31.*t46.*t92.*zeta_dot.*(3.0./1.0e+3)-t14.*t31.*t46.*t92.*zeta_dot.*(3.0./1.0e+3);
et112 = t20.*t31.*t46.*t92.*zeta_dot.*(-4.5e-3)-t23.*t31.*t46.*t92.*zeta_dot.*4.5e-3-t26.*t31.*t46.*t92.*zeta_dot.*4.5e-3-t29.*t31.*t46.*t92.*zeta_dot.*4.5e-3-t6.*t31.*t74.*t92.*zeta_dot.*1.05e-2-t8.*t31.*t74.*t92.*zeta_dot.*1.05e-2-t11.*t31.*t74.*t92.*zeta_dot.*1.05e-2-t15.*t31.*t74.*t92.*zeta_dot.*1.05e-2-(t31.*t46.*t76.*t92.*zeta_dot)./3.75e+2-(t31.*t46.*t79.*t92.*zeta_dot)./3.75e+2-(t31.*t46.*t82.*t92.*zeta_dot)./3.75e+2-(t31.*t46.*t85.*t92.*zeta_dot)./3.75e+2;
et113 = t304+t305+t306+t307+t308+t309+t310+t311+t312+t313+t314+t315+t462+t463+t464+t465+t466+t467+t468+t469+t586+t587+t588+t589+t590+t591+t592+t593+t594+t595+t596+t597+t659+t661+t663+t665+t667+t668-t669-t670+t753+t756+t759+t762+t817+t818+t819+t820+t821+t822+t823+t824+t825+t826+t827+t828-t877-t878-t879+t880+t881+t882+t883+t884+t885-t886-t887-t888-t961-t963-t965-t967-t969-t971-t973-t975-t976-t977-t978+t979+t980+t981+t982+t983+t984-t985-t986-t987+t1002+t1003+t1004+t1005+t1006+t1007+t1008+t1009-t1054-t1055-t1056-t1057-t1058-t1059-t1060-t1061-t1062;
et114 = -t1063-t1064-t1065+t1106-t1107-t1108+t1109-t1110-t1111+t1112-t1113-t1114+t1115-t1116-t1117+t1118+t1121-t1122-t1123+t1124+t1125+t1128+t1129-t1132-t1133+t1162+t1163+t1166+t1167-t1170-t1171-t1172-t1173+t1183+t1184+t1185+t1186+t1187+t1188+t1189+t1190+t1191+t1192+t1193+t1194-t1247-t1248-t1249-t1250-t1251-t1252-t1253-t1254-t1307+t1332+t1335+t1337+t1338+t1360+t1361+t1362-t1363-t1364-t1365-t1366-t1367-t1368+t1369+t1370+t1371+t1512+t1513+t1514+t1515-t1541+t1542-t1543+t1544-t1545+t1546-t1547+t1548-t1590;
et115 = -t1591-t1592-t1593-t1594-t1595-t1596-t1597-t1598-t1608-t1609-t1610-t1611-t1612-t1613-t1614-t1615-t1616-t1617-t1618-t1619+t1638+t1640+t1642+t1644-t1659+t1660-t1661+t1662-t1665+t1666-t1669+t1670-t1711+t1712-t1713+t1714+t1715+t1717+t1720+t1722+t1724+t1726+t1760+t1762+t1764+t1766+t1865+t1866+t1867+t1868-t1869+t1870-t1871+t1872-t1873+t1874-t1875+t1876+t1910+t1911+t1913+t1916+t1970+t1972+t1974+t1976-t1994+t1995-t1996+t1997-t1998+t1999-t2000+t2001-t2034+t2035-t2036+t2037-t2038+t2039-t2040+t2041+t2108;
et116 = -t2109+t2110-t2111+t2112-t2113+t2114-t2115+t2124-t2125+t2126-t2127+t2128-t2129+t2130-t2131+t2151+t2152+t2154+t2157-t16.*zeta_dot.*1.508875e-1-t16.*t19.*zeta_dot.*(3.0./2.5e+2)-t16.*t20.*zeta_dot.*(3.0./2.5e+2)-t16.*t21.*zeta_dot.*(3.0./2.5e+2)-t16.*t22.*zeta_dot.*(3.0./2.5e+2)-t16.*t23.*zeta_dot.*(3.0./2.5e+2)-t16.*t24.*zeta_dot.*(3.0./2.5e+2)-t16.*t25.*zeta_dot.*(3.0./2.5e+2)-t16.*t26.*zeta_dot.*(3.0./2.5e+2)-t16.*t27.*zeta_dot.*(3.0./2.5e+2)-t16.*t28.*zeta_dot.*(3.0./2.5e+2)-t16.*t29.*zeta_dot.*(3.0./2.5e+2)-t16.*t30.*zeta_dot.*(3.0./2.5e+2)+t16.*t60.*zeta_dot.*(4.0./3.75e+2)+t16.*t61.*zeta_dot.*(4.0./3.75e+2);
et117 = t16.*t62.*zeta_dot.*(4.0./3.75e+2)+t16.*t63.*zeta_dot.*(4.0./3.75e+2)+t16.*t64.*zeta_dot.*(4.0./3.75e+2)+t16.*t65.*zeta_dot.*(4.0./3.75e+2)+t16.*t66.*zeta_dot.*(4.0./3.75e+2)+t16.*t67.*zeta_dot.*(4.0./3.75e+2)+t16.*t68.*zeta_dot.*(4.0./3.75e+2)+t16.*t69.*zeta_dot.*(4.0./3.75e+2)+t16.*t70.*zeta_dot.*(4.0./3.75e+2)+t16.*t71.*zeta_dot.*(4.0./3.75e+2)-psi_dot.*t3.*t4.*t16.*(2.1e+1./1.0e+3)+psi_dot.*t3.*t5.*t16.*1.05e-2+psi_dot.*t3.*t6.*t16.*1.05e-2+psi_dot.*t3.*t7.*t16.*(2.1e+1./1.0e+3)-psi_dot.*t3.*t8.*t16.*1.05e-2-psi_dot.*t3.*t9.*t16.*1.05e-2+psi_dot.*t3.*t10.*t16.*(2.1e+1./1.0e+3)-psi_dot.*t3.*t11.*t16.*1.05e-2;
et118 = psi_dot.*t3.*t12.*t16.*(-1.05e-2)-psi_dot.*t3.*t13.*t16.*(2.1e+1./1.0e+3)+psi_dot.*t3.*t14.*t16.*1.05e-2+psi_dot.*t3.*t15.*t16.*1.05e-2-psi_dot.*t4.*t16.*t18.*(3.0./5.0e+2)+psi_dot.*t5.*t16.*t18.*(3.0./1.0e+3)+psi_dot.*t6.*t16.*t18.*(3.0./1.0e+3)-psi_dot.*t7.*t16.*t18.*(3.0./5.0e+2)+psi_dot.*t8.*t16.*t18.*(3.0./1.0e+3)+psi_dot.*t9.*t16.*t18.*(3.0./1.0e+3)-psi_dot.*t10.*t16.*t18.*(3.0./5.0e+2)+psi_dot.*t11.*t16.*t18.*(3.0./1.0e+3)+psi_dot.*t12.*t16.*t18.*(3.0./1.0e+3)-psi_dot.*t13.*t16.*t18.*(3.0./5.0e+2)+psi_dot.*t14.*t16.*t18.*(3.0./1.0e+3)+psi_dot.*t15.*t16.*t18.*(3.0./1.0e+3)-psi_dot.*t16.*t18.*t19.*(3.0./1.0e+2);
et119 = psi_dot.*t16.*t18.*t20.*(-1.65e-2)-psi_dot.*t16.*t18.*t21.*1.65e-2-psi_dot.*t16.*t18.*t22.*(3.0./1.0e+2)-psi_dot.*t16.*t18.*t23.*1.65e-2-psi_dot.*t16.*t18.*t24.*1.65e-2+psi_dot.*t16.*t18.*t25.*(3.0./2.5e+2)+psi_dot.*t16.*t18.*t26.*2.55e-2+psi_dot.*t16.*t18.*t27.*2.55e-2+psi_dot.*t16.*t18.*t28.*(3.0./2.5e+2)+psi_dot.*t16.*t18.*t29.*2.55e-2+psi_dot.*t16.*t18.*t30.*2.55e-2+t5.*t16.*t20.*t136+t6.*t16.*t21.*t136+t8.*t16.*t23.*t136+t9.*t16.*t24.*t136+t11.*t16.*t26.*t136+t12.*t16.*t27.*t136+t14.*t16.*t29.*t136+t15.*t16.*t30.*t136+t3.*t16.*t92.*t126+t3.*t16.*t92.*t129+t3.*t4.*t16.*th11_dot.*(3.0./1.0e+2);
et120 = t3.*t5.*t16.*th12_dot.*1.65e-2+t3.*t6.*t16.*th13_dot.*1.65e-2+t3.*t7.*t16.*th21_dot.*(3.0./1.0e+2)+t3.*t8.*t16.*th22_dot.*1.65e-2+t3.*t9.*t16.*th23_dot.*1.65e-2-t3.*t10.*t16.*th31_dot.*(3.0./2.5e+2)-t3.*t11.*t16.*th32_dot.*2.55e-2-t3.*t12.*t16.*th33_dot.*2.55e-2-t3.*t13.*t16.*th41_dot.*(3.0./2.5e+2)-t3.*t14.*t16.*th42_dot.*2.55e-2-t3.*t15.*t16.*th43_dot.*2.55e-2-phi_dot.*t3.*t7.*t16.*t31.*(2.1e+1./1.0e+3)-phi_dot.*t3.*t10.*t16.*t31.*(2.1e+1./1.0e+3)-phi_dot.*t5.*t20.*t73.*t92.*(2.0./3.75e+2)-phi_dot.*t8.*t23.*t73.*t92.*(2.0./3.75e+2)-phi_dot.*t11.*t26.*t73.*t92.*(2.0./3.75e+2);
et121 = phi_dot.*t14.*t29.*t73.*t92.*(-2.0./3.75e+2)-phi_dot.*t6.*t47.*t73.*t92.*(3.0./5.0e+2)-phi_dot.*t9.*t47.*t73.*t92.*(3.0./5.0e+2)-phi_dot.*t12.*t47.*t73.*t92.*(3.0./5.0e+2)-phi_dot.*t15.*t47.*t73.*t92.*(3.0./5.0e+2)-psi_dot.*t4.*t16.*t18.*t19.*(4.0./3.75e+2)-psi_dot.*t7.*t16.*t18.*t22.*(4.0./3.75e+2)-psi_dot.*t10.*t16.*t18.*t25.*(4.0./3.75e+2)-psi_dot.*t13.*t16.*t18.*t28.*(4.0./3.75e+2)-psi_dot.*t3.*t5.*t16.*t92.*(3.0./5.0e+2)-psi_dot.*t3.*t8.*t16.*t92.*(3.0./5.0e+2)+psi_dot.*t3.*t11.*t16.*t92.*(3.0./2.0e+2)-psi_dot.*t3.*t12.*t16.*t92.*(3.0./2.0e+2)+psi_dot.*t3.*t14.*t16.*t92.*(3.0./2.0e+2)-psi_dot.*t3.*t15.*t16.*t92.*(3.0./2.0e+2)+(psi_dot.*t3.*t16.*t61.*t92)./3.75e+2;
et122 = psi_dot.*t3.*t16.*t62.*t92.*(-1.0./3.75e+2)+(psi_dot.*t3.*t16.*t64.*t92)./3.75e+2-(psi_dot.*t3.*t16.*t65.*t92)./3.75e+2+(psi_dot.*t3.*t16.*t67.*t92)./3.75e+2-(psi_dot.*t3.*t16.*t68.*t92)./3.75e+2+(psi_dot.*t3.*t16.*t70.*t92)./3.75e+2-(psi_dot.*t3.*t16.*t71.*t92)./3.75e+2+t16.*t18.*t20.*t92.*th12_dot.*8.25e-3-t16.*t18.*t21.*t92.*th13_dot.*8.25e-3+t16.*t18.*t23.*t92.*th22_dot.*8.25e-3-t16.*t18.*t24.*t92.*th23_dot.*8.25e-3-t16.*t18.*t26.*t92.*th32_dot.*1.275e-2+t16.*t18.*t27.*t92.*th33_dot.*1.275e-2-t16.*t18.*t29.*t92.*th42_dot.*1.275e-2+t16.*t18.*t30.*t92.*th43_dot.*1.275e-2;
et123 = t5.*t16.*t47.*t92.*zeta_dot.*(-2.1e+1./1.0e+3)-t9.*t16.*t47.*t92.*zeta_dot.*(2.1e+1./1.0e+3)-t12.*t16.*t47.*t92.*zeta_dot.*(2.1e+1./1.0e+3)-t14.*t16.*t47.*t92.*zeta_dot.*(2.1e+1./1.0e+3)-phi_dot.*t3.*t6.*t16.*t31.*t92.*(3.0./5.0e+2)-phi_dot.*t3.*t9.*t16.*t31.*t92.*(3.0./5.0e+2)-phi_dot.*t3.*t5.*t18.*t73.*t92.*(2.1e+1./1.0e+3)-phi_dot.*t3.*t9.*t18.*t73.*t92.*(2.1e+1./1.0e+3)-phi_dot.*t3.*t12.*t18.*t73.*t92.*(2.1e+1./1.0e+3)-phi_dot.*t3.*t14.*t18.*t73.*t92.*(2.1e+1./1.0e+3)-t3.*t5.*t16.*t18.*t92.*zeta_dot.*(3.0./5.0e+2)-t3.*t8.*t16.*t18.*t92.*zeta_dot.*(3.0./5.0e+2)-t3.*t11.*t16.*t18.*t92.*zeta_dot.*(3.0./5.0e+2)-t3.*t14.*t16.*t18.*t92.*zeta_dot.*(3.0./5.0e+2);
et124 = t113+t264-t266+t286-t369+t454+t524+t566+t583+t638+t794-t917+t1091-t1126+t1146+t1158+t1175+t1236+t1324-t1501+t1569+t1579+t1663-t1743+t1767+t1807-t1841+t1917+t1986+t2018+t2042-t2050+t2100+t2158+t31.*t316+t31.*t438+t31.*t1492-psi_dot.*t5.*t31.*(3.0./5.0e+2)-t20.*t31.*th12_dot.*(2.1e+1./1.0e+3)-phi_dot.*t5.*t47.*t73.*(3.0./5.0e+2)-phi_dot.*t20.*t47.*t73.*6.75e-3+psi_dot.*t3.*t5.*t16.*1.65e-2-psi_dot.*t3.*t16.*t61.*(2.0./3.75e+2)-t3.*t5.*t16.*th12_dot.*1.05e-2-t5.*t16.*t18.*th12_dot.*(3.0./1.0e+3)-t16.*t18.*t20.*th12_dot.*1.65e-2+t5.*t31.*t92.*th12_dot.*(3.0./1.0e+3)-t20.*t31.*t92.*th12_dot.*4.5e-3;
et125 = t18.*t31.*t61.*zeta_dot.*(-2.0./3.75e+2)+t16.*t20.*t92.*zeta_dot.*(3.0./1.0e+3)-t16.*t61.*t92.*zeta_dot.*(2.0./3.75e+2)-phi_dot.*t3.*t16.*t20.*t31.*(3.0./1.0e+3)-phi_dot.*t20.*t47.*t73.*t92.*1.05e-2+psi_dot.*t16.*t18.*t20.*t92.*8.25e-3-t3.*t5.*t16.*t92.*th12_dot.*1.05e-2-phi_dot.*t16.*t18.*t20.*t31.*t92.*(3.0./5.0e+2);
et126 = t114+t264-t267+t287-t371+t455+t525+t583+t620+t639+t795+t918+t1092-t1127+t1147+t1159+t1176+t1237+t1401+t1403-t1502+t1580+t1620+t1744+t1780+t1842-t1918-t1987+t2051-t2101+t2133-t2159+t31.*t317+t31.*t439-psi_dot.*t6.*t31.*(3.0./5.0e+2)+t3.*t92.*t424-t21.*t31.*th13_dot.*(2.1e+1./1.0e+3)-phi_dot.*t6.*t47.*t73.*(3.0./5.0e+2)-phi_dot.*t21.*t47.*t73.*6.75e-3-phi_dot.*t21.*t73.*t92.*1.05e-2+psi_dot.*t3.*t6.*t16.*1.65e-2-psi_dot.*t3.*t16.*t62.*(2.0./3.75e+2)-psi_dot.*t21.*t31.*t92.*1.05e-2-t3.*t6.*t16.*th13_dot.*1.05e-2-t6.*t16.*t18.*th13_dot.*(3.0./1.0e+3)-t16.*t18.*t21.*th13_dot.*1.65e-2;
et127 = t6.*t31.*t92.*th13_dot.*(-3.0./1.0e+3)+t21.*t31.*t92.*th13_dot.*4.5e-3-t18.*t31.*t62.*zeta_dot.*(2.0./3.75e+2)-t16.*t21.*t92.*zeta_dot.*(3.0./1.0e+3)-phi_dot.*t3.*t16.*t21.*t31.*(3.0./1.0e+3)-psi_dot.*t16.*t18.*t21.*t92.*8.25e-3-t3.*t21.*t31.*t92.*zeta_dot.*2.25e-3-t3.*t16.*t18.*t21.*t92.*zeta_dot.*1.05e-2-(t3.*t6.*t21.*t31.*t92.*zeta_dot)./3.75e+2-phi_dot.*t6.*t16.*t18.*t21.*t31.*t92.*(2.0./3.75e+2);
et128 = t116+t264-t268+t288-t372+t456+t526+t566+t583+t641+t797+t919+t1094-t1130+t1148+t1177-t1239-t1504+t1569-t1582-t1745+t1769+t1807-t1843+t1919+t1988+t2020-t2052+t2102+t2134+t2160+t31.*t318+t3.*t426+t31.*t1494-psi_dot.*t8.*t31.*(3.0./5.0e+2)+t23.*t31.*th22_dot.*(2.1e+1./1.0e+3)-phi_dot.*t8.*t47.*t73.*(3.0./5.0e+2)-phi_dot.*t23.*t47.*t73.*6.75e-3-phi_dot.*t23.*t73.*t92.*1.05e-2+psi_dot.*t3.*t8.*t16.*1.65e-2-psi_dot.*t3.*t16.*t64.*(2.0./3.75e+2)-psi_dot.*t23.*t31.*t92.*1.05e-2-t8.*t16.*t18.*th22_dot.*(3.0./1.0e+3)-t16.*t18.*t23.*th22_dot.*1.65e-2+t8.*t31.*t92.*th22_dot.*(3.0./1.0e+3);
et129 = t23.*t31.*t92.*th22_dot.*(-4.5e-3)-t3.*t23.*t31.*zeta_dot.*1.05e-2-t18.*t31.*t64.*zeta_dot.*(2.0./3.75e+2)+t16.*t23.*t92.*zeta_dot.*(3.0./1.0e+3)-t16.*t64.*t92.*zeta_dot.*(2.0./3.75e+2)-phi_dot.*t3.*t16.*t23.*t31.*(3.0./1.0e+3)-phi_dot.*t16.*t18.*t23.*t31.*1.05e-2+psi_dot.*t16.*t18.*t23.*t92.*8.25e-3-t3.*t8.*t16.*t92.*th22_dot.*1.05e-2-phi_dot.*t16.*t18.*t23.*t31.*t92.*(3.0./5.0e+2)-t3.*t16.*t18.*t23.*t92.*zeta_dot.*1.05e-2;
et130 = t117+t264-t269+t289-t374+t457+t527+t583+t620+t642+t798-t920+t1095-t1131+t1149+t1178-t1240+t1327+t1401+t1405-t1505-t1583+t1620+t1668+t1746+t1782+t1844-t1920-t1989+t2045+t2053-t2103-t2161+t31.*t319+t3.*t427-psi_dot.*t9.*t31.*(3.0./5.0e+2)+t3.*t92.*t427+t24.*t31.*th23_dot.*(2.1e+1./1.0e+3)-phi_dot.*t9.*t47.*t73.*(3.0./5.0e+2)-phi_dot.*t24.*t47.*t73.*6.75e-3+psi_dot.*t3.*t9.*t16.*1.65e-2-psi_dot.*t3.*t16.*t65.*(2.0./3.75e+2)-t9.*t16.*t18.*th23_dot.*(3.0./1.0e+3)-t16.*t18.*t24.*th23_dot.*1.65e-2-t9.*t31.*t92.*th23_dot.*(3.0./1.0e+3)+t24.*t31.*t92.*th23_dot.*4.5e-3;
et131 = t3.*t24.*t31.*zeta_dot.*(-1.05e-2)-t18.*t31.*t65.*zeta_dot.*(2.0./3.75e+2)-t16.*t24.*t92.*zeta_dot.*(3.0./1.0e+3)-phi_dot.*t3.*t16.*t24.*t31.*(3.0./1.0e+3)-phi_dot.*t16.*t18.*t24.*t31.*1.05e-2-phi_dot.*t24.*t47.*t73.*t92.*1.05e-2-psi_dot.*t16.*t18.*t24.*t92.*8.25e-3-t3.*t24.*t31.*t92.*zeta_dot.*2.25e-3-(t3.*t9.*t24.*t31.*t92.*zeta_dot)./3.75e+2-phi_dot.*t9.*t16.*t18.*t24.*t31.*t92.*(2.0./3.75e+2);
et132 = t119+t264-t270+t290-t375+t458-t530+t566+t583+t644+t800+t921+t1097+t1134+t1150+t1179-t1242-t1507+t1569-t1585-t1747+t1771+t1775+t1807-t1845+t1921+t1990+t2022-t2054+t2104+t2136+t2162+t31.*t320+t3.*t429+t31.*t1496-psi_dot.*t11.*t31.*(3.0./5.0e+2)+t3.*t92.*t429+t26.*t31.*th32_dot.*(2.1e+1./1.0e+3)-phi_dot.*t11.*t47.*t73.*(3.0./5.0e+2)-phi_dot.*t26.*t47.*t73.*6.75e-3-phi_dot.*t26.*t73.*t92.*1.05e-2-psi_dot.*t3.*t11.*t16.*2.55e-2-psi_dot.*t3.*t16.*t67.*(2.0./3.75e+2)-psi_dot.*t26.*t31.*t92.*1.05e-2-t11.*t16.*t18.*th32_dot.*(3.0./1.0e+3)+t16.*t18.*t26.*th32_dot.*2.55e-2;
et133 = t11.*t31.*t92.*th32_dot.*(3.0./1.0e+3)-t26.*t31.*t92.*th32_dot.*4.5e-3-t3.*t26.*t31.*zeta_dot.*1.05e-2-t18.*t31.*t67.*zeta_dot.*(2.0./3.75e+2)+t16.*t26.*t92.*zeta_dot.*(3.0./1.0e+3)-t16.*t67.*t92.*zeta_dot.*(2.0./3.75e+2)-phi_dot.*t3.*t16.*t26.*t31.*(3.0./1.0e+3)-phi_dot.*t16.*t18.*t26.*t31.*1.05e-2-psi_dot.*t16.*t18.*t26.*t92.*1.275e-2-t3.*t16.*t18.*t26.*t92.*zeta_dot.*1.05e-2;
et134 = t120+t264-t271+t291-t377+t459-t531+t583+t620+t645+t801-t922+t1098+t1135+t1151+t1180-t1243+t1329+t1401+t1407-t1508-t1586+t1620+t1672+t1748-t1776+t1846-t1922-t1991+t2047+t2055-t2105-t2163+t31.*t321+t3.*t430-psi_dot.*t12.*t31.*(3.0./5.0e+2)+t27.*t31.*th33_dot.*(2.1e+1./1.0e+3)-phi_dot.*t12.*t47.*t73.*(3.0./5.0e+2)-phi_dot.*t27.*t47.*t73.*6.75e-3-psi_dot.*t3.*t12.*t16.*2.55e-2-psi_dot.*t3.*t16.*t68.*(2.0./3.75e+2)-t12.*t16.*t18.*th33_dot.*(3.0./1.0e+3)+t16.*t18.*t27.*th33_dot.*2.55e-2-t12.*t31.*t92.*th33_dot.*(3.0./1.0e+3)+t27.*t31.*t92.*th33_dot.*4.5e-3;
et135 = t3.*t27.*t31.*zeta_dot.*(-1.05e-2)-t18.*t31.*t68.*zeta_dot.*(2.0./3.75e+2)-t16.*t27.*t92.*zeta_dot.*(3.0./1.0e+3)-phi_dot.*t3.*t16.*t27.*t31.*(3.0./1.0e+3)-phi_dot.*t16.*t18.*t27.*t31.*1.05e-2-phi_dot.*t27.*t47.*t73.*t92.*1.05e-2+psi_dot.*t16.*t18.*t27.*t92.*1.275e-2-t3.*t12.*t16.*t92.*th33_dot.*1.05e-2-t3.*t27.*t31.*t92.*zeta_dot.*2.25e-3-(t3.*t12.*t27.*t31.*t92.*zeta_dot)./3.75e+2-phi_dot.*t12.*t16.*t18.*t27.*t31.*t92.*(2.0./3.75e+2);
et136 = t122+t264-t272+t292-t378+t460-t532+t566+t583+t647+t803-t923+t1100+t1136+t1152+t1168+t1181+t1245+t1330-t1510+t1569+t1588+t1673-t1749+t1773+t1777+t1807-t1847+t1923+t1992+t2024+t2048-t2056+t2106+t2164+t31.*t322+t31.*t444+t31.*t1498-psi_dot.*t14.*t31.*(3.0./5.0e+2)+t3.*t92.*t432-t29.*t31.*th42_dot.*(2.1e+1./1.0e+3)-phi_dot.*t14.*t47.*t73.*(3.0./5.0e+2)-phi_dot.*t29.*t47.*t73.*6.75e-3-psi_dot.*t3.*t14.*t16.*2.55e-2-psi_dot.*t3.*t16.*t70.*(2.0./3.75e+2)-t3.*t14.*t16.*th42_dot.*1.05e-2-t14.*t16.*t18.*th42_dot.*(3.0./1.0e+3)+t16.*t18.*t29.*th42_dot.*2.55e-2+t14.*t31.*t92.*th42_dot.*(3.0./1.0e+3);
et137 = t29.*t31.*t92.*th42_dot.*(-4.5e-3)-t18.*t31.*t70.*zeta_dot.*(2.0./3.75e+2)+t16.*t29.*t92.*zeta_dot.*(3.0./1.0e+3)-t16.*t70.*t92.*zeta_dot.*(2.0./3.75e+2)-phi_dot.*t3.*t16.*t29.*t31.*(3.0./1.0e+3)-phi_dot.*t29.*t47.*t73.*t92.*1.05e-2-psi_dot.*t16.*t18.*t29.*t92.*1.275e-2;
et138 = t123+t264-t273+t293-t380+t461-t533+t583+t620+t648+t804+t924+t1101+t1137+t1153+t1169+t1182+t1246+t1401+t1409-t1511+t1589+t1620+t1750-t1778+t1848-t1924-t1993+t2057-t2107+t2139-t2165+t31.*t323+t31.*t445-psi_dot.*t15.*t31.*(3.0./5.0e+2)-t30.*t31.*th43_dot.*(2.1e+1./1.0e+3)-phi_dot.*t15.*t47.*t73.*(3.0./5.0e+2)-phi_dot.*t30.*t47.*t73.*6.75e-3-phi_dot.*t30.*t73.*t92.*1.05e-2-psi_dot.*t3.*t15.*t16.*2.55e-2-psi_dot.*t3.*t16.*t71.*(2.0./3.75e+2)-psi_dot.*t30.*t31.*t92.*1.05e-2-t3.*t15.*t16.*th43_dot.*1.05e-2-t15.*t16.*t18.*th43_dot.*(3.0./1.0e+3)+t16.*t18.*t30.*th43_dot.*2.55e-2;
et139 = t15.*t31.*t92.*th43_dot.*(-3.0./1.0e+3)+t30.*t31.*t92.*th43_dot.*4.5e-3-t18.*t31.*t71.*zeta_dot.*(2.0./3.75e+2)-t16.*t30.*t92.*zeta_dot.*(3.0./1.0e+3)-phi_dot.*t3.*t16.*t30.*t31.*(3.0./1.0e+3)+psi_dot.*t16.*t18.*t30.*t92.*1.275e-2-t3.*t15.*t16.*t92.*th43_dot.*1.05e-2-t3.*t30.*t31.*t92.*zeta_dot.*2.25e-3-t3.*t16.*t18.*t30.*t92.*zeta_dot.*1.05e-2-(t3.*t15.*t30.*t31.*t92.*zeta_dot)./3.75e+2-phi_dot.*t15.*t16.*t18.*t30.*t31.*t92.*(2.0./3.75e+2);
et140 = t213+t215+t217+t219+t221+t223+t225+t227+t229+t231+t233+t235+t252+t255+t258+t261+t414+t415+t416+t417+t418+t419+t420+t421-t422-t423-t424+t425+t426+t427+t428+t429+t430-t431-t432-t433-t474-t475-t476-t477+t514+t515-t516-t517+t518+t519+t520+t521-t546-t547-t548-t549-t550-t551-t552-t553-t554-t555-t556-t557-t558+t559-t560+t561-t562+t563-t564+t565+t599-t608-t609-t610-t611-t612-t613-t614-t615+t649+t650+t651+t652+t729+t730+t731+t732+t765+t766-t767;
et141 = -t768+t781+t782+t783+t784+t785+t786+t787+t788+t789+t790+t791+t792+t853+t856+t859+t862+t933+t943+t944+t945+t946+t947+t948+t949+t950-t994-t995-t996-t997-t998-t999-t1000-t1001+t1010+t1011+t1012+t1013+t1014+t1015+t1016+t1017+t1018+t1019+t1020+t1021+t1022+t1023+t1024+t1025+t1026+t1027+t1028+t1029-t1030-t1031-t1032-t1033+t1078-t1079-t1080+t1081-t1082-t1083+t1084-t1085-t1086+t1087-t1088-t1089+t1102+t1103+t1104+t1105+t1223+t1224+t1225+t1232+t1233+t1234-t1255+t1256+t1257-t1258+t1259+t1260-t1261-t1262+t1263+t1264-t1265-t1266+t1267+t1268+t1269+t1270-t1271-t1272-t1273-t1274+t1290+t1291+t1292+t1293+t1294+t1295+t1299;
et142 = t1300+t1301+t1302+t1303+t1304+t1305+t1306-t1308+t1309-t1310+t1311-t1312+t1313-t1314+t1315+t1348+t1349+t1350+t1351+t1384+t1385+t1386+t1387+t1388+t1389+t1390+t1391+t1414+t1415+t1416+t1417+t1418+t1419+t1420+t1421+t1422+t1423+t1424+t1425+t1426+t1427+t1452+t1453+t1454+t1455+t1456+t1457+t1476-t1477-t1478+t1479-t1480+t1481+t1482-t1483-t1484+t1485-t1486+t1487-t1488+t1489-t1490+t1491+t1516+t1517+t1518+t1519+t1520+t1521+t1522+t1523+t1524+t1525+t1526+t1527+t1528+t1529+t1530+t1531+t1557+t1558+t1559-t1560-t1561-t1562-t1563-t1564-t1565+t1566+t1567+t1568+t1607+t1621-t1622+t1623-t1624+t1626+t1628+t1650-t1651+t1652+t1653-t1654+t1655-t1656-t1657+t1658+t1699+t1700+t1701+t1702+t1703+t1704+t1705+t1706+t1707+t1708+t1709+t1710+t1825+t1827+t1829+t1831+t1833+t1835+t1837+t1839+t1857;
et143 = t1859+t1861+t1863+t1894+t1895+t1897+t1900+t1901+t1903+t1905+t1907+t1925+t1926+t1927+t1928+t1929+t1930+t1931+t1932+t1942+t1944+t1946+t1948+t1950+t1951+t1952+t1953+t1954+t1957+t1959+t1960+t1978+t1980+t1982+t1984+t2011+t2013+t2015+t2017+t2058+t2059+t2060+t2061+t2062+t2063+t2064+t2065+t2066+t2067+t2068+t2069+t2071+t2072+t2073+t2074+t2075+t2076+t2077+t2078+t2079-t2080+t2081-t2082+t2083-t2084+t2085-t2086+t2087-t2088+t2089-t2090+t2091-t2092+t2093-t2094+t2095+t2096+t2097+t2098+t2116+t2119+t2121+t2122+t2140-t2141+t2142-t2143+t2144-t2145+t2146-t2147+t2166+t2168+t2170+t2172+t3.*t212+t3.*t218+t3.*t224+t3.*t230+t3.*t31.*t169+t3.*t31.*t170+t3.*t31.*t171+t3.*t31.*t172+t18.*t92.*t216+t18.*t92.*t222-(t18.*t31.*th12_dot)./3.75e+2-(t18.*t31.*th13_dot)./3.75e+2-(t18.*t31.*th22_dot)./3.75e+2;
et144 = t18.*t31.*th23_dot.*(-1.0./3.75e+2)-(t18.*t31.*th32_dot)./3.75e+2-(t18.*t31.*th33_dot)./3.75e+2-(t18.*t31.*th42_dot)./3.75e+2-(t18.*t31.*th43_dot)./3.75e+2-phi_dot.*t19.*t46.*t87.*(3.0./1.0e+3)-phi_dot.*t20.*t46.*t87.*(3.0./1.0e+3)-phi_dot.*t21.*t46.*t87.*(3.0./1.0e+3)-phi_dot.*t22.*t46.*t87.*(3.0./1.0e+3)-phi_dot.*t23.*t46.*t87.*(3.0./1.0e+3)-phi_dot.*t24.*t46.*t87.*(3.0./1.0e+3)-phi_dot.*t25.*t46.*t87.*(3.0./1.0e+3)-phi_dot.*t26.*t46.*t87.*(3.0./1.0e+3)-phi_dot.*t27.*t46.*t87.*(3.0./1.0e+3)-phi_dot.*t28.*t46.*t87.*(3.0./1.0e+3)-phi_dot.*t29.*t46.*t87.*(3.0./1.0e+3)-phi_dot.*t30.*t46.*t87.*(3.0./1.0e+3);
et145 = psi_dot.*t3.*t5.*t31.*(-3.0./1.0e+3)-psi_dot.*t3.*t6.*t31.*(3.0./1.0e+3)-psi_dot.*t3.*t8.*t31.*(3.0./1.0e+3)-psi_dot.*t3.*t9.*t31.*(3.0./1.0e+3)-psi_dot.*t3.*t11.*t31.*(3.0./1.0e+3)-psi_dot.*t3.*t12.*t31.*(3.0./1.0e+3)-psi_dot.*t3.*t14.*t31.*(3.0./1.0e+3)-psi_dot.*t3.*t15.*t31.*(3.0./1.0e+3)+psi_dot.*t3.*t19.*t31.*(3.0./1.0e+2)-psi_dot.*t4.*t18.*t31.*(2.1e+1./1.0e+3)+psi_dot.*t3.*t20.*t31.*1.65e-2+psi_dot.*t5.*t18.*t31.*1.05e-2+psi_dot.*t3.*t21.*t31.*1.65e-2+psi_dot.*t6.*t18.*t31.*1.05e-2+psi_dot.*t3.*t22.*t31.*(3.0./1.0e+2)+psi_dot.*t7.*t18.*t31.*(2.1e+1./1.0e+3);
et146 = psi_dot.*t3.*t23.*t31.*1.65e-2-psi_dot.*t8.*t18.*t31.*1.05e-2+psi_dot.*t3.*t24.*t31.*1.65e-2-psi_dot.*t9.*t18.*t31.*1.05e-2-psi_dot.*t3.*t25.*t31.*(3.0./2.5e+2)+psi_dot.*t10.*t18.*t31.*(2.1e+1./1.0e+3)-psi_dot.*t3.*t26.*t31.*2.55e-2-psi_dot.*t11.*t18.*t31.*1.05e-2-psi_dot.*t3.*t27.*t31.*2.55e-2-psi_dot.*t12.*t18.*t31.*1.05e-2-psi_dot.*t3.*t28.*t31.*(3.0./2.5e+2)-psi_dot.*t13.*t18.*t31.*(2.1e+1./1.0e+3)-psi_dot.*t3.*t29.*t31.*2.55e-2+psi_dot.*t14.*t18.*t31.*1.05e-2-psi_dot.*t3.*t30.*t31.*2.55e-2+psi_dot.*t15.*t18.*t31.*1.05e-2;
et147 = psi_dot.*t3.*t31.*t76.*(-1.0./3.75e+2)-(psi_dot.*t3.*t31.*t77)./3.75e+2-(psi_dot.*t3.*t31.*t79)./3.75e+2-(psi_dot.*t3.*t31.*t80)./3.75e+2-(psi_dot.*t3.*t31.*t82)./3.75e+2-(psi_dot.*t3.*t31.*t83)./3.75e+2-(psi_dot.*t3.*t31.*t85)./3.75e+2-(psi_dot.*t3.*t31.*t86)./3.75e+2+t4.*t18.*t31.*th11_dot.*(3.0./1.0e+2)+t5.*t18.*t31.*th12_dot.*1.65e-2+t6.*t18.*t31.*th13_dot.*1.65e-2+t7.*t18.*t31.*th21_dot.*(3.0./1.0e+2)+t8.*t18.*t31.*th22_dot.*1.65e-2+t9.*t18.*t31.*th23_dot.*1.65e-2-t10.*t18.*t31.*th31_dot.*(3.0./2.5e+2)-t11.*t18.*t31.*th32_dot.*2.55e-2-t12.*t18.*t31.*th33_dot.*2.55e-2;
et148 = t13.*t18.*t31.*th41_dot.*(-3.0./2.5e+2)-t14.*t18.*t31.*th42_dot.*2.55e-2-t15.*t18.*t31.*th43_dot.*2.55e-2-phi_dot.*t5.*t18.*t72.*t92.*(3.0./5.0e+2)-phi_dot.*t8.*t18.*t72.*t92.*(3.0./5.0e+2)-phi_dot.*t6.*t46.*t87.*t92.*5.25e-3-phi_dot.*t8.*t46.*t87.*t92.*5.25e-3-phi_dot.*t11.*t46.*t87.*t92.*5.25e-3-phi_dot.*t15.*t46.*t87.*t92.*5.25e-3-(phi_dot.*t74.*t77.*t87.*t92)./7.5e+2-(phi_dot.*t74.*t80.*t87.*t92)./7.5e+2-(phi_dot.*t74.*t83.*t87.*t92)./7.5e+2-(phi_dot.*t74.*t86.*t87.*t92)./7.5e+2-psi_dot.*t5.*t18.*t31.*t92.*(3.0./5.0e+2)-psi_dot.*t8.*t18.*t31.*t92.*(3.0./5.0e+2);
et149 = psi_dot.*t11.*t18.*t31.*t92.*(3.0./2.0e+2)-psi_dot.*t12.*t18.*t31.*t92.*(3.0./2.0e+2)+psi_dot.*t14.*t18.*t31.*t92.*(3.0./2.0e+2)-psi_dot.*t15.*t18.*t31.*t92.*(3.0./2.0e+2)+(psi_dot.*t18.*t31.*t49.*t92)./7.5e+2-(psi_dot.*t18.*t31.*t50.*t92)./7.5e+2+(psi_dot.*t18.*t31.*t52.*t92)./7.5e+2-(psi_dot.*t18.*t31.*t53.*t92)./7.5e+2+(psi_dot.*t18.*t31.*t55.*t92)./7.5e+2-(psi_dot.*t18.*t31.*t56.*t92)./7.5e+2+(psi_dot.*t18.*t31.*t58.*t92)./7.5e+2-(psi_dot.*t18.*t31.*t59.*t92)./7.5e+2-t3.*t20.*t31.*t92.*th12_dot.*8.25e-3+t3.*t21.*t31.*t92.*th13_dot.*8.25e-3-t3.*t23.*t31.*t92.*th22_dot.*8.25e-3+t3.*t24.*t31.*t92.*th23_dot.*8.25e-3;
et150 = t3.*t26.*t31.*t92.*th32_dot.*1.275e-2-t3.*t27.*t31.*t92.*th33_dot.*1.275e-2+t3.*t29.*t31.*t92.*th42_dot.*1.275e-2-t3.*t30.*t31.*t92.*th43_dot.*1.275e-2;
et151 = psi_dot.*t74.*3.085625e-1+t4.*th11_dot.*(3.0./1.0e+3)+t5.*th12_dot.*(3.0./1.0e+3)+t6.*th13_dot.*(3.0./1.0e+3)+t7.*th21_dot.*(3.0./1.0e+3)+t8.*th22_dot.*(3.0./1.0e+3)-t19.*th11_dot.*(3.0./1.0e+2)+t9.*th23_dot.*(3.0./1.0e+3)+t20.*th12_dot.*4.875e-3+t21.*th13_dot.*4.875e-3+t10.*th31_dot.*(3.0./1.0e+3)+t11.*th32_dot.*(3.0./1.0e+3)-t22.*th21_dot.*(3.0./1.0e+2)+t12.*th33_dot.*(3.0./1.0e+3)+t23.*th22_dot.*4.875e-3+t24.*th23_dot.*4.875e-3+t13.*th41_dot.*(3.0./1.0e+3)+t14.*th42_dot.*(3.0./1.0e+3)+t25.*th31_dot.*(3.0./2.5e+2)+t15.*th43_dot.*(3.0./1.0e+3)-t26.*th32_dot.*1.6125e-2;
